simulink model "SIM_EXO_DAL_MN"  (R2021b)
(part 14 of 24)

C_dq = ft_12({dq1,dq2,dq3,dq4,dq5,dq6,t1004,t1016,t1019,t1020,t1031,t1039,t1046,t1050,t1056,t1061,t1069,t1075,t1076,t1077,t1081,t1083,t1088,t1090,t1095,t1099,t1101,t1106,t1108,t112,t1122,t113,t1133,t1144,t1146,t1147,t115,t1150,t1152,t1155,t1156,t1158,t116,t1165,t1170,t1171,t1174,t1177,t1179,t1184,t1185,t1191,t1193,t1194,t1196,t1201,t1203,t1205,t1207,t121,t1211,t1212,t1213,t1215,t1221,t1224,t1225,t1227,t1228,t1233,t1245,t125,t1250,t1253,t1254,t1258,t1265,t1267,t1268,t1269,t1273,t1274,t1282,t1285,t1288,t1292,t1300,t1301,t1306,t131,t1311,t1316,t1317,t1318,t132,t1322,t1323,t1324,t133,t1330,t1331,t1333,t1337,t1342,t1344,t1345,t1348,t1353,t1365,t1377,t1379,t1380,t1383,t1388,t139,t1391,t1402,t1407,t1409,t1411,t1413,t1419,t142,t1423,t1426,t1427,t1428,t1429,t1436,t144,t1440,t1441,t1443,t1445,t1446,t1449,t1454,t1457,t1458,t1460,t1471,t148,t1486,t1487,t1488,t1489,t1493,t1494,t1495,t1496,t1498,t1499,t15,t150,t1503,t1505,t1506,t1508,t151,t1511,t1517,t1520,t1521,t1522,t1523,t1524,t1526,t1530,t1531,t1533,t1534,t1535,t1536,t1537,t1538,t1540,t1541,t1542,t1548,t1549,t1550,t1551,t1558,t156,t1560,t1561,t1566,t1567,t1568,t1570,t1571,t1574,t1577,t1578,t158,t1581,t1582,t1584,t1585,t1586,t1587,t1589,t1590,t1591,t1592,t1593,t1594,t1595,t1598,t16,t1600,t1601,t1602,t1605,t1606,t1607,t1609,t1611,t1612,t1613,t1614,t1615,t1616,t1617,t1619,t1620,t1621,t1622,t1625,t1627,t1628,t1630,t1632,t1633,t1635,t1636,t1637,t1638,t1639,t1641,t1642,t1643,t1644,t1645,t1647,t1648,t1651,t1653,t1655,t1656,t1657,t1658,t1659,t166,t1660,t1661,t1662,t1663,t1666,t1667,t1669,t1670,t1672,t1674,t1676,t1681,t1683,t1687,t1692,t1696,t1697,t1699,t17,t1700,t1701,t1704,t1705,t1706,t1707,t1708,t1709,t171,t1710,t1711,t1712,t1713,t1715,t1716,t1718,t1719,t1720,t1721,t1724,t1728,t1729,t1731,t1732,t1733,t1734,t1735,t1736,t1740,t1745,t1747,t1748,t1752,t1753,t1754,t1755,t1756,t1757,t1758,t1759,t1760,t1761,t1762,t1763,t1764,t1766,t1767,t1769,t1770,t1771,t1772,t1775,t1776,t1777,t1779,t1781,t1783,t1784,t1785,t1786,t1787,t1788,t1789,t1792,t1793,t1794,t1795,t1797,t1798,t1799,t18,t1800,t1804,t1805,t1806,t1807,t1808,t1809,t1811,t1812,t1814,t1815,t1816,t1820,t1821,t1823,t1827,t1828,t1829,t183,t1831,t1832,t1833,t1834,t1835,t1836,t1839,t1847,t1849,t185,t1850,t1851,t1855,t1856,t1857,t1858,t1859,t1860,t1861,t1863,t1866,t1867,t1868,t1870,t1873,t1878,t1882,t1884,t1886,t1889,t1892,t1896,t1899,t19,t190,t1900,t1902,t1903,t1906,t1907,t1908,t1909,t191,t1912,t1913,t1915,t1916,t1917,t1920,t1922,t1925,t1926,t1930,t1935,t1936,t1937,t1938,t1939,t1941,t1942,t1943,t1946,t1947,t1951,t1952,t1955,t196,t1961,t1967,t1968,t1969,t197,t1970,t1974,t1977,t1981,t1983,t1984,t1985,t1986,t1989,t199,t1992,t1993,t1994,t1995,t1996,t1997,t1998,t1999,t2,t20,t200,t2000,t2002,t2003,t2004,t2006,t2008,t201,t2014,t2015,t2017,t2019,t202,t2020,t2026,t2027,t2028,t2033,t2034,t2035,t2036,t2037,t2038,t2039,t2042,t2043,t2047,t2050,t2052,t2053,t206,t2060,t2062,t2066,t2067,t2068,t2069,t207,t2070,t2072,t2073,t2075,t2076,t2077,t2079,t2081,t2083,t2084,t2085,t2087,t2088,t2091,t2096,t2098,t21,t2100,t2104,t2105,t2106,t2108,t2110,t2113,t2114,t2115,t2116,t2118,t2119,t2121,t2123,t2128,t2130,t2131,t2132,t2133,t2134,t2136,t2142,t2143,t2145,t2148,t2149,t2150,t2154,t2158,t2164,t2165,t2171,t2176,t2177,t2178,t2180,t2181,t2182,t2184,t2186,t2187,t2189,t2191,t2192,t2193,t2194,t2196,t2197,t2199,t22,t2200,t2202,t2203,t2208,t2211,t2212,t2213,t2214,t2217,t2218,t2220,t2223,t2224,t2225,t2234,t2236,t2239,t224,t2243,t225,t2253,t2256,t2257,t2265,t2266,t2267,t227,t2276,t2277,t2279,t228,t2280,t2284,t2285,t2289,t2291,t2296,t2298,t2299,t23,t230,t2300,t2303,t2304,t2305,t231,t2312,t2314,t2315,t2316,t2317,t2320,t2323,t2324,t2326,t2328,t233,t2330,t2333,t2334,t2336,t2338,t2339,t234,t2340,t2341,t2342,t235,t2350,t2357,t2358,t2359,t236,t2361,t2362,t2364,t2369,t2372,t2375,t2376,t2377,t2379,t2383,t2385,t2387,t2388,t2389,t2390,t2391,t2392,t2394,t2395,t2396,t2397,t2398,t24,t240,t2400,t2401,t2402,t2403,t2405,t2406,t2410,t2416,t2417,t2420,t2421,t2424,t2429,t243,t2430,t2431,t2435,t2438,t2439,t244,t2440,t2441,t2443,t2444,t2449,t2452,t2453,t2454,t2455,t2456,t2465,t2466,t2470,t2474,t2481,t2483,t2486,t249,t2490,t2494,t2497,t2502,t2507,t2513,t2519,t2523,t2524,t2525,t2530,t2539,t2544,t2545,t2546,t2548,t2549,t2552,t2553,t2554,t2555,t2556,t2560,t2562,t2563,t2564,t2565,t2566,t2567,t2568,t2569,t257,t2570,t2571,t2574,t2575,t2576,t2577,t2578,t2579,t258,t2588,t2589,t2597,t2598,t2599,t2606,t2611,t2612,t2615,t2617,t2620,t2623,t2624,t2625,t2627,t263,t2633,t2634,t2639,t2640,t2641,t2644,t2649,t2650,t2651,t2655,t2656,t2659,t266,t2666,t2669,t2671,t2673,t2675,t2681,t2684,t2686,t2689,t2691,t2692,t2694,t2695,t2696,t2697,t2698,t270,t2700,t2706,t2707,t2708,t2711,t2713,t2714,t2715,t2718,t2720,t2721,t2722,t2724,t2725,t2726,t273,t2736,t2737,t274,t2740,t2741,t2743,t2744,t2748,t2749,t275,t2750,t2752,t2753,t2754,t2755,t2757,t2758,t2759,t276,t2760,t2761,t2762,t2764,t277,t2770,t2771,t2772,t2775,t2778,t278,t2780,t2783,t2785,t2791,t2792,t2793,t2795,t2796,t2797,t2798,t2799,t280,t2800,t2801,t2802,t2805,t2806,t2807,t2812,t2814,t2815,t2816,t2817,t2818,t2824,t2825,t2827,t2828,t2832,t2833,t2835,t284,t2850,t2851,t2854,t2857,t2861,t2868,t287,t2872,t2877,t2880,t2881,t2883,t2884,t2887,t2889,t2893,t2895,t2896,t29,t290,t2905,t2906,t2907,t291,t2911,t2912,t2913,t2915,t2916,t2918,t292,t2921,t2922,t2932,t2933,t294,t2941,t2944,t2946,t2956,t2958,t2965,t297,t2973,t2977,t2987,t299,t2993,t2998,t2999,t3,t30,t300,t302,t303,t304,t3047,t305,t306,t3065,t3080,t3083,t3088,t309,t3095,t3096,t310,t311,t3117,t3125,t3129,t313,t3136,t314,t3142,t315,t3159,t316,t3164,t3166,t3168,t318,t319,t320,t3200,t3209,t3210,t3213,t3219,t322,t3222,t3223,t3224,t3228,t3230,t3239,t324,t3245,t3247,t325,t3266,t3268,t3274,t3275,t3277,t3278,t3279,t328,t3284,t3288,t3296,t3298,t3303,t3309,t3314,t3317,t3318,t3320,t3321,t3326,t3328,t3329,t333,t3332,t3336,t3337,t3338,t3340,t3349,t3351,t3352,t3353,t336,t3363,t3364,t3365,t3366,t3368,t3369,t337,t3371,t3372,t3373,t3375,t3377,t3378,t3380,t3381,t3383,t3387,t3388,t3390,t3391,t3392,t3393,t3396,t3397,t3398,t3399,t34,t340,t3400,t3402,t3405,t3407,t3408,t3409,t3410,t3411,t3413,t3416,t3417,t3418,t3420,t3421,t3422,t3426,t3429,t3430,t3432,t3434,t3435,t3436,t3437,t3439,t344,t3440,t3441,t3442,t3443,t3444,t3445,t3446,t3447,t3449,t3450,t3453,t3454,t3455,t3457,t3458,t346,t3462,t3463,t3464,t3465,t3468,t3469,t347,t3471,t3472,t3473,t3474,t3475,t3476,t3479,t348,t3480,t3481,t3483,t3484,t3485,t3489,t349,t3490,t3491,t3492,t3493,t3496,t3498,t3499,t350,t3500,t3501,t3502,t3504,t3505,t3506,t3507,t3510,t3511,t3513,t3514,t3515,t3517,t3518,t352,t3521,t3522,t3523,t3526,t353,t3530,t3531,t3532,t3535,t3536,t3539,t3540,t3542,t3543,t3544,t3547,t3554,t3556,t3557,t3559,t356,t3562,t3563,t3565,t3568,t3569,t357,t3571,t3572,t3573,t3574,t3577,t3578,t358,t3582,t3583,t3584,t3585,t3588,t3589,t359,t3590,t3591,t3592,t3593,t3598,t3602,t3604,t3605,t3606,t3607,t361,t3610,t3611,t3612,t3617,t3618,t362,t3624,t3625,t3633,t3634,t3635,t3636,t3637,t3638,t3640,t3642,t3644,t3648,t365,t3652,t3653,t3654,t3655,t3656,t3657,t3658,t3659,t3662,t3666,t3667,t3668,t3671,t3672,t3673,t3674,t3676,t3678,t3679,t368,t3681,t3682,t3689,t369,t3690,t3691,t3693,t3694,t3696,t3698,t3699,t3700,t3701,t3702,t3703,t3704,t3705,t3706,t3708,t371,t3713,t3715,t3717,t3719,t372,t3720,t3725,t3726,t3728,t3729,t373,t3731,t3732,t3733,t3734,t3735,t3737,t3738,t374,t3742,t3743,t3746,t3747,t3750,t3752,t3753,t3754,t3755,t3756,t3757,t3758,t3759,t3761,t3762,t3763,t3764,t3765,t3766,t3767,t3769,t377,t3772,t3777,t3779,t378,t3780,t3781,t3783,t3784,t3785,t3787,t3788,t3789,t379,t3792,t3793,t3795,t3796,t3799,t380,t3800,t3810,t3811,t3812,t3813,t3814,t3815,t3818,t3819,t382,t3820,t3821,t3822,t3823,t3824,t3831,t3833,t3834,t3835,t3836,t3838,t3839,t384,t3840,t3841,t3842,t3843,t3844,t3845,t3848,t3849,t3851,t3852,t3853,t386,t3863,t3865,t3866,t3868,t3869,t387,t3870,t3871,t3872,t3873,t3874,t3875,t3876,t388,t3880,t3882,t3883,t3884,t3885,t3889,t3890,t3891,t3892,t3893,t3896,t3904,t3905,t3906,t3907,t3908,t391,t3910,t3913,t3914,t3915,t392,t3920,t3921,t3922,t3923,t3924,t3931,t3940,t3941,t3942,t3943,t3944,t395,t3950,t3951,t3954,t3955,t3956,t3957,t3959,t396,t3960,t3965,t3967,t3968,t3969,t3971,t3972,t3973,t3976,t3977,t3978,t3979,t3991,t3992,t3993,t3995,t3996,t3997,t3998,t4,t400,t4000,t4004,t4008,t401,t4010,t4011,t4014,t4015,t4016,t4017,t4018,t402,t4020,t4023,t4024,t4025,t4026,t4028,t4029,t403,t4034,t4037,t4041,t4042,t4045,t4046,t4047,t4050,t4051,t4053,t4055,t4056,t4057,t4059,t406,t4062,t4063,t4064,t4067,t4068,t4069,t4070,t4071,t4072,t4073,t4074,t4075,t4076,t4079,t4080,t4083,t4085,t4086,t4087,t4088,t4089,t4091,t4092,t4093,t4094,t4095,t4096,t4099,t410,t4100,t4102,t4103,t4104,t4108,t411,t4113,t4115,t4118,t4119,t412,t4121,t4122,t4123,t4126,t4127,t413,t4132,t4134,t4138,t414,t4141,t4143,t4146,t4148,t4149,t415,t4152,t4153,t4154,t4158,t416,t4161,t4166,t417,t4173,t4178,t4179,t418,t4181,t4183,t4184,t4185,t4186,t4190,t4196,t4197,t4198,t4199,t420,t4205,t4206,t4208,t4209,t4210,t4211,t4215,t4217,t4218,t4219,t422,t4221,t4223,t4224,t4226,t4228,t423,t4230,t4231,t4232,t4233,t4234,t4235,t424,t4241,t4243,t4245,t4246,t4247,t4248,t4249,t425,t4250,t4251,t4254,t4255,t4256,t4257,t4259,t4260,t4261,t4262,t4263,t427,t4274,t4276,t4278,t4279,t428,t4280,t4282,t4283,t4284,t4285,t4286,t4287,t4289,t429,t4290,t4292,t4293,t4295,t4296,t4297,t4298,t4299,t4301,t4303,t4304,t4305,t4306,t431,t4315,t4317,t4318,t432,t4323,t4324,t4325,t4326,t4327,t4329,t433,t4330,t4332,t4333,t4334,t4335,t4337,t4338,t4339,t434,t4342,t4344,t4345,t4346,t4347,t4348,t4349,t435,t4350,t436,t4363,t4365,t4366,t4368,t4369,t437,t4370,t4371,t4373,t4374,t4377,t4378,t438,t4380,t4382,t4383,t4385,t4387,t4388,t439,t4392,t4394,t4395,t4396,t4397,t4399,t44,t440,t4402,t4403,t4405,t4406,t4407,t4409,t441,t4410,t4412,t4413,t4414,t4416,t4417,t4418,t4419,t442,t4420,t4421,t4423,t4425,t4426,t4427,t4428,t4429,t4431,t4432,t4433,t4434,t4435,t4436,t4437,t4438,t4439,t444,t4440,t4444,t4446,t4447,t4449,t445,t4450,t4453,t4460,t4462,t4463,t4464,t4467,t4468,t4469,t4470,t4471,t4473,t4474,t4475,t4478,t4479,t448,t4482,t4483,t4484,t4485,t4486,t4487,t4488,t4489,t449,t4490,t4494,t4495,t4498,t4499,t45,t450,t4500,t4501,t4502,t4503,t4504,t4505,t4506,t4507,t4508,t4509,t4510,t4512,t4515,t4518,t4519,t452,t4520,t4521,t4522,t4523,t4526,t4527,t4528,t453,t4530,t4534,t4536,t4538,t4539,t454,t4541,t4543,t4545,t4546,t4549,t4551,t4552,t4553,t4556,t4557,t4558,t4559,t4560,t4565,t4568,t4569,t457,t4570,t4572,t4575,t4577,t4578,t458,t4581,t4582,t4586,t4587,t4588,t4589,t459,t4590,t4591,t4592,t4593,t4595,t4596,t4597,t4598,t460,t4600,t4601,t4602,t4604,t4605,t4606,t4607,t4608,t461,t4614,t4616,t4619,t462,t4621,t4622,t4623,t4624,t4625,t4626,t4629,t463,t4633,t4634,t4636,t4637,t4639,t464,t4640,t4644,t4645,t4647,t4648,t465,t4650,t4652,t4653,t4654,t4656,t4657,t4659,t466,t4660,t4662,t4663,t4666,t4667,t4668,t4669,t4670,t4673,t4674,t4675,t4677,t4678,t4679,t468,t4680,t4681,t4682,t4683,t4684,t4685,t4686,t4687,t469,t4694,t4695,t4696,t4697,t4699,t47,t470,t4700,t4703,t4707,t4708,t4709,t471,t4711,t4714,t4717,t4718,t4719,t472,t4720,t4721,t4722,t4723,t4724,t4725,t4726,t4727,t4728,t4731,t4732,t4733,t4734,t4737,t4738,t4739,t4742,t4743,t4745,t4747,t4748,t475,t4754,t4755,t4756,t4762,t4763,t4764,t4767,t477,t4772,t4773,t4775,t4780,t4781,t4782,t4783,t4785,t4786,t479,t480,t4803,t481,t4810,t4811,t482,t4824,t4825,t4826,t483,t4831,t4837,t4838,t4842,t4846,t485,t486,t4862,t4864,t4865,t4866,t4867,t4869,t4870,t4877,t488,t4884,t489,t4903,t4904,t491,t4911,t4914,t4919,t492,t4920,t4922,t4924,t4925,t4927,t4929,t493,t4934,t4936,t494,t4942,t4944,t4946,t4949,t4950,t4952,t4953,t4957,t496,t4964,t4966,t4967,t4969,t497,t4973,t4974,t4979,t498,t4981,t4982,t4983,t4984,t4987,t4988,t4989,t499,t4990,t4993,t4994,t4995,t4996,t5,t50,t500,t5000,t5001,t5002,t5007,t5008,t5009,t501,t5016,t5017,t502,t5020,t5021,t5022,t5023,t5024,t5026,t5027,t503,t5031,t5032,t5039,t504,t5043,t5049,t505,t5050,t5056,t5058,t506,t5061,t5063,t5064,t5065,t507,t5074,t5075,t5076,t508,t5080,t5083,t5084,t5086,t5087,t509,t5090,t5091,t5092,t5093,t5097,t5098,t5099,t510,t5100,t5102,t5107,t511,t5110,t5112,t5113,t5114,t512,t5121,t5123,t513,t5131,t5132,t5136,t5139,t514,t5140,t5143,t5144,t5145,t5147,t5148,t5150,t5151,t516,t5163,t5164,t5166,t5167,t517,t5175,t5177,t518,t5182,t5184,t5188,t5189,t5194,t5195,t520,t5200,t5202,t5203,t5204,t5205,t5206,t521,t5210,t5211,t5215,t5217,t5219,t522,t5222,t5227,t5228,t523,t5231,t5232,t5233,t5235,t5236,t5237,t5238,t524,t5242,t5244,t5249,t525,t5251,t5252,t5254,t5255,t5256,t5258,t5259,t526,t5260,t5261,t5262,t5264,t5266,t5269,t527,t5275,t5279,t528,t5280,t5285,t5286,t529,t5291,t5294,t5296,t5297,t5299,t53,t530,t5301,t5302,t5307,t5309,t531,t5314,t5316,t5318,t532,t5320,t5321,t5322,t5323,t5324,t533,t5333,t5335,t5337,t5339,t534,t5340,t5344,t535,t5354,t5356,t5357,t5358,t5359,t536,t5361,t5364,t5369,t537,t5370,t5371,t5372,t5373,t5375,t5378,t5379,t538,t5380,t5381,t5382,t5383,t5385,t5389,t539,t5390,t5391,t5392,t5393,t5394,t5395,t5396,t5397,t5399,t540,t5401,t5402,t5403,t5404,t5405,t5406,t5408,t5409,t5410,t5411,t5412,t5414,t5415,t5416,t5418,t5422,t5423,t5426,t5427,t5428,t543,t5431,t5436,t5438,t544,t5442,t5443,t5447,t545,t5450,t5451,t5457,t5459,t546,t5464,t5465,t5466,t547,t5479,t548,t5480,t5482,t5483,t5484,t5486,t5487,t5488,t549,t5507,t551,t5512,t5515,t552,t5521,t5526,t553,t554,t555,t556,t557,t558,t559,t560,t5602,t5605,t561,t5616,t5617,t5619,t562,t5620,t5621,t5622,t5623,t5624,t5625,t5626,t5628,t563,t5630,t5633,t5634,t5636,t5639,t564,t5642,t5644,t5648,t5657,t5658,t5662,t5665,t5666,t567,t5670,t5679,t568,t5682,t5684,t5688,t569,t5691,t5692,t5694,t5696,t5698,t5699,t57,t570,t5701,t5703,t5704,t5705,t5707,t571,t5711,t5713,t5714,t5718,t572,t5720,t5722,t5723,t5724,t5726,t5727,t5728,t573,t5731,t5732,t5733,t5736,t5738,t574,t5742,t5745,t5746,t5747,t5748,t5751,t5754,t5757,t5759,t576,t5760,t5763,t5765,t5768,t5770,t5771,t5772,t5773,t5774,t5775,t5776,t5778,t5779,t578,t5782,t5784,t5786,t5787,t5788,t579,t5790,t5792,t5794,t5795,t5797,t58,t580,t5808,t5809,t581,t5810,t5813,t5814,t5818,t5819,t582,t5822,t5823,t5824,t5825,t5826,t5827,t5828,t5829,t5830,t5831,t5832,t5833,t5834,t5835,t5836,t5838,t584,t5842,t5843,t5844,t5845,t5846,t5849,t5850,t5851,t5852,t5859,t586,t5860,t5861,t5862,t5863,t5868,t5869,t587,t5870,t5871,t5872,t5873,t5874,t5875,t5876,t5881,t5882,t5883,t5884,t5885,t5886,t5887,t5888,t5889,t589,t5890,t5891,t5892,t5893,t5894,t5895,t5896,t5898,t5899,t590,t5901,t5902,t5903,t5905,t5906,t5909,t591,t5917,t5918,t5919,t592,t5920,t5925,t5928,t593,t5930,t5931,t5932,t5933,t5934,t5935,t5936,t5938,t5939,t594,t5940,t595,t5954,t5956,t5957,t5958,t5959,t596,t5960,t5964,t5965,t5966,t5967,t597,t5970,t5971,t5972,t5976,t5977,t5978,t5979,t5980,t5981,t5982,t5984,t5988,t5994,t5996,t5998,t5999,t6,t60,t600,t6000,t6001,t6002,t6003,t6005,t6007,t6011,t6012,t6013,t6014,t6017,t602,t603,t6038,t604,t6043,t6045,t6046,t6047,t605,t6060,t6061,t6062,t6064,t6065,t6069,t6075,t6077,t6079,t6086,t609,t610,t6101,t6102,t6103,t6105,t6106,t6108,t6109,t611,t6117,t6119,t612,t6123,t6124,t6126,t613,t6136,t6139,t614,t6140,t6149,t615,t616,t618,t619,t6195,t620,t6203,t6204,t6205,t6206,t6209,t621,t6210,t622,t623,t624,t625,t626,t629,t6319,t632,t6329,t6330,t6338,t6341,t6342,t6343,t6347,t6348,t6349,t6350,t6351,t6352,t6362,t638,t6391,t6395,t640,t6403,t6416,t6417,t6436,t6437,t6462,t6463,t6471,t650,t6506,t654,t6565,t658,t6597,t6609,t6689,t669,t6690,t673,t679,t681,t6826,t6827,t683,t684,t7,t7012,t7020,t7043,t705,t706,t7079,t708,t7080,t7087,t71,t7104,t7119,t712,t7148,t7149,t716,t72,t724,t7256,t73,t731,t733,t7333,t7364,t738,t739,t741,t742,t743,t744,t746,t748,t749,t75,t750,t752,t7528,t753,t7549,t7553,t7556,t7566,t7570,t7573,t759,t76,t760,t764,t765,t766,t773,t777,t778,t779,t780,t781,t784,t785,t792,t796,t797,t8,t801,t802,t803,t804,t81,t823,t824,t825,t826,t827,t830,t832,t833,t834,t835,t836,t838,t84,t841,t842,t843,t845,t846,t847,t848,t852,t856,t86,t861,t863,t866,t868,t869,t870,t874,t875,t877,t878,t880,t881,t893,t899,t9,t90,t902,t903,t905,t908,t909,t91,t910,t911,t912,t914,t915,t917,t919,t922,t925,t926,t928,t929,t930,t931,t932,t934,t940,t944,t945,t947,t95,t952,t954,t955,t957,t958,t968,t97,t970,t971,t972,t975,t976,t984,t985,t986,t989,t99,t991,t998});
end
function C_dq = ft_12(ct)
dq1 = ct{1};
dq2 = ct{2};
dq3 = ct{3};
dq4 = ct{4};
dq5 = ct{5};
dq6 = ct{6};
t1004 = ct{7};
t1016 = ct{8};
t1019 = ct{9};
t1020 = ct{10};
t1031 = ct{11};
t1039 = ct{12};
t1046 = ct{13};
t1050 = ct{14};
t1056 = ct{15};
t1061 = ct{16};
t1069 = ct{17};
t1075 = ct{18};
t1076 = ct{19};
t1077 = ct{20};
t1081 = ct{21};
t1083 = ct{22};
t1088 = ct{23};
t1090 = ct{24};
t1095 = ct{25};
t1099 = ct{26};
t1101 = ct{27};
t1106 = ct{28};
t1108 = ct{29};
t112 = ct{30};
t1122 = ct{31};
t113 = ct{32};
t1133 = ct{33};
t1144 = ct{34};
t1146 = ct{35};
t1147 = ct{36};
t115 = ct{37};
t1150 = ct{38};
t1152 = ct{39};
t1155 = ct{40};
t1156 = ct{41};
t1158 = ct{42};
t116 = ct{43};
t1165 = ct{44};
t1170 = ct{45};
t1171 = ct{46};
t1174 = ct{47};
t1177 = ct{48};
t1179 = ct{49};
t1184 = ct{50};
t1185 = ct{51};
t1191 = ct{52};
t1193 = ct{53};
t1194 = ct{54};
t1196 = ct{55};
t1201 = ct{56};
t1203 = ct{57};
t1205 = ct{58};
t1207 = ct{59};
t121 = ct{60};
t1211 = ct{61};
t1212 = ct{62};
t1213 = ct{63};
t1215 = ct{64};
t1221 = ct{65};
t1224 = ct{66};
t1225 = ct{67};
t1227 = ct{68};
t1228 = ct{69};
t1233 = ct{70};
t1245 = ct{71};
t125 = ct{72};
t1250 = ct{73};
t1253 = ct{74};
t1254 = ct{75};
t1258 = ct{76};
t1265 = ct{77};
t1267 = ct{78};
t1268 = ct{79};
t1269 = ct{80};
t1273 = ct{81};
t1274 = ct{82};
t1282 = ct{83};
t1285 = ct{84};
t1288 = ct{85};
t1292 = ct{86};
t1300 = ct{87};
t1301 = ct{88};
t1306 = ct{89};
t131 = ct{90};
t1311 = ct{91};
t1316 = ct{92};
t1317 = ct{93};
t1318 = ct{94};
t132 = ct{95};
t1322 = ct{96};
t1323 = ct{97};
t1324 = ct{98};
t133 = ct{99};
t1330 = ct{100};
t1331 = ct{101};
t1333 = ct{102};
t1337 = ct{103};
t1342 = ct{104};
t1344 = ct{105};
t1345 = ct{106};
t1348 = ct{107};
t1353 = ct{108};
t1365 = ct{109};
t1377 = ct{110};
t1379 = ct{111};
t1380 = ct{112};
t1383 = ct{113};
t1388 = ct{114};
t139 = ct{115};
t1391 = ct{116};
t1402 = ct{117};
t1407 = ct{118};
t1409 = ct{119};
t1411 = ct{120};
t1413 = ct{121};
t1419 = ct{122};
t142 = ct{123};
t1423 = ct{124};
t1426 = ct{125};
t1427 = ct{126};
t1428 = ct{127};
t1429 = ct{128};
t1436 = ct{129};
t144 = ct{130};
t1440 = ct{131};
t1441 = ct{132};
t1443 = ct{133};
t1445 = ct{134};
t1446 = ct{135};
t1449 = ct{136};
t1454 = ct{137};
t1457 = ct{138};
t1458 = ct{139};
t1460 = ct{140};
t1471 = ct{141};
t148 = ct{142};
t1486 = ct{143};
t1487 = ct{144};
t1488 = ct{145};
t1489 = ct{146};
t1493 = ct{147};
t1494 = ct{148};
t1495 = ct{149};
t1496 = ct{150};
t1498 = ct{151};
t1499 = ct{152};
t15 = ct{153};
t150 = ct{154};
t1503 = ct{155};
t1505 = ct{156};
t1506 = ct{157};
t1508 = ct{158};
t151 = ct{159};
t1511 = ct{160};
t1517 = ct{161};
t1520 = ct{162};
t1521 = ct{163};
t1522 = ct{164};
t1523 = ct{165};
t1524 = ct{166};
t1526 = ct{167};
t1530 = ct{168};
t1531 = ct{169};
t1533 = ct{170};
t1534 = ct{171};
t1535 = ct{172};
t1536 = ct{173};
t1537 = ct{174};
t1538 = ct{175};
t1540 = ct{176};
t1541 = ct{177};
t1542 = ct{178};
t1548 = ct{179};
t1549 = ct{180};
t1550 = ct{181};
t1551 = ct{182};
t1558 = ct{183};
t156 = ct{184};
t1560 = ct{185};
t1561 = ct{186};
t1566 = ct{187};
t1567 = ct{188};
t1568 = ct{189};
t1570 = ct{190};
t1571 = ct{191};
t1574 = ct{192};
t1577 = ct{193};
t1578 = ct{194};
t158 = ct{195};
t1581 = ct{196};
t1582 = ct{197};
t1584 = ct{198};
t1585 = ct{199};
t1586 = ct{200};
t1587 = ct{201};
t1589 = ct{202};
t1590 = ct{203};
t1591 = ct{204};
t1592 = ct{205};
t1593 = ct{206};
t1594 = ct{207};
t1595 = ct{208};
t1598 = ct{209};
t16 = ct{210};
t1600 = ct{211};
t1601 = ct{212};
t1602 = ct{213};
t1605 = ct{214};
t1606 = ct{215};
t1607 = ct{216};
t1609 = ct{217};
t1611 = ct{218};
t1612 = ct{219};
t1613 = ct{220};
t1614 = ct{221};
t1615 = ct{222};
t1616 = ct{223};
t1617 = ct{224};
t1619 = ct{225};
t1620 = ct{226};
t1621 = ct{227};
t1622 = ct{228};
t1625 = ct{229};
t1627 = ct{230};
t1628 = ct{231};
t1630 = ct{232};
t1632 = ct{233};
t1633 = ct{234};
t1635 = ct{235};
t1636 = ct{236};
t1637 = ct{237};
t1638 = ct{238};
t1639 = ct{239};
t1641 = ct{240};
t1642 = ct{241};
t1643 = ct{242};
t1644 = ct{243};
t1645 = ct{244};
t1647 = ct{245};
t1648 = ct{246};
t1651 = ct{247};
t1653 = ct{248};
t1655 = ct{249};
t1656 = ct{250};
t1657 = ct{251};
t1658 = ct{252};
t1659 = ct{253};
t166 = ct{254};
t1660 = ct{255};
t1661 = ct{256};
t1662 = ct{257};
t1663 = ct{258};
t1666 = ct{259};
t1667 = ct{260};
t1669 = ct{261};
t1670 = ct{262};
t1672 = ct{263};
t1674 = ct{264};
t1676 = ct{265};
t1681 = ct{266};
t1683 = ct{267};
t1687 = ct{268};
t1692 = ct{269};
t1696 = ct{270};
t1697 = ct{271};
t1699 = ct{272};
t17 = ct{273};
t1700 = ct{274};
t1701 = ct{275};
t1704 = ct{276};
t1705 = ct{277};
t1706 = ct{278};
t1707 = ct{279};
t1708 = ct{280};
t1709 = ct{281};
t171 = ct{282};
t1710 = ct{283};
t1711 = ct{284};
t1712 = ct{285};
t1713 = ct{286};
t1715 = ct{287};
t1716 = ct{288};
t1718 = ct{289};
t1719 = ct{290};
t1720 = ct{291};
t1721 = ct{292};
t1724 = ct{293};
t1728 = ct{294};
t1729 = ct{295};
t1731 = ct{296};
t1732 = ct{297};
t1733 = ct{298};
t1734 = ct{299};
t1735 = ct{300};
t1736 = ct{301};
t1740 = ct{302};
t1745 = ct{303};
t1747 = ct{304};
t1748 = ct{305};
t1752 = ct{306};
t1753 = ct{307};
t1754 = ct{308};
t1755 = ct{309};
t1756 = ct{310};
t1757 = ct{311};
t1758 = ct{312};
t1759 = ct{313};
t1760 = ct{314};
t1761 = ct{315};
t1762 = ct{316};
t1763 = ct{317};
t1764 = ct{318};
t1766 = ct{319};
t1767 = ct{320};
t1769 = ct{321};
t1770 = ct{322};
t1771 = ct{323};
t1772 = ct{324};
t1775 = ct{325};
t1776 = ct{326};
t1777 = ct{327};
t1779 = ct{328};
t1781 = ct{329};
t1783 = ct{330};
t1784 = ct{331};
t1785 = ct{332};
t1786 = ct{333};
t1787 = ct{334};
t1788 = ct{335};
t1789 = ct{336};
t1792 = ct{337};
t1793 = ct{338};
t1794 = ct{339};
t1795 = ct{340};
t1797 = ct{341};
t1798 = ct{342};
t1799 = ct{343};
t18 = ct{344};
t1800 = ct{345};
t1804 = ct{346};
t1805 = ct{347};
t1806 = ct{348};
t1807 = ct{349};
t1808 = ct{350};
t1809 = ct{351};
t1811 = ct{352};
t1812 = ct{353};
t1814 = ct{354};
t1815 = ct{355};
t1816 = ct{356};
t1820 = ct{357};
t1821 = ct{358};
t1823 = ct{359};
t1827 = ct{360};
t1828 = ct{361};
t1829 = ct{362};
t183 = ct{363};
t1831 = ct{364};
t1832 = ct{365};
t1833 = ct{366};
t1834 = ct{367};
t1835 = ct{368};
t1836 = ct{369};
t1839 = ct{370};
t1847 = ct{371};
t1849 = ct{372};
t185 = ct{373};
t1850 = ct{374};
t1851 = ct{375};
t1855 = ct{376};
t1856 = ct{377};
t1857 = ct{378};
t1858 = ct{379};
t1859 = ct{380};
t1860 = ct{381};
t1861 = ct{382};
t1863 = ct{383};
t1866 = ct{384};
t1867 = ct{385};
t1868 = ct{386};
t1870 = ct{387};
t1873 = ct{388};
t1878 = ct{389};
t1882 = ct{390};
t1884 = ct{391};
t1886 = ct{392};
t1889 = ct{393};
t1892 = ct{394};
t1896 = ct{395};
t1899 = ct{396};
t19 = ct{397};
t190 = ct{398};
t1900 = ct{399};
t1902 = ct{400};
t1903 = ct{401};
t1906 = ct{402};
t1907 = ct{403};
t1908 = ct{404};
t1909 = ct{405};
t191 = ct{406};
t1912 = ct{407};
t1913 = ct{408};
t1915 = ct{409};
t1916 = ct{410};
t1917 = ct{411};
t1920 = ct{412};
t1922 = ct{413};
t1925 = ct{414};
t1926 = ct{415};
t1930 = ct{416};
t1935 = ct{417};
t1936 = ct{418};
t1937 = ct{419};
t1938 = ct{420};
t1939 = ct{421};
t1941 = ct{422};
t1942 = ct{423};
t1943 = ct{424};
t1946 = ct{425};
t1947 = ct{426};
t1951 = ct{427};
t1952 = ct{428};
t1955 = ct{429};
t196 = ct{430};
t1961 = ct{431};
t1967 = ct{432};
t1968 = ct{433};
t1969 = ct{434};
t197 = ct{435};
t1970 = ct{436};
t1974 = ct{437};
t1977 = ct{438};
t1981 = ct{439};
t1983 = ct{440};
t1984 = ct{441};
t1985 = ct{442};
t1986 = ct{443};
t1989 = ct{444};
t199 = ct{445};
t1992 = ct{446};
t1993 = ct{447};
t1994 = ct{448};
t1995 = ct{449};
t1996 = ct{450};
t1997 = ct{451};
t1998 = ct{452};
t1999 = ct{453};
t2 = ct{454};
t20 = ct{455};
t200 = ct{456};
t2000 = ct{457};
t2002 = ct{458};
t2003 = ct{459};
t2004 = ct{460};
t2006 = ct{461};
t2008 = ct{462};
t201 = ct{463};
t2014 = ct{464};
t2015 = ct{465};
t2017 = ct{466};
t2019 = ct{467};
t202 = ct{468};
t2020 = ct{469};
t2026 = ct{470};
t2027 = ct{471};
t2028 = ct{472};
t2033 = ct{473};
t2034 = ct{474};
t2035 = ct{475};
t2036 = ct{476};
t2037 = ct{477};
t2038 = ct{478};
t2039 = ct{479};
t2042 = ct{480};
t2043 = ct{481};
t2047 = ct{482};
t2050 = ct{483};
t2052 = ct{484};
t2053 = ct{485};
t206 = ct{486};
t2060 = ct{487};
t2062 = ct{488};
t2066 = ct{489};
t2067 = ct{490};
t2068 = ct{491};
t2069 = ct{492};
t207 = ct{493};
t2070 = ct{494};
t2072 = ct{495};
t2073 = ct{496};
t2075 = ct{497};
t2076 = ct{498};
t2077 = ct{499};
t2079 = ct{500};
t2081 = ct{501};
t2083 = ct{502};
t2084 = ct{503};
t2085 = ct{504};
t2087 = ct{505};
t2088 = ct{506};
t2091 = ct{507};
t2096 = ct{508};
t2098 = ct{509};
t21 = ct{510};
t2100 = ct{511};
t2104 = ct{512};
t2105 = ct{513};
t2106 = ct{514};
t2108 = ct{515};
t2110 = ct{516};
t2113 = ct{517};
t2114 = ct{518};
t2115 = ct{519};
t2116 = ct{520};
t2118 = ct{521};
t2119 = ct{522};
t2121 = ct{523};
t2123 = ct{524};
t2128 = ct{525};
t2130 = ct{526};
t2131 = ct{527};
t2132 = ct{528};
t2133 = ct{529};
t2134 = ct{530};
t2136 = ct{531};
t2142 = ct{532};
t2143 = ct{533};
t2145 = ct{534};
t2148 = ct{535};
t2149 = ct{536};
t2150 = ct{537};
t2154 = ct{538};
t2158 = ct{539};
t2164 = ct{540};
t2165 = ct{541};
t2171 = ct{542};
t2176 = ct{543};
t2177 = ct{544};
t2178 = ct{545};
t2180 = ct{546};
t2181 = ct{547};
t2182 = ct{548};
t2184 = ct{549};
t2186 = ct{550};
t2187 = ct{551};
t2189 = ct{552};
t2191 = ct{553};
t2192 = ct{554};
t2193 = ct{555};
t2194 = ct{556};
t2196 = ct{557};
t2197 = ct{558};
t2199 = ct{559};
t22 = ct{560};
t2200 = ct{561};
t2202 = ct{562};
t2203 = ct{563};
t2208 = ct{564};
t2211 = ct{565};
t2212 = ct{566};
t2213 = ct{567};
t2214 = ct{568};
t2217 = ct{569};
t2218 = ct{570};
t2220 = ct{571};
t2223 = ct{572};
t2224 = ct{573};
t2225 = ct{574};
t2234 = ct{575};
t2236 = ct{576};
t2239 = ct{577};
t224 = ct{578};
t2243 = ct{579};
t225 = ct{580};
t2253 = ct{581};
t2256 = ct{582};
t2257 = ct{583};
t2265 = ct{584};
t2266 = ct{585};
t2267 = ct{586};
t227 = ct{587};
t2276 = ct{588};
t2277 = ct{589};
t2279 = ct{590};
t228 = ct{591};
t2280 = ct{592};
t2284 = ct{593};
t2285 = ct{594};
t2289 = ct{595};
t2291 = ct{596};
t2296 = ct{597};
t2298 = ct{598};
t2299 = ct{599};
t23 = ct{600};
t230 = ct{601};
t2300 = ct{602};
t2303 = ct{603};
t2304 = ct{604};
t2305 = ct{605};
t231 = ct{606};
t2312 = ct{607};
t2314 = ct{608};
t2315 = ct{609};
t2316 = ct{610};
t2317 = ct{611};
t2320 = ct{612};
t2323 = ct{613};
t2324 = ct{614};
t2326 = ct{615};
t2328 = ct{616};
t233 = ct{617};
t2330 = ct{618};
t2333 = ct{619};
t2334 = ct{620};
t2336 = ct{621};
t2338 = ct{622};
t2339 = ct{623};
t234 = ct{624};
t2340 = ct{625};
t2341 = ct{626};
t2342 = ct{627};
t235 = ct{628};
t2350 = ct{629};
t2357 = ct{630};
t2358 = ct{631};
t2359 = ct{632};
t236 = ct{633};
t2361 = ct{634};
t2362 = ct{635};
t2364 = ct{636};
t2369 = ct{637};
t2372 = ct{638};
t2375 = ct{639};
t2376 = ct{640};
t2377 = ct{641};
t2379 = ct{642};
t2383 = ct{643};
t2385 = ct{644};
t2387 = ct{645};
t2388 = ct{646};
t2389 = ct{647};
t2390 = ct{648};
t2391 = ct{649};
t2392 = ct{650};
t2394 = ct{651};
t2395 = ct{652};
t2396 = ct{653};
t2397 = ct{654};
t2398 = ct{655};
t24 = ct{656};
t240 = ct{657};
t2400 = ct{658};
t2401 = ct{659};
t2402 = ct{660};
t2403 = ct{661};
t2405 = ct{662};
t2406 = ct{663};
t2410 = ct{664};
t2416 = ct{665};
t2417 = ct{666};
t2420 = ct{667};
t2421 = ct{668};
t2424 = ct{669};
t2429 = ct{670};
t243 = ct{671};
t2430 = ct{672};
t2431 = ct{673};
t2435 = ct{674};
t2438 = ct{675};
t2439 = ct{676};
t244 = ct{677};
t2440 = ct{678};
t2441 = ct{679};
t2443 = ct{680};
t2444 = ct{681};
t2449 = ct{682};
t2452 = ct{683};
t2453 = ct{684};
t2454 = ct{685};
t2455 = ct{686};
t2456 = ct{687};
t2465 = ct{688};
t2466 = ct{689};
t2470 = ct{690};
t2474 = ct{691};
t2481 = ct{692};
t2483 = ct{693};
t2486 = ct{694};
t249 = ct{695};
t2490 = ct{696};
t2494 = ct{697};
t2497 = ct{698};
t2502 = ct{699};
t2507 = ct{700};
t2513 = ct{701};
t2519 = ct{702};
t2523 = ct{703};
t2524 = ct{704};
t2525 = ct{705};
t2530 = ct{706};
t2539 = ct{707};
t2544 = ct{708};
t2545 = ct{709};
t2546 = ct{710};
t2548 = ct{711};
t2549 = ct{712};
t2552 = ct{713};
t2553 = ct{714};
t2554 = ct{715};
t2555 = ct{716};
t2556 = ct{717};
t2560 = ct{718};
t2562 = ct{719};
t2563 = ct{720};
t2564 = ct{721};
t2565 = ct{722};
t2566 = ct{723};
t2567 = ct{724};
t2568 = ct{725};
t2569 = ct{726};
t257 = ct{727};
t2570 = ct{728};
t2571 = ct{729};
t2574 = ct{730};
t2575 = ct{731};
t2576 = ct{732};
t2577 = ct{733};
t2578 = ct{734};
t2579 = ct{735};
t258 = ct{736};
t2588 = ct{737};
t2589 = ct{738};
t2597 = ct{739};
t2598 = ct{740};
t2599 = ct{741};
t2606 = ct{742};
t2611 = ct{743};
t2612 = ct{744};
t2615 = ct{745};
t2617 = ct{746};
t2620 = ct{747};
t2623 = ct{748};
t2624 = ct{749};
t2625 = ct{750};
t2627 = ct{751};
t263 = ct{752};
t2633 = ct{753};
t2634 = ct{754};
t2639 = ct{755};
t2640 = ct{756};
t2641 = ct{757};
t2644 = ct{758};
t2649 = ct{759};
t2650 = ct{760};
t2651 = ct{761};
t2655 = ct{762};
t2656 = ct{763};
t2659 = ct{764};
t266 = ct{765};
t2666 = ct{766};
t2669 = ct{767};
t2671 = ct{768};
t2673 = ct{769};
t2675 = ct{770};
t2681 = ct{771};
t2684 = ct{772};
t2686 = ct{773};
t2689 = ct{774};
t2691 = ct{775};
t2692 = ct{776};
t2694 = ct{777};
t2695 = ct{778};
t2696 = ct{779};
t2697 = ct{780};
t2698 = ct{781};
t270 = ct{782};
t2700 = ct{783};
t2706 = ct{784};
t2707 = ct{785};
t2708 = ct{786};
t2711 = ct{787};
t2713 = ct{788};
t2714 = ct{789};
t2715 = ct{790};
t2718 = ct{791};
t2720 = ct{792};
t2721 = ct{793};
t2722 = ct{794};
t2724 = ct{795};
t2725 = ct{796};
t2726 = ct{797};
t273 = ct{798};
t2736 = ct{799};
t2737 = ct{800};
t274 = ct{801};
t2740 = ct{802};
t2741 = ct{803};
t2743 = ct{804};
t2744 = ct{805};
t2748 = ct{806};
t2749 = ct{807};
t275 = ct{808};
t2750 = ct{809};
t2752 = ct{810};
t2753 = ct{811};
t2754 = ct{812};
t2755 = ct{813};
t2757 = ct{814};
t2758 = ct{815};
t2759 = ct{816};
t276 = ct{817};
t2760 = ct{818};
t2761 = ct{819};
t2762 = ct{820};
t2764 = ct{821};
t277 = ct{822};
t2770 = ct{823};
t2771 = ct{824};
t2772 = ct{825};
t2775 = ct{826};
t2778 = ct{827};
t278 = ct{828};
t2780 = ct{829};
t2783 = ct{830};
t2785 = ct{831};
t2791 = ct{832};
t2792 = ct{833};
t2793 = ct{834};
t2795 = ct{835};
t2796 = ct{836};
t2797 = ct{837};
t2798 = ct{838};
t2799 = ct{839};
t280 = ct{840};
t2800 = ct{841};
t2801 = ct{842};
t2802 = ct{843};
t2805 = ct{844};
t2806 = ct{845};
t2807 = ct{846};
t2812 = ct{847};
t2814 = ct{848};
t2815 = ct{849};
t2816 = ct{850};
t2817 = ct{851};
t2818 = ct{852};
t2824 = ct{853};
t2825 = ct{854};
t2827 = ct{855};
t2828 = ct{856};
t2832 = ct{857};
t2833 = ct{858};
t2835 = ct{859};
t284 = ct{860};
t2850 = ct{861};
t2851 = ct{862};
t2854 = ct{863};
t2857 = ct{864};
t2861 = ct{865};
t2868 = ct{866};
t287 = ct{867};
t2872 = ct{868};
t2877 = ct{869};
t2880 = ct{870};
t2881 = ct{871};
t2883 = ct{872};
t2884 = ct{873};
t2887 = ct{874};
t2889 = ct{875};
t2893 = ct{876};
t2895 = ct{877};
t2896 = ct{878};
t29 = ct{879};
t290 = ct{880};
t2905 = ct{881};
t2906 = ct{882};
t2907 = ct{883};
t291 = ct{884};
t2911 = ct{885};
t2912 = ct{886};
t2913 = ct{887};
t2915 = ct{888};
t2916 = ct{889};
t2918 = ct{890};
t292 = ct{891};
t2921 = ct{892};
t2922 = ct{893};
t2932 = ct{894};
t2933 = ct{895};
t294 = ct{896};
t2941 = ct{897};
t2944 = ct{898};
t2946 = ct{899};
t2956 = ct{900};
t2958 = ct{901};
t2965 = ct{902};
t297 = ct{903};
t2973 = ct{904};
t2977 = ct{905};
t2987 = ct{906};
t299 = ct{907};
t2993 = ct{908};
t2998 = ct{909};
t2999 = ct{910};
t3 = ct{911};
t30 = ct{912};
t300 = ct{913};
t302 = ct{914};
t303 = ct{915};
t304 = ct{916};
t3047 = ct{917};
t305 = ct{918};
t306 = ct{919};
t3065 = ct{920};
t3080 = ct{921};
t3083 = ct{922};
t3088 = ct{923};
t309 = ct{924};
t3095 = ct{925};
t3096 = ct{926};
t310 = ct{927};
t311 = ct{928};
t3117 = ct{929};
t3125 = ct{930};
t3129 = ct{931};
t313 = ct{932};
t3136 = ct{933};
t314 = ct{934};
t3142 = ct{935};
t315 = ct{936};
t3159 = ct{937};
t316 = ct{938};
t3164 = ct{939};
t3166 = ct{940};
t3168 = ct{941};
t318 = ct{942};
t319 = ct{943};
t320 = ct{944};
t3200 = ct{945};
t3209 = ct{946};
t3210 = ct{947};
t3213 = ct{948};
t3219 = ct{949};
t322 = ct{950};
t3222 = ct{951};
t3223 = ct{952};
t3224 = ct{953};
t3228 = ct{954};
t3230 = ct{955};
t3239 = ct{956};
t324 = ct{957};
t3245 = ct{958};
t3247 = ct{959};
t325 = ct{960};
t3266 = ct{961};
t3268 = ct{962};
t3274 = ct{963};
t3275 = ct{964};
t3277 = ct{965};
t3278 = ct{966};
t3279 = ct{967};
t328 = ct{968};
t3284 = ct{969};
t3288 = ct{970};
t3296 = ct{971};
t3298 = ct{972};
t3303 = ct{973};
t3309 = ct{974};
t3314 = ct{975};
t3317 = ct{976};
t3318 = ct{977};
t3320 = ct{978};
t3321 = ct{979};
t3326 = ct{980};
t3328 = ct{981};
t3329 = ct{982};
t333 = ct{983};
t3332 = ct{984};
t3336 = ct{985};
t3337 = ct{986};
t3338 = ct{987};
t3340 = ct{988};
t3349 = ct{989};
t3351 = ct{990};
t3352 = ct{991};
t3353 = ct{992};
t336 = ct{993};
t3363 = ct{994};
t3364 = ct{995};
t3365 = ct{996};
t3366 = ct{997};
t3368 = ct{998};
t3369 = ct{999};
t337 = ct{1000};
t3371 = ct{1001};
t3372 = ct{1002};
t3373 = ct{1003};
t3375 = ct{1004};
t3377 = ct{1005};
t3378 = ct{1006};
t3380 = ct{1007};
t3381 = ct{1008};
t3383 = ct{1009};
t3387 = ct{1010};
t3388 = ct{1011};
t3390 = ct{1012};
t3391 = ct{1013};
t3392 = ct{1014};
t3393 = ct{1015};
t3396 = ct{1016};
t3397 = ct{1017};
t3398 = ct{1018};
t3399 = ct{1019};
t34 = ct{1020};
t340 = ct{1021};
t3400 = ct{1022};
t3402 = ct{1023};
t3405 = ct{1024};
t3407 = ct{1025};
t3408 = ct{1026};
t3409 = ct{1027};
t3410 = ct{1028};
t3411 = ct{1029};
t3413 = ct{1030};
t3416 = ct{1031};
t3417 = ct{1032};
t3418 = ct{1033};
t3420 = ct{1034};
t3421 = ct{1035};
t3422 = ct{1036};
t3426 = ct{1037};
t3429 = ct{1038};
t3430 = ct{1039};
t3432 = ct{1040};
t3434 = ct{1041};
t3435 = ct{1042};
t3436 = ct{1043};
t3437 = ct{1044};
t3439 = ct{1045};
t344 = ct{1046};
t3440 = ct{1047};
t3441 = ct{1048};
t3442 = ct{1049};
t3443 = ct{1050};
t3444 = ct{1051};
t3445 = ct{1052};
t3446 = ct{1053};
t3447 = ct{1054};
t3449 = ct{1055};
t3450 = ct{1056};
t3453 = ct{1057};
t3454 = ct{1058};
t3455 = ct{1059};
t3457 = ct{1060};
t3458 = ct{1061};
t346 = ct{1062};
t3462 = ct{1063};
t3463 = ct{1064};
t3464 = ct{1065};
t3465 = ct{1066};
t3468 = ct{1067};
t3469 = ct{1068};
t347 = ct{1069};
t3471 = ct{1070};
t3472 = ct{1071};
t3473 = ct{1072};
t3474 = ct{1073};
t3475 = ct{1074};
t3476 = ct{1075};
t3479 = ct{1076};
t348 = ct{1077};
t3480 = ct{1078};
t3481 = ct{1079};
t3483 = ct{1080};
t3484 = ct{1081};
t3485 = ct{1082};
t3489 = ct{1083};
t349 = ct{1084};
t3490 = ct{1085};
t3491 = ct{1086};
t3492 = ct{1087};
t3493 = ct{1088};
t3496 = ct{1089};
t3498 = ct{1090};
t3499 = ct{1091};
t350 = ct{1092};
t3500 = ct{1093};
t3501 = ct{1094};
t3502 = ct{1095};
t3504 = ct{1096};
t3505 = ct{1097};
t3506 = ct{1098};
t3507 = ct{1099};
t3510 = ct{1100};
t3511 = ct{1101};
t3513 = ct{1102};
t3514 = ct{1103};
t3515 = ct{1104};
t3517 = ct{1105};
t3518 = ct{1106};
t352 = ct{1107};
t3521 = ct{1108};
t3522 = ct{1109};
t3523 = ct{1110};
t3526 = ct{1111};
t353 = ct{1112};
t3530 = ct{1113};
t3531 = ct{1114};
t3532 = ct{1115};
t3535 = ct{1116};
t3536 = ct{1117};
t3539 = ct{1118};
t3540 = ct{1119};
t3542 = ct{1120};
t3543 = ct{1121};
t3544 = ct{1122};
t3547 = ct{1123};
t3554 = ct{1124};
t3556 = ct{1125};
t3557 = ct{1126};
t3559 = ct{1127};
t356 = ct{1128};
t3562 = ct{1129};
t3563 = ct{1130};
t3565 = ct{1131};
t3568 = ct{1132};
t3569 = ct{1133};
t357 = ct{1134};
t3571 = ct{1135};
t3572 = ct{1136};
t3573 = ct{1137};
t3574 = ct{1138};
t3577 = ct{1139};
t3578 = ct{1140};
t358 = ct{1141};
t3582 = ct{1142};
t3583 = ct{1143};
t3584 = ct{1144};
t3585 = ct{1145};
t3588 = ct{1146};
t3589 = ct{1147};
t359 = ct{1148};
t3590 = ct{1149};
t3591 = ct{1150};
t3592 = ct{1151};
t3593 = ct{1152};
t3598 = ct{1153};
t3602 = ct{1154};
t3604 = ct{1155};
t3605 = ct{1156};
t3606 = ct{1157};
t3607 = ct{1158};
t361 = ct{1159};
t3610 = ct{1160};
t3611 = ct{1161};
t3612 = ct{1162};
t3617 = ct{1163};
t3618 = ct{1164};
t362 = ct{1165};
t3624 = ct{1166};
t3625 = ct{1167};
t3633 = ct{1168};
t3634 = ct{1169};
t3635 = ct{1170};
t3636 = ct{1171};
t3637 = ct{1172};
t3638 = ct{1173};
t3640 = ct{1174};
t3642 = ct{1175};
t3644 = ct{1176};
t3648 = ct{1177};
t365 = ct{1178};
t3652 = ct{1179};
t3653 = ct{1180};
t3654 = ct{1181};
t3655 = ct{1182};
t3656 = ct{1183};
t3657 = ct{1184};
t3658 = ct{1185};
t3659 = ct{1186};
t3662 = ct{1187};
t3666 = ct{1188};
t3667 = ct{1189};
t3668 = ct{1190};
t3671 = ct{1191};
t3672 = ct{1192};
t3673 = ct{1193};
t3674 = ct{1194};
t3676 = ct{1195};
t3678 = ct{1196};
t3679 = ct{1197};
t368 = ct{1198};
t3681 = ct{1199};
t3682 = ct{1200};
t3689 = ct{1201};
t369 = ct{1202};
t3690 = ct{1203};
t3691 = ct{1204};
t3693 = ct{1205};
t3694 = ct{1206};
t3696 = ct{1207};
t3698 = ct{1208};
t3699 = ct{1209};
t3700 = ct{1210};
t3701 = ct{1211};
t3702 = ct{1212};
t3703 = ct{1213};
t3704 = ct{1214};
t3705 = ct{1215};
t3706 = ct{1216};
t3708 = ct{1217};
t371 = ct{1218};
t3713 = ct{1219};
t3715 = ct{1220};
t3717 = ct{1221};
t3719 = ct{1222};
t372 = ct{1223};
t3720 = ct{1224};
t3725 = ct{1225};
t3726 = ct{1226};
t3728 = ct{1227};
t3729 = ct{1228};
t373 = ct{1229};
t3731 = ct{1230};
t3732 = ct{1231};
t3733 = ct{1232};
t3734 = ct{1233};
t3735 = ct{1234};
t3737 = ct{1235};
t3738 = ct{1236};
t374 = ct{1237};
t3742 = ct{1238};
t3743 = ct{1239};
t3746 = ct{1240};
t3747 = ct{1241};
t3750 = ct{1242};
t3752 = ct{1243};
t3753 = ct{1244};
t3754 = ct{1245};
t3755 = ct{1246};
t3756 = ct{1247};
t3757 = ct{1248};
t3758 = ct{1249};
t3759 = ct{1250};
t3761 = ct{1251};
t3762 = ct{1252};
t3763 = ct{1253};
t3764 = ct{1254};
t3765 = ct{1255};
t3766 = ct{1256};
t3767 = ct{1257};
t3769 = ct{1258};
t377 = ct{1259};
t3772 = ct{1260};
t3777 = ct{1261};
t3779 = ct{1262};
t378 = ct{1263};
t3780 = ct{1264};
t3781 = ct{1265};
t3783 = ct{1266};
t3784 = ct{1267};
t3785 = ct{1268};
t3787 = ct{1269};
t3788 = ct{1270};
t3789 = ct{1271};
t379 = ct{1272};
t3792 = ct{1273};
t3793 = ct{1274};
t3795 = ct{1275};
t3796 = ct{1276};
t3799 = ct{1277};
t380 = ct{1278};
t3800 = ct{1279};
t3810 = ct{1280};
t3811 = ct{1281};
t3812 = ct{1282};
t3813 = ct{1283};
t3814 = ct{1284};
t3815 = ct{1285};
t3818 = ct{1286};
t3819 = ct{1287};
t382 = ct{1288};
t3820 = ct{1289};
t3821 = ct{1290};
t3822 = ct{1291};
t3823 = ct{1292};
t3824 = ct{1293};
t3831 = ct{1294};
t3833 = ct{1295};
t3834 = ct{1296};
t3835 = ct{1297};
t3836 = ct{1298};
t3838 = ct{1299};
t3839 = ct{1300};
t384 = ct{1301};
t3840 = ct{1302};
t3841 = ct{1303};
t3842 = ct{1304};
t3843 = ct{1305};
t3844 = ct{1306};
t3845 = ct{1307};
t3848 = ct{1308};
t3849 = ct{1309};
t3851 = ct{1310};
t3852 = ct{1311};
t3853 = ct{1312};
t386 = ct{1313};
t3863 = ct{1314};
t3865 = ct{1315};
t3866 = ct{1316};
t3868 = ct{1317};
t3869 = ct{1318};
t387 = ct{1319};
t3870 = ct{1320};
t3871 = ct{1321};
t3872 = ct{1322};
t3873 = ct{1323};
t3874 = ct{1324};
t3875 = ct{1325};
t3876 = ct{1326};
t388 = ct{1327};
t3880 = ct{1328};
t3882 = ct{1329};
t3883 = ct{1330};
t3884 = ct{1331};
t3885 = ct{1332};
t3889 = ct{1333};
t3890 = ct{1334};
t3891 = ct{1335};
t3892 = ct{1336};
t3893 = ct{1337};
t3896 = ct{1338};
t3904 = ct{1339};
t3905 = ct{1340};
t3906 = ct{1341};
t3907 = ct{1342};
t3908 = ct{1343};
t391 = ct{1344};
t3910 = ct{1345};
t3913 = ct{1346};
t3914 = ct{1347};
t3915 = ct{1348};
t392 = ct{1349};
t3920 = ct{1350};
t3921 = ct{1351};
t3922 = ct{1352};
t3923 = ct{1353};
t3924 = ct{1354};
t3931 = ct{1355};
t3940 = ct{1356};
t3941 = ct{1357};
t3942 = ct{1358};
t3943 = ct{1359};
t3944 = ct{1360};
t395 = ct{1361};
t3950 = ct{1362};
t3951 = ct{1363};
t3954 = ct{1364};
t3955 = ct{1365};
t3956 = ct{1366};
t3957 = ct{1367};
t3959 = ct{1368};
t396 = ct{1369};
t3960 = ct{1370};
t3965 = ct{1371};
t3967 = ct{1372};
t3968 = ct{1373};
t3969 = ct{1374};
t3971 = ct{1375};
t3972 = ct{1376};
t3973 = ct{1377};
t3976 = ct{1378};
t3977 = ct{1379};
t3978 = ct{1380};
t3979 = ct{1381};
t3991 = ct{1382};
t3992 = ct{1383};
t3993 = ct{1384};
t3995 = ct{1385};
t3996 = ct{1386};
t3997 = ct{1387};
t3998 = ct{1388};
t4 = ct{1389};
t400 = ct{1390};
t4000 = ct{1391};
t4004 = ct{1392};
t4008 = ct{1393};
t401 = ct{1394};
t4010 = ct{1395};
t4011 = ct{1396};
t4014 = ct{1397};
t4015 = ct{1398};
t4016 = ct{1399};
t4017 = ct{1400};
t4018 = ct{1401};
t402 = ct{1402};
t4020 = ct{1403};
t4023 = ct{1404};
t4024 = ct{1405};
t4025 = ct{1406};
t4026 = ct{1407};
t4028 = ct{1408};
t4029 = ct{1409};
t403 = ct{1410};
t4034 = ct{1411};
t4037 = ct{1412};
t4041 = ct{1413};
t4042 = ct{1414};
t4045 = ct{1415};
t4046 = ct{1416};
t4047 = ct{1417};
t4050 = ct{1418};
t4051 = ct{1419};
t4053 = ct{1420};
t4055 = ct{1421};
t4056 = ct{1422};
t4057 = ct{1423};
t4059 = ct{1424};
t406 = ct{1425};
t4062 = ct{1426};
t4063 = ct{1427};
t4064 = ct{1428};
t4067 = ct{1429};
t4068 = ct{1430};
t4069 = ct{1431};
t4070 = ct{1432};
t4071 = ct{1433};
t4072 = ct{1434};
t4073 = ct{1435};
t4074 = ct{1436};
t4075 = ct{1437};
t4076 = ct{1438};
t4079 = ct{1439};
t4080 = ct{1440};
t4083 = ct{1441};
t4085 = ct{1442};
t4086 = ct{1443};
t4087 = ct{1444};
t4088 = ct{1445};
t4089 = ct{1446};
t4091 = ct{1447};
t4092 = ct{1448};
t4093 = ct{1449};
t4094 = ct{1450};
t4095 = ct{1451};
t4096 = ct{1452};
t4099 = ct{1453};
t410 = ct{1454};
t4100 = ct{1455};
t4102 = ct{1456};
t4103 = ct{1457};
t4104 = ct{1458};
t4108 = ct{1459};
t411 = ct{1460};
t4113 = ct{1461};
t4115 = ct{1462};
t4118 = ct{1463};
t4119 = ct{1464};
t412 = ct{1465};
t4121 = ct{1466};
t4122 = ct{1467};
t4123 = ct{1468};
t4126 = ct{1469};
t4127 = ct{1470};
t413 = ct{1471};
t4132 = ct{1472};
t4134 = ct{1473};
t4138 = ct{1474};
t414 = ct{1475};
t4141 = ct{1476};
t4143 = ct{1477};
t4146 = ct{1478};
t4148 = ct{1479};
t4149 = ct{1480};
t415 = ct{1481};
t4152 = ct{1482};
t4153 = ct{1483};
t4154 = ct{1484};
t4158 = ct{1485};
t416 = ct{1486};
t4161 = ct{1487};
t4166 = ct{1488};
t417 = ct{1489};
t4173 = ct{1490};
t4178 = ct{1491};
t4179 = ct{1492};
t418 = ct{1493};
t4181 = ct{1494};
t4183 = ct{1495};
t4184 = ct{1496};
t4185 = ct{1497};
t4186 = ct{1498};
t4190 = ct{1499};
t4196 = ct{1500};
t4197 = ct{1501};
t4198 = ct{1502};
t4199 = ct{1503};
t420 = ct{1504};
t4205 = ct{1505};
t4206 = ct{1506};
t4208 = ct{1507};
t4209 = ct{1508};
t4210 = ct{1509};
t4211 = ct{1510};
t4215 = ct{1511};
t4217 = ct{1512};
t4218 = ct{1513};
t4219 = ct{1514};
t422 = ct{1515};
t4221 = ct{1516};
t4223 = ct{1517};
t4224 = ct{1518};
t4226 = ct{1519};
t4228 = ct{1520};
t423 = ct{1521};
t4230 = ct{1522};
t4231 = ct{1523};
t4232 = ct{1524};
t4233 = ct{1525};
t4234 = ct{1526};
t4235 = ct{1527};
t424 = ct{1528};
t4241 = ct{1529};
t4243 = ct{1530};
t4245 = ct{1531};
t4246 = ct{1532};
t4247 = ct{1533};
t4248 = ct{1534};
t4249 = ct{1535};
t425 = ct{1536};
t4250 = ct{1537};
t4251 = ct{1538};
t4254 = ct{1539};
t4255 = ct{1540};
t4256 = ct{1541};
t4257 = ct{1542};
t4259 = ct{1543};
t4260 = ct{1544};
t4261 = ct{1545};
t4262 = ct{1546};
t4263 = ct{1547};
t427 = ct{1548};
t4274 = ct{1549};
t4276 = ct{1550};
t4278 = ct{1551};
t4279 = ct{1552};
t428 = ct{1553};
t4280 = ct{1554};
t4282 = ct{1555};
t4283 = ct{1556};
t4284 = ct{1557};
t4285 = ct{1558};
t4286 = ct{1559};
t4287 = ct{1560};
t4289 = ct{1561};
t429 = ct{1562};
t4290 = ct{1563};
t4292 = ct{1564};
t4293 = ct{1565};
t4295 = ct{1566};
t4296 = ct{1567};
t4297 = ct{1568};
t4298 = ct{1569};
t4299 = ct{1570};
t4301 = ct{1571};
t4303 = ct{1572};
t4304 = ct{1573};
t4305 = ct{1574};
t4306 = ct{1575};
t431 = ct{1576};
t4315 = ct{1577};
t4317 = ct{1578};
t4318 = ct{1579};
t432 = ct{1580};
t4323 = ct{1581};
t4324 = ct{1582};
t4325 = ct{1583};
t4326 = ct{1584};
t4327 = ct{1585};
t4329 = ct{1586};
t433 = ct{1587};
t4330 = ct{1588};
t4332 = ct{1589};
t4333 = ct{1590};
t4334 = ct{1591};
t4335 = ct{1592};
t4337 = ct{1593};
t4338 = ct{1594};
t4339 = ct{1595};
t434 = ct{1596};
t4342 = ct{1597};
t4344 = ct{1598};
t4345 = ct{1599};
t4346 = ct{1600};
t4347 = ct{1601};
t4348 = ct{1602};
t4349 = ct{1603};
t435 = ct{1604};
t4350 = ct{1605};
t436 = ct{1606};
t4363 = ct{1607};
t4365 = ct{1608};
t4366 = ct{1609};
t4368 = ct{1610};
t4369 = ct{1611};
t437 = ct{1612};
t4370 = ct{1613};
t4371 = ct{1614};
t4373 = ct{1615};
t4374 = ct{1616};
t4377 = ct{1617};
t4378 = ct{1618};
t438 = ct{1619};
t4380 = ct{1620};
t4382 = ct{1621};
t4383 = ct{1622};
t4385 = ct{1623};
t4387 = ct{1624};
t4388 = ct{1625};
t439 = ct{1626};
t4392 = ct{1627};
t4394 = ct{1628};
t4395 = ct{1629};
t4396 = ct{1630};
t4397 = ct{1631};
t4399 = ct{1632};
t44 = ct{1633};
t440 = ct{1634};
t4402 = ct{1635};
t4403 = ct{1636};
t4405 = ct{1637};
t4406 = ct{1638};
t4407 = ct{1639};
t4409 = ct{1640};
t441 = ct{1641};
t4410 = ct{1642};
t4412 = ct{1643};
t4413 = ct{1644};
t4414 = ct{1645};
t4416 = ct{1646};
t4417 = ct{1647};
t4418 = ct{1648};
t4419 = ct{1649};
t442 = ct{1650};
t4420 = ct{1651};
t4421 = ct{1652};
t4423 = ct{1653};
t4425 = ct{1654};
t4426 = ct{1655};
t4427 = ct{1656};
t4428 = ct{1657};
t4429 = ct{1658};
t4431 = ct{1659};
t4432 = ct{1660};
t4433 = ct{1661};
t4434 = ct{1662};
t4435 = ct{1663};
t4436 = ct{1664};
t4437 = ct{1665};
t4438 = ct{1666};
t4439 = ct{1667};
t444 = ct{1668};
t4440 = ct{1669};
t4444 = ct{1670};
t4446 = ct{1671};
t4447 = ct{1672};
t4449 = ct{1673};
t445 = ct{1674};
t4450 = ct{1675};
t4453 = ct{1676};
t4460 = ct{1677};
t4462 = ct{1678};
t4463 = ct{1679};
t4464 = ct{1680};
t4467 = ct{1681};
t4468 = ct{1682};
t4469 = ct{1683};
t4470 = ct{1684};
t4471 = ct{1685};
t4473 = ct{1686};
t4474 = ct{1687};
t4475 = ct{1688};
t4478 = ct{1689};
t4479 = ct{1690};
t448 = ct{1691};
t4482 = ct{1692};
t4483 = ct{1693};
t4484 = ct{1694};
t4485 = ct{1695};
t4486 = ct{1696};
t4487 = ct{1697};
t4488 = ct{1698};
t4489 = ct{1699};
t449 = ct{1700};
t4490 = ct{1701};
t4494 = ct{1702};
t4495 = ct{1703};
t4498 = ct{1704};
t4499 = ct{1705};
t45 = ct{1706};
t450 = ct{1707};
t4500 = ct{1708};
t4501 = ct{1709};
t4502 = ct{1710};
t4503 = ct{1711};
t4504 = ct{1712};
t4505 = ct{1713};
t4506 = ct{1714};
t4507 = ct{1715};
t4508 = ct{1716};
t4509 = ct{1717};
t4510 = ct{1718};
t4512 = ct{1719};
t4515 = ct{1720};
t4518 = ct{1721};
t4519 = ct{1722};
t452 = ct{1723};
t4520 = ct{1724};
t4521 = ct{1725};
t4522 = ct{1726};
t4523 = ct{1727};
t4526 = ct{1728};
t4527 = ct{1729};
t4528 = ct{1730};
t453 = ct{1731};
t4530 = ct{1732};
t4534 = ct{1733};
t4536 = ct{1734};
t4538 = ct{1735};
t4539 = ct{1736};
t454 = ct{1737};
t4541 = ct{1738};
t4543 = ct{1739};
t4545 = ct{1740};
t4546 = ct{1741};
t4549 = ct{1742};
t4551 = ct{1743};
t4552 = ct{1744};
t4553 = ct{1745};
t4556 = ct{1746};
t4557 = ct{1747};
t4558 = ct{1748};
t4559 = ct{1749};
t4560 = ct{1750};
t4565 = ct{1751};
t4568 = ct{1752};
t4569 = ct{1753};
t457 = ct{1754};
t4570 = ct{1755};
t4572 = ct{1756};
t4575 = ct{1757};
t4577 = ct{1758};
t4578 = ct{1759};
t458 = ct{1760};
t4581 = ct{1761};
t4582 = ct{1762};
t4586 = ct{1763};
t4587 = ct{1764};
t4588 = ct{1765};
t4589 = ct{1766};
t459 = ct{1767};
t4590 = ct{1768};
t4591 = ct{1769};
t4592 = ct{1770};
t4593 = ct{1771};
t4595 = ct{1772};
t4596 = ct{1773};
t4597 = ct{1774};
t4598 = ct{1775};
t460 = ct{1776};
t4600 = ct{1777};
t4601 = ct{1778};
t4602 = ct{1779};
t4604 = ct{1780};
t4605 = ct{1781};
t4606 = ct{1782};
t4607 = ct{1783};
t4608 = ct{1784};
t461 = ct{1785};
t4614 = ct{1786};
t4616 = ct{1787};
t4619 = ct{1788};
t462 = ct{1789};
t4621 = ct{1790};
t4622 = ct{1791};
t4623 = ct{1792};
t4624 = ct{1793};
t4625 = ct{1794};
t4626 = ct{1795};
t4629 = ct{1796};
t463 = ct{1797};
t4633 = ct{1798};
t4634 = ct{1799};
t4636 = ct{1800};
t4637 = ct{1801};
t4639 = ct{1802};
t464 = ct{1803};
t4640 = ct{1804};
t4644 = ct{1805};
t4645 = ct{1806};
t4647 = ct{1807};
t4648 = ct{1808};
t465 = ct{1809};
t4650 = ct{1810};
t4652 = ct{1811};
t4653 = ct{1812};
t4654 = ct{1813};
t4656 = ct{1814};
t4657 = ct{1815};
t4659 = ct{1816};
t466 = ct{1817};
t4660 = ct{1818};
t4662 = ct{1819};
t4663 = ct{1820};
t4666 = ct{1821};
t4667 = ct{1822};
t4668 = ct{1823};
t4669 = ct{1824};
t4670 = ct{1825};
t4673 = ct{1826};
t4674 = ct{1827};
t4675 = ct{1828};
t4677 = ct{1829};
t4678 = ct{1830};
t4679 = ct{1831};
t468 = ct{1832};
t4680 = ct{1833};
t4681 = ct{1834};
t4682 = ct{1835};
t4683 = ct{1836};
t4684 = ct{1837};
t4685 = ct{1838};
t4686 = ct{1839};
t4687 = ct{1840};
t469 = ct{1841};
t4694 = ct{1842};
t4695 = ct{1843};
t4696 = ct{1844};
t4697 = ct{1845};
t4699 = ct{1846};
t47 = ct{1847};
t470 = ct{1848};
t4700 = ct{1849};
t4703 = ct{1850};
t4707 = ct{1851};
t4708 = ct{1852};
t4709 = ct{1853};
t471 = ct{1854};
t4711 = ct{1855};
t4714 = ct{1856};
t4717 = ct{1857};
t4718 = ct{1858};
t4719 = ct{1859};
t472 = ct{1860};
t4720 = ct{1861};
t4721 = ct{1862};
t4722 = ct{1863};
t4723 = ct{1864};
t4724 = ct{1865};
t4725 = ct{1866};
t4726 = ct{1867};
t4727 = ct{1868};
t4728 = ct{1869};
t4731 = ct{1870};
t4732 = ct{1871};
t4733 = ct{1872};
t4734 = ct{1873};
t4737 = ct{1874};
t4738 = ct{1875};
t4739 = ct{1876};
t4742 = ct{1877};
t4743 = ct{1878};
t4745 = ct{1879};
t4747 = ct{1880};
t4748 = ct{1881};
t475 = ct{1882};
t4754 = ct{1883};
t4755 = ct{1884};
t4756 = ct{1885};
t4762 = ct{1886};
t4763 = ct{1887};
t4764 = ct{1888};
t4767 = ct{1889};
t477 = ct{1890};
t4772 = ct{1891};
t4773 = ct{1892};
t4775 = ct{1893};
t4780 = ct{1894};
t4781 = ct{1895};
t4782 = ct{1896};
t4783 = ct{1897};
t4785 = ct{1898};
t4786 = ct{1899};
t479 = ct{1900};
t480 = ct{1901};
t4803 = ct{1902};
t481 = ct{1903};
t4810 = ct{1904};
t4811 = ct{1905};
t482 = ct{1906};
t4824 = ct{1907};
t4825 = ct{1908};
t4826 = ct{1909};
t483 = ct{1910};
t4831 = ct{1911};
t4837 = ct{1912};
t4838 = ct{1913};
t4842 = ct{1914};
t4846 = ct{1915};
t485 = ct{1916};
t486 = ct{1917};
t4862 = ct{1918};
t4864 = ct{1919};
t4865 = ct{1920};
t4866 = ct{1921};
t4867 = ct{1922};
t4869 = ct{1923};
t4870 = ct{1924};
t4877 = ct{1925};
t488 = ct{1926};
t4884 = ct{1927};
t489 = ct{1928};
t4903 = ct{1929};
t4904 = ct{1930};
t491 = ct{1931};
t4911 = ct{1932};
t4914 = ct{1933};
t4919 = ct{1934};
t492 = ct{1935};
t4920 = ct{1936};
t4922 = ct{1937};
t4924 = ct{1938};
t4925 = ct{1939};
t4927 = ct{1940};
t4929 = ct{1941};
t493 = ct{1942};
t4934 = ct{1943};
t4936 = ct{1944};
t494 = ct{1945};
t4942 = ct{1946};
t4944 = ct{1947};
t4946 = ct{1948};
t4949 = ct{1949};
t4950 = ct{1950};
t4952 = ct{1951};
t4953 = ct{1952};
t4957 = ct{1953};
t496 = ct{1954};
t4964 = ct{1955};
t4966 = ct{1956};
t4967 = ct{1957};
t4969 = ct{1958};
t497 = ct{1959};
t4973 = ct{1960};
t4974 = ct{1961};
t4979 = ct{1962};
t498 = ct{1963};
t4981 = ct{1964};
t4982 = ct{1965};
t4983 = ct{1966};
t4984 = ct{1967};
t4987 = ct{1968};
t4988 = ct{1969};
t4989 = ct{1970};
t499 = ct{1971};
t4990 = ct{1972};
t4993 = ct{1973};
t4994 = ct{1974};
t4995 = ct{1975};
t4996 = ct{1976};
t5 = ct{1977};
t50 = ct{1978};
t500 = ct{1979};
t5000 = ct{1980};
t5001 = ct{1981};
t5002 = ct{1982};
t5007 = ct{1983};
t5008 = ct{1984};
t5009 = ct{1985};
t501 = ct{1986};
t5016 = ct{1987};
t5017 = ct{1988};
t502 = ct{1989};
t5020 = ct{1990};
t5021 = ct{1991};
t5022 = ct{1992};
t5023 = ct{1993};
t5024 = ct{1994};
t5026 = ct{1995};
t5027 = ct{1996};
t503 = ct{1997};
t5031 = ct{1998};
t5032 = ct{1999};
t5039 = ct{2000};
t504 = ct{2001};
t5043 = ct{2002};
t5049 = ct{2003};
t505 = ct{2004};
t5050 = ct{2005};
t5056 = ct{2006};
t5058 = ct{2007};
t506 = ct{2008};
t5061 = ct{2009};
t5063 = ct{2010};
t5064 = ct{2011};
t5065 = ct{2012};
t507 = ct{2013};
t5074 = ct{2014};
t5075 = ct{2015};
t5076 = ct{2016};
t508 = ct{2017};
t5080 = ct{2018};
t5083 = ct{2019};
t5084 = ct{2020};
t5086 = ct{2021};
t5087 = ct{2022};
t509 = ct{2023};
t5090 = ct{2024};
t5091 = ct{2025};
t5092 = ct{2026};
t5093 = ct{2027};
t5097 = ct{2028};
t5098 = ct{2029};
t5099 = ct{2030};
t510 = ct{2031};
t5100 = ct{2032};
t5102 = ct{2033};
t5107 = ct{2034};
t511 = ct{2035};
t5110 = ct{2036};
t5112 = ct{2037};
t5113 = ct{2038};
t5114 = ct{2039};
t512 = ct{2040};
t5121 = ct{2041};
t5123 = ct{2042};
t513 = ct{2043};
t5131 = ct{2044};
t5132 = ct{2045};
t5136 = ct{2046};
t5139 = ct{2047};
t514 = ct{2048};
t5140 = ct{2049};
t5143 = ct{2050};
t5144 = ct{2051};
t5145 = ct{2052};
t5147 = ct{2053};
t5148 = ct{2054};
t5150 = ct{2055};
t5151 = ct{2056};
t516 = ct{2057};
t5163 = ct{2058};
t5164 = ct{2059};
t5166 = ct{2060};
t5167 = ct{2061};
t517 = ct{2062};
t5175 = ct{2063};
t5177 = ct{2064};
t518 = ct{2065};
t5182 = ct{2066};
t5184 = ct{2067};
t5188 = ct{2068};
t5189 = ct{2069};
t5194 = ct{2070};
t5195 = ct{2071};
t520 = ct{2072};
t5200 = ct{2073};
t5202 = ct{2074};
t5203 = ct{2075};
t5204 = ct{2076};
t5205 = ct{2077};
t5206 = ct{2078};
t521 = ct{2079};
t5210 = ct{2080};
t5211 = ct{2081};
t5215 = ct{2082};
t5217 = ct{2083};
t5219 = ct{2084};
t522 = ct{2085};
t5222 = ct{2086};
t5227 = ct{2087};
t5228 = ct{2088};
t523 = ct{2089};
t5231 = ct{2090};
t5232 = ct{2091};
t5233 = ct{2092};
t5235 = ct{2093};
t5236 = ct{2094};
t5237 = ct{2095};
t5238 = ct{2096};
t524 = ct{2097};
t5242 = ct{2098};
t5244 = ct{2099};
t5249 = ct{2100};
t525 = ct{2101};
t5251 = ct{2102};
t5252 = ct{2103};
t5254 = ct{2104};
t5255 = ct{2105};
t5256 = ct{2106};
t5258 = ct{2107};
t5259 = ct{2108};
t526 = ct{2109};
t5260 = ct{2110};
t5261 = ct{2111};
t5262 = ct{2112};
t5264 = ct{2113};
t5266 = ct{2114};
t5269 = ct{2115};
t527 = ct{2116};
t5275 = ct{2117};
t5279 = ct{2118};
t528 = ct{2119};
t5280 = ct{2120};
t5285 = ct{2121};
t5286 = ct{2122};
t529 = ct{2123};
t5291 = ct{2124};
t5294 = ct{2125};
t5296 = ct{2126};
t5297 = ct{2127};
t5299 = ct{2128};
t53 = ct{2129};
t530 = ct{2130};
t5301 = ct{2131};
t5302 = ct{2132};
t5307 = ct{2133};
t5309 = ct{2134};
t531 = ct{2135};
t5314 = ct{2136};
t5316 = ct{2137};
t5318 = ct{2138};
t532 = ct{2139};
t5320 = ct{2140};
t5321 = ct{2141};
t5322 = ct{2142};
t5323 = ct{2143};
t5324 = ct{2144};
t533 = ct{2145};
t5333 = ct{2146};
t5335 = ct{2147};
t5337 = ct{2148};
t5339 = ct{2149};
t534 = ct{2150};
t5340 = ct{2151};
t5344 = ct{2152};
t535 = ct{2153};
t5354 = ct{2154};
t5356 = ct{2155};
t5357 = ct{2156};
t5358 = ct{2157};
t5359 = ct{2158};
t536 = ct{2159};
t5361 = ct{2160};
t5364 = ct{2161};
t5369 = ct{2162};
t537 = ct{2163};
t5370 = ct{2164};
t5371 = ct{2165};
t5372 = ct{2166};
t5373 = ct{2167};
t5375 = ct{2168};
t5378 = ct{2169};
t5379 = ct{2170};
t538 = ct{2171};
t5380 = ct{2172};
t5381 = ct{2173};
t5382 = ct{2174};
t5383 = ct{2175};
t5385 = ct{2176};
t5389 = ct{2177};
t539 = ct{2178};
t5390 = ct{2179};
t5391 = ct{2180};
t5392 = ct{2181};
t5393 = ct{2182};
t5394 = ct{2183};
t5395 = ct{2184};
t5396 = ct{2185};
t5397 = ct{2186};
t5399 = ct{2187};
t540 = ct{2188};
t5401 = ct{2189};
t5402 = ct{2190};
t5403 = ct{2191};
t5404 = ct{2192};
t5405 = ct{2193};
t5406 = ct{2194};
t5408 = ct{2195};
t5409 = ct{2196};
t5410 = ct{2197};
t5411 = ct{2198};
t5412 = ct{2199};
t5414 = ct{2200};
t5415 = ct{2201};
t5416 = ct{2202};
t5418 = ct{2203};
t5422 = ct{2204};
t5423 = ct{2205};
t5426 = ct{2206};
t5427 = ct{2207};
t5428 = ct{2208};
t543 = ct{2209};
t5431 = ct{2210};
t5436 = ct{2211};
t5438 = ct{2212};
t544 = ct{2213};
t5442 = ct{2214};
t5443 = ct{2215};
t5447 = ct{2216};
t545 = ct{2217};
t5450 = ct{2218};
t5451 = ct{2219};
t5457 = ct{2220};
t5459 = ct{2221};
t546 = ct{2222};
t5464 = ct{2223};
t5465 = ct{2224};
t5466 = ct{2225};
t547 = ct{2226};
t5479 = ct{2227};
t548 = ct{2228};
t5480 = ct{2229};
t5482 = ct{2230};
t5483 = ct{2231};
t5484 = ct{2232};
t5486 = ct{2233};
t5487 = ct{2234};
t5488 = ct{2235};
t549 = ct{2236};
t5507 = ct{2237};
t551 = ct{2238};
t5512 = ct{2239};
t5515 = ct{2240};
t552 = ct{2241};
t5521 = ct{2242};
t5526 = ct{2243};
t553 = ct{2244};
t554 = ct{2245};
t555 = ct{2246};
t556 = ct{2247};
t557 = ct{2248};
t558 = ct{2249};
t559 = ct{2250};
t560 = ct{2251};
t5602 = ct{2252};
t5605 = ct{2253};
t561 = ct{2254};
t5616 = ct{2255};
t5617 = ct{2256};
t5619 = ct{2257};
t562 = ct{2258};
t5620 = ct{2259};
t5621 = ct{2260};
t5622 = ct{2261};
t5623 = ct{2262};
t5624 = ct{2263};
t5625 = ct{2264};
t5626 = ct{2265};
t5628 = ct{2266};
t563 = ct{2267};
t5630 = ct{2268};
t5633 = ct{2269};
t5634 = ct{2270};
t5636 = ct{2271};
t5639 = ct{2272};
t564 = ct{2273};
t5642 = ct{2274};
t5644 = ct{2275};
t5648 = ct{2276};
t5657 = ct{2277};
t5658 = ct{2278};
t5662 = ct{2279};
t5665 = ct{2280};
t5666 = ct{2281};
t567 = ct{2282};
t5670 = ct{2283};
t5679 = ct{2284};
t568 = ct{2285};
t5682 = ct{2286};
t5684 = ct{2287};
t5688 = ct{2288};
t569 = ct{2289};
t5691 = ct{2290};
t5692 = ct{2291};
t5694 = ct{2292};
t5696 = ct{2293};
t5698 = ct{2294};
t5699 = ct{2295};
t57 = ct{2296};
t570 = ct{2297};
t5701 = ct{2298};
t5703 = ct{2299};
t5704 = ct{2300};
t5705 = ct{2301};
t5707 = ct{2302};
t571 = ct{2303};
t5711 = ct{2304};
t5713 = ct{2305};
t5714 = ct{2306};
t5718 = ct{2307};
t572 = ct{2308};
t5720 = ct{2309};
t5722 = ct{2310};
t5723 = ct{2311};
t5724 = ct{2312};
t5726 = ct{2313};
t5727 = ct{2314};
t5728 = ct{2315};
t573 = ct{2316};
t5731 = ct{2317};
t5732 = ct{2318};
t5733 = ct{2319};
t5736 = ct{2320};
t5738 = ct{2321};
t574 = ct{2322};
t5742 = ct{2323};
t5745 = ct{2324};
t5746 = ct{2325};
t5747 = ct{2326};
t5748 = ct{2327};
t5751 = ct{2328};
t5754 = ct{2329};
t5757 = ct{2330};
t5759 = ct{2331};
t576 = ct{2332};
t5760 = ct{2333};
t5763 = ct{2334};
t5765 = ct{2335};
t5768 = ct{2336};
t5770 = ct{2337};
t5771 = ct{2338};
t5772 = ct{2339};
t5773 = ct{2340};
t5774 = ct{2341};
t5775 = ct{2342};
t5776 = ct{2343};
t5778 = ct{2344};
t5779 = ct{2345};
t578 = ct{2346};
t5782 = ct{2347};
t5784 = ct{2348};
t5786 = ct{2349};
t5787 = ct{2350};
t5788 = ct{2351};
t579 = ct{2352};
t5790 = ct{2353};
t5792 = ct{2354};
t5794 = ct{2355};
t5795 = ct{2356};
t5797 = ct{2357};
t58 = ct{2358};
t580 = ct{2359};
t5808 = ct{2360};
t5809 = ct{2361};
t581 = ct{2362};
t5810 = ct{2363};
t5813 = ct{2364};
t5814 = ct{2365};
t5818 = ct{2366};
t5819 = ct{2367};
t582 = ct{2368};
t5822 = ct{2369};
t5823 = ct{2370};
t5824 = ct{2371};
t5825 = ct{2372};
t5826 = ct{2373};
t5827 = ct{2374};
t5828 = ct{2375};
t5829 = ct{2376};
t5830 = ct{2377};
t5831 = ct{2378};
t5832 = ct{2379};
t5833 = ct{2380};
t5834 = ct{2381};
t5835 = ct{2382};
t5836 = ct{2383};
t5838 = ct{2384};
t584 = ct{2385};
t5842 = ct{2386};
t5843 = ct{2387};
t5844 = ct{2388};
t5845 = ct{2389};
t5846 = ct{2390};
t5849 = ct{2391};
t5850 = ct{2392};
t5851 = ct{2393};
t5852 = ct{2394};
t5859 = ct{2395};
t586 = ct{2396};
t5860 = ct{2397};
t5861 = ct{2398};
t5862 = ct{2399};
t5863 = ct{2400};
t5868 = ct{2401};
t5869 = ct{2402};
t587 = ct{2403};
t5870 = ct{2404};
t5871 = ct{2405};
t5872 = ct{2406};
t5873 = ct{2407};
t5874 = ct{2408};
t5875 = ct{2409};
t5876 = ct{2410};
t5881 = ct{2411};
t5882 = ct{2412};
t5883 = ct{2413};
t5884 = ct{2414};
t5885 = ct{2415};
t5886 = ct{2416};
t5887 = ct{2417};
t5888 = ct{2418};
t5889 = ct{2419};
t589 = ct{2420};
t5890 = ct{2421};
t5891 = ct{2422};
t5892 = ct{2423};
t5893 = ct{2424};
t5894 = ct{2425};
t5895 = ct{2426};
t5896 = ct{2427};
t5898 = ct{2428};
t5899 = ct{2429};
t590 = ct{2430};
t5901 = ct{2431};
t5902 = ct{2432};
t5903 = ct{2433};
t5905 = ct{2434};
t5906 = ct{2435};
t5909 = ct{2436};
t591 = ct{2437};
t5917 = ct{2438};
t5918 = ct{2439};
t5919 = ct{2440};
t592 = ct{2441};
t5920 = ct{2442};
t5925 = ct{2443};
t5928 = ct{2444};
t593 = ct{2445};
t5930 = ct{2446};
t5931 = ct{2447};
t5932 = ct{2448};
t5933 = ct{2449};
t5934 = ct{2450};
t5935 = ct{2451};
t5936 = ct{2452};
t5938 = ct{2453};
t5939 = ct{2454};
t594 = ct{2455};
t5940 = ct{2456};
t595 = ct{2457};
t5954 = ct{2458};
t5956 = ct{2459};
t5957 = ct{2460};
t5958 = ct{2461};
t5959 = ct{2462};
t596 = ct{2463};
t5960 = ct{2464};
t5964 = ct{2465};
t5965 = ct{2466};
t5966 = ct{2467};
t5967 = ct{2468};
t597 = ct{2469};
t5970 = ct{2470};
t5971 = ct{2471};
t5972 = ct{2472};
t5976 = ct{2473};
t5977 = ct{2474};
t5978 = ct{2475};
t5979 = ct{2476};
t5980 = ct{2477};
t5981 = ct{2478};
t5982 = ct{2479};
t5984 = ct{2480};
t5988 = ct{2481};
t5994 = ct{2482};
t5996 = ct{2483};
t5998 = ct{2484};
t5999 = ct{2485};
t6 = ct{2486};
t60 = ct{2487};
t600 = ct{2488};
t6000 = ct{2489};
t6001 = ct{2490};
t6002 = ct{2491};
t6003 = ct{2492};
t6005 = ct{2493};
t6007 = ct{2494};
t6011 = ct{2495};
t6012 = ct{2496};
t6013 = ct{2497};
t6014 = ct{2498};
t6017 = ct{2499};
t602 = ct{2500};
t603 = ct{2501};
t6038 = ct{2502};
t604 = ct{2503};
t6043 = ct{2504};
t6045 = ct{2505};
t6046 = ct{2506};
t6047 = ct{2507};
t605 = ct{2508};
t6060 = ct{2509};
t6061 = ct{2510};
t6062 = ct{2511};
t6064 = ct{2512};
t6065 = ct{2513};
t6069 = ct{2514};
t6075 = ct{2515};
t6077 = ct{2516};
t6079 = ct{2517};
t6086 = ct{2518};
t609 = ct{2519};
t610 = ct{2520};
t6101 = ct{2521};
t6102 = ct{2522};
t6103 = ct{2523};
t6105 = ct{2524};
t6106 = ct{2525};
t6108 = ct{2526};
t6109 = ct{2527};
t611 = ct{2528};
t6117 = ct{2529};
t6119 = ct{2530};
t612 = ct{2531};
t6123 = ct{2532};
t6124 = ct{2533};
t6126 = ct{2534};
t613 = ct{2535};
t6136 = ct{2536};
t6139 = ct{2537};
t614 = ct{2538};
t6140 = ct{2539};
t6149 = ct{2540};
t615 = ct{2541};
t616 = ct{2542};
t618 = ct{2543};
t619 = ct{2544};
t6195 = ct{2545};
t620 = ct{2546};
t6203 = ct{2547};
t6204 = ct{2548};
t6205 = ct{2549};
t6206 = ct{2550};
t6209 = ct{2551};
t621 = ct{2552};
t6210 = ct{2553};
t622 = ct{2554};
t623 = ct{2555};
t624 = ct{2556};
t625 = ct{2557};
t626 = ct{2558};
t629 = ct{2559};
t6319 = ct{2560};
t632 = ct{2561};
t6329 = ct{2562};
t6330 = ct{2563};
t6338 = ct{2564};
t6341 = ct{2565};
t6342 = ct{2566};
t6343 = ct{2567};
t6347 = ct{2568};
t6348 = ct{2569};
t6349 = ct{2570};
t6350 = ct{2571};
t6351 = ct{2572};
t6352 = ct{2573};
t6362 = ct{2574};
t638 = ct{2575};
t6391 = ct{2576};
t6395 = ct{2577};
t640 = ct{2578};
t6403 = ct{2579};
t6416 = ct{2580};
t6417 = ct{2581};
t6436 = ct{2582};
t6437 = ct{2583};
t6462 = ct{2584};
t6463 = ct{2585};
t6471 = ct{2586};
t650 = ct{2587};
t6506 = ct{2588};
t654 = ct{2589};
t6565 = ct{2590};
t658 = ct{2591};
t6597 = ct{2592};
t6609 = ct{2593};
t6689 = ct{2594};
t669 = ct{2595};
t6690 = ct{2596};
t673 = ct{2597};
t679 = ct{2598};
t681 = ct{2599};
t6826 = ct{2600};
t6827 = ct{2601};
t683 = ct{2602};
t684 = ct{2603};
t7 = ct{2604};
t7012 = ct{2605};
t7020 = ct{2606};
t7043 = ct{2607};
t705 = ct{2608};
t706 = ct{2609};
t7079 = ct{2610};
t708 = ct{2611};
t7080 = ct{2612};
t7087 = ct{2613};
t71 = ct{2614};
t7104 = ct{2615};
t7119 = ct{2616};
t712 = ct{2617};
t7148 = ct{2618};
t7149 = ct{2619};
t716 = ct{2620};
t72 = ct{2621};
t724 = ct{2622};
t7256 = ct{2623};
t73 = ct{2624};
t731 = ct{2625};
t733 = ct{2626};
t7333 = ct{2627};
t7364 = ct{2628};
t738 = ct{2629};
t739 = ct{2630};
t741 = ct{2631};
t742 = ct{2632};
t743 = ct{2633};
t744 = ct{2634};
t746 = ct{2635};
t748 = ct{2636};
t749 = ct{2637};
t75 = ct{2638};
t750 = ct{2639};
t752 = ct{2640};
t7528 = ct{2641};
t753 = ct{2642};
t7549 = ct{2643};
t7553 = ct{2644};
t7556 = ct{2645};
t7566 = ct{2646};
t7570 = ct{2647};
t7573 = ct{2648};
t759 = ct{2649};
t76 = ct{2650};
t760 = ct{2651};
t764 = ct{2652};
t765 = ct{2653};
t766 = ct{2654};
t773 = ct{2655};
t777 = ct{2656};
t778 = ct{2657};
t779 = ct{2658};
t780 = ct{2659};
t781 = ct{2660};
t784 = ct{2661};
t785 = ct{2662};
t792 = ct{2663};
t796 = ct{2664};
t797 = ct{2665};
t8 = ct{2666};
t801 = ct{2667};
t802 = ct{2668};
t803 = ct{2669};
t804 = ct{2670};
t81 = ct{2671};
t823 = ct{2672};
t824 = ct{2673};
t825 = ct{2674};
t826 = ct{2675};
t827 = ct{2676};
t830 = ct{2677};
t832 = ct{2678};
t833 = ct{2679};
t834 = ct{2680};
t835 = ct{2681};
t836 = ct{2682};
t838 = ct{2683};
t84 = ct{2684};
t841 = ct{2685};
t842 = ct{2686};
t843 = ct{2687};
t845 = ct{2688};
t846 = ct{2689};
t847 = ct{2690};
t848 = ct{2691};
t852 = ct{2692};
t856 = ct{2693};
t86 = ct{2694};
t861 = ct{2695};
t863 = ct{2696};
t866 = ct{2697};
t868 = ct{2698};
t869 = ct{2699};
t870 = ct{2700};
t874 = ct{2701};
t875 = ct{2702};
t877 = ct{2703};
t878 = ct{2704};
t880 = ct{2705};
t881 = ct{2706};
t893 = ct{2707};
t899 = ct{2708};
t9 = ct{2709};
t90 = ct{2710};
t902 = ct{2711};
t903 = ct{2712};
t905 = ct{2713};
t908 = ct{2714};
t909 = ct{2715};
t91 = ct{2716};
t910 = ct{2717};
t911 = ct{2718};
t912 = ct{2719};
t914 = ct{2720};
t915 = ct{2721};
t917 = ct{2722};
t919 = ct{2723};
t922 = ct{2724};
t925 = ct{2725};
t926 = ct{2726};
t928 = ct{2727};
t929 = ct{2728};
t930 = ct{2729};
t931 = ct{2730};
t932 = ct{2731};
t934 = ct{2732};
t940 = ct{2733};
t944 = ct{2734};
t945 = ct{2735};
t947 = ct{2736};
t95 = ct{2737};
t952 = ct{2738};
t954 = ct{2739};
t955 = ct{2740};
t957 = ct{2741};
t958 = ct{2742};
t968 = ct{2743};
t97 = ct{2744};
t970 = ct{2745};
t971 = ct{2746};
t972 = ct{2747};
t975 = ct{2748};
t976 = ct{2749};
t984 = ct{2750};
t985 = ct{2751};
t986 = ct{2752};
t989 = ct{2753};
t99 = ct{2754};
t991 = ct{2755};
t998 = ct{2756};
t6156 = t5795.*(t2088-t4743).*(-5.344156668414146e-72);
t6163 = t5795.*(t2088-t4743).*(-7.671525497590686e-73);
t6175 = t6126.*(-7.26735e-3);
t6180 = t6126.*7.26735e-3;
t6182 = t6126.*(-7.26350610236655e-5);
t6187 = t6126.*7.26350610236655e-5;
t6193 = -t5657.*(t4148+t5.*(t2421-t4158));
t6197 = t5657.*(t4148+t5.*(t2421-t4158));
t6198 = t6126.*(-1.40259855e-11);
t6199 = -t6195;
t6200 = t6126.*1.40259855e-11;
t6201 = (t5657.*t5886)./2.0;
t6207 = -t6205;
t6208 = -t6206;
t6211 = -t6209;
t6212 = -t6210;
t6215 = t5657.*t5903;
t6241 = t6195.*7.26350610236655e-5;
t6249 = t6195.*1.246862701090643e-6;
t6251 = t6195.*1.744166498897461e-6;
t6267 = t6195.*1.40259855e-11;
t6269 = t6195.*4.126305279697715e-13;
t6271 = (t520.*t6136)./2.0;
t6276 = (t579.*t6136)./2.0;
t6280 = (t6136.*(t97-t8.*t9.*1.33637579258949e-4))./2.0;
t6331 = -t6330;
t6340 = t5810.*(t3136-t5691).*-2.0;
t6344 = t5861.*((t197.*(t29-t30))./9.007199254740992e+15+t3.*(t3219-t3230)).*-2.0;
t6354 = t5861.*(t7.*(t3719-t3788)+(t3.*t34.*t191.*(t29-t30))./8.112963841460668e+31).*-2.0;
t6360 = t9.*t6351.*7.01299275e-12;
t6364 = -t5903.*(t4148+t5.*(t2421-t4158));
t6366 = t4.*t91.*t5824.*(t3136-t5691).*(-7.596454196607839e-68);
t6367 = t4.*t5824.*t5861.*(t29-t30).*(-7.596454196607839e-68);
t6372 = t4.*t91.*t5824.*(t3136-t5691).*(-1.015171749786156e-71);
t6373 = t4.*t91.*t5824.*(t3136-t5691).*(-5.520609140571798e-70);
t6374 = t5903.*(t4148+t5.*(t2421-t4158)).*(-7.26735e-3);
t6375 = t4.*t91.*t5824.*(t3136-t5691).*1.015171749786156e-71;
t6376 = t4.*t91.*t5824.*(t3136-t5691).*5.520609140571798e-70;
t6377 = t4.*t91.*t5824.*(t3136-t5691).*(-5.517689141340903e-72);
t6378 = t5903.*(t4148+t5.*(t2421-t4158)).*(-7.26350610236655e-5);
t6379 = t4.*t91.*t5824.*(t3136-t5691).*5.517689141340903e-72;
t6380 = (t1531.*t6350)./2.0;
t6381 = (t1587.*t6349)./2.0;
t6382 = t4.*t91.*t5824.*(t3136-t5691).*(-1.656182742171539e-72);
t6383 = t4.*t5824.*t5861.*(t29-t30).*(-1.015171749786156e-71);
t6384 = t4.*t5824.*t5861.*(t29-t30).*(-5.520609140571798e-70);
t6386 = t4.*t91.*t5824.*(t3136-t5691).*1.656182742171539e-72;
t6387 = t4.*t5824.*t5861.*(t29-t30).*1.015171749786156e-71;
t6388 = t4.*t5824.*t5861.*(t29-t30).*5.520609140571798e-70;
t6389 = t4.*t5824.*t5861.*(t29-t30).*(-5.517689141340903e-72);
t6390 = t4.*t5824.*t5861.*(t29-t30).*5.517689141340903e-72;
t6393 = t4.*t5824.*t5861.*(t29-t30).*(-1.656182742171539e-72);
t6396 = t4.*t5824.*t5861.*(t29-t30).*1.656182742171539e-72;
t6397 = t5903.*(t4148+t5.*(t2421-t4158)).*(-1.40259855e-11);
t6398 = t5903.*(t4148+t5.*(t2421-t4158)).*1.40259855e-11;
t6404 = -t6403;
t6406 = t5.*t6391.*7.01299275e-12;
t6407 = t9.*t6395.*7.01299275e-12;
t6409 = t5050+t5087+t5703+t5713;
t6427 = (t5782.*t6136)./2.0;
t6431 = (t1531.*t6395)./2.0;
t6433 = (t1587.*t6391)./2.0;
t6440 = t91.*t5824.*(t5670+t4.*(t1458-t5665)).*(-7.596454196607839e-68);
t6441 = t5824.*t6103.*(t29-t30).*(-7.596454196607839e-68);
t6456 = t91.*t5824.*(t5670+t4.*(t1458-t5665)).*(-1.015171749786156e-71);
t6457 = t91.*t5824.*(t5670+t4.*(t1458-t5665)).*(-5.520609140571798e-70);
t6458 = t91.*t5824.*(t5670+t4.*(t1458-t5665)).*(-5.517689141340903e-72);
t6459 = t5824.*t6103.*(t29-t30).*(-1.015171749786156e-71);
t6460 = t5824.*t6103.*(t29-t30).*(-5.520609140571798e-70);
t6461 = t5824.*t6103.*(t29-t30).*(-5.517689141340903e-72);
t6469 = t744+t759+t2620+t2644+t3320+t3326+t5925;
t6507 = -t6506;
t6546 = (t626.*t6462)./2.0;
t6548 = (t629.*t6463)./2.0;
t6553 = (t5633.*t6417)./2.0;
t6554 = (t5634.*t6416)./2.0;
t6557 = (t1531.*t6462)./2.0;
t6559 = (t1633.*t6462)./2.0;
t6560 = (t1561.*t6463)./2.0;
t6562 = (t1587.*t6463)./2.0;
t6566 = -t6565;
t6567 = (t5633.*t6436)./2.0;
t6568 = (t5634.*t6437)./2.0;
t6702 = t784+t1645+t1889+t3410+t3704+t3905+t4289+t4439+t5086+t5396+t5427;
t6832 = t673+t683+t748+t764+t2606+t2623+t2639+t2649+t3277+t3296+t6136;
t6868 = (t5294.*t6689)./2.0;
t6871 = (t5358.*t6689)./2.0;
t6872 = (t5321.*t6690)./2.0;
t6873 = (t5361.*t6690)./2.0;
t6874 = t1506+t1542+t1571+t2519+t2796+t2814+t4877+t5016+t5110+t5143+t5369+t5371;
t6895 = (t5633.*t6689)./2.0;
t6902 = (t5634.*t6690)./2.0;
t6919 = t658+t1558+t1637+t3317+t3696+t3698+t4283+t4967+t5092+t5705+t5720;
t6933 = t731+t746+t838+t880+t2673+t2691+t2707+t2711+t3332+t3349+t6349;
t6934 = t733+t752+t834+t842+t2675+t2697+t2708+t2714+t3336+t3351+t6350;
t6994 = t777+t1638+t1709+t1789+t3373+t3454+t3699+t3758+t3842+t4366+t4434+t5397+t5760;
t7000 = t823+t1711+t1713+t1804+t3399+t3411+t3769+t3777+t3848+t4290+t4438+t5399+t5751;
t7010 = t613.*(t5772+t5861.*((t197.*(t29-t30))./9.007199254740992e+15+t3.*(t3219-t3230)).*2.0+t5810.*(t3136-t5691).*2.0).*(-1.0./2.0);
t7011 = (t613.*(t5772+t5861.*((t197.*(t29-t30))./9.007199254740992e+15+t3.*(t3219-t3230)).*2.0+t5810.*(t3136-t5691).*2.0))./2.0;
t7019 = t750+t766+t833+t841+t2625+t2651+t2696+t2713+t3278+t3298+t3366+t3377+t6351;
t7021 = t650+t1549+t1595+t1696+t1729+t3329+t3381+t3402+t3690+t3691+t3793+t3893+t4299+t4346+t5309+t5357;
t7026 = t773+t1632+t1635+t1907+t3228+t3372+t3447+t3693+t3834+t3914+t4363+t4504+t5043+t5379+t5759;
t7032 = t1311+t2317+t2369+t2405+t3713+t3737+t4051+t4079+t4095+t4662+t4703+t5177+t5266+t5724+t5726;
t7033 = t1267+t2316+t2339+t2403+t3654+t3810+t4045+t4063+t4094+t4681+t4700+t5182+t5231+t5732+t5733;
t7044 = (t5.*t7043)./2.0;
t7046 = t708+t1269+t1936+t2340+t2401+t3364+t3729+t3920+t4064+t4092+t4296+t4657+t4726+t5286+t5291+t5296+t5322+t5406;
t7052 = (t1429.*t7043)./2.0;
t7060 = t705+t749+t765+t780+t835+t843+t2624+t2633+t2650+t2669+t2698+t2715+t3288+t3328+t3337+t3352+t6462;
t7061 = t706+t716+t785+t804+t836+t846+t2634+t2659+t2671+t2681+t2700+t2718+t3284+t3303+t3340+t3353+t6463;
t7065 = t743+t870+t1662+t1832+t1859+t2131+t3383+t3476+t3735+t3870+t3872+t3991+t4233+t4297+t4435+t4512+t5188+t5381+t5411+t5428+t5438;
t7082 = t654+t1317+t1505+t1658+t2277+t2372+t2429+t3279+t3502+t3655+t3720+t3731+t3747+t4071+t4080+t4102+t4231+t4663+t4722+t5182+t5194+t5401+t5728+t5733;
t7085 = t679+t1265+t1560+t1850+t2279+t2336+t2430+t3363+t3544+t3653+t3766+t3800+t3865+t4062+t4073+t4104+t4365+t4680+t4725+t5167+t5177+t5414+t5724+t5731;
t7098 = t739+t909+t1606+t1660+t1716+t1836+t1937+t2053+t3396+t3418+t3480+t3481+t3702+t3733+t3876+t3890+t3921+t3969+t4285+t4298+t4350+t4510+t5385+t5415+t5747+t5765;
t7109 = t801+t863+t1566+t1653+t1712+t1851+t1939+t2042+t3275+t3393+t3413+t3442+t3505+t3728+t3789+t3866+t3885+t3942+t3967+t4282+t4374+t4432+t4507+t5256+t5382+t5408+t5754+t5768;
t7153 = t1785+t1866+t2379+t2389+t2410+t2470+t3588+t3624+t4020+t4026+t4072+t4096+t4218+t4247+t4639+t4652+t4687+t4721+t7043;
t7244 = t669+t1267+t1522+t1535+t1669+t1676+t1733+t1903+t2316+t2323+t2339+t2376+t2387+t2391+t2403+t2440+t2455+t3318+t3473+t3573+t3590+t3591+t3604+t3654+t3689+t3799+t3810+t4017+t4024+t4028+t4041+t4045+t4057+t4063+t4087+t4094+t4215+t4245+t4280+t4670+t4679+t4681+t4685+t4700+t4718+t5254+t5264+t5380+t5722+t5736;
t7258 = dq1.*t7256;
t7334 = dq1.*t7333;
t7335 = dq2.*t7333;
t7550 = dq2.*t7549;
t7551 = dq6.*t7549;
t7557 = dq1.*t7556;
t7558 = dq2.*t7556;
t7559 = dq5.*t7556;
t7564 = t7119+t7549;
t7567 = dq1.*t7566;
t7568 = dq2.*t7566;
t7569 = dq4.*t7566;
t7571 = dq2.*t7570;
t7574 = dq1.*t7573;
t7575 = dq5.*t7573;
t7576 = t1752+t1755+t1915+t1920+t1926+t1943+t2000+t2087+t2105+t2108+t2171+t2194+t2218+t2305+t2513+t2545+t3598+t3633+t3657+t3674+t3787+t3796+t3883+t3896+t3908+t3924+t3941+t3973+t3996+t3998+t4122+t4127+t4205+t4224+t4241+t4262+t4292+t4303+t4330+t4399+t4464+t4470+t4484+t4539+t4560+t4569+t4754+t4772+t7566;
t7579 = t2721+t2736+t2758+t2762+t2770+t2828+t2832+t2850+t2854+t2883+t2884+t2907+t2912+t2946+t2993+t2998+t3210+t3223+t4831+t4865+t4922+t4944+t4952+t4969+t4979+t4982+t5001+t5074+t5098+t5131+t5148+t5175+t5200+t5205+t5222+t5237+t5261+t5302+t5436+t5442+t5451+t5479+t5512+t5526+t7570;
t5627 = -t5625;
t5638 = t5625.*(-1.33637579258949e-4);
t5645 = t5625.*(-1.246862701090643e-6);
t5646 = t5625.*(-3.383302988283333e-6);
t5647 = t5625.*(-4.00912737776847e-7);
t5650 = t5624.*1.40259855e-11;
t5651 = t5625.*1.40259855e-11;
t5652 = t5625.*(-3.146556677756745e-13);
t5655 = t5624.*(-4.126305279697715e-13);
t5676 = t5.*t5666;
t5677 = t9.*t5666;
t5681 = t2225+t4767;
t5683 = t2276+t4764;
t5700 = t5666.*1.33637579258949e-4;
t5702 = t5622.*(t81-t86).*(-1.0./2.0);
t5706 = t47.*t5666;
t5708 = (t5622.*(t81-t86))./2.0;
t5709 = t5666.*7.26350610236655e-5;
t5710 = t5666.*4.20092050615074e-6;
t5725 = t58.*t5666;
t5729 = t76.*t5666;
t5730 = t84.*t5666;
t5734 = t71.*t5666;
t5737 = t75.*t5666;
t5744 = t5666.*3.146556677756745e-13;
t5752 = -t5746;
t5755 = t5666.*4.126305279697715e-13;
t5756 = t142.*t5666;
t5766 = t151.*t5666;
t5769 = (t640.*t5622)./2.0;
t5783 = t5682./6.582018229284824e+63;
t5791 = -t5788;
t5798 = t5682.*2.060956449549905e-68;
t5799 = t5682.*9.397632428359433e-69;
t5800 = t5682.*4.040985049072001e-70;
t5802 = t5682.*2.672078334207073e-72;
t5805 = t5682.*3.835762748795343e-73;
t5839 = t4199+t5624;
t5841 = (t4742.*t5622)./2.0;
t5847 = (t1460.*t5776)./2.0;
t5848 = -t5845;
t5855 = t4.*t5852;
t5856 = t5.*t5852;
t5857 = t8.*t5852;
t5858 = t9.*t5852;
t5865 = t8.*t5862;
t5866 = t8.*t5863;
t5878 = t8.*t5873;
t5879 = t8.*t5874;
t5897 = -t5896;
t5900 = -t5899;
t5904 = -t5902;
t5907 = -t5906;
t5908 = t5881.*1.33637579258949e-4;
t5910 = t5881.*7.26735e-3;
t5913 = t5881.*7.26350610236655e-5;
t5915 = t5881.*2.180205e-5;
t5926 = (t594.*t5872)./2.0;
t5929 = t5622.*t5657.*2.0;
t5937 = (t1471.*t5872)./2.0;
t5941 = t5622.*t5657.*2.67275158517898e-4;
t5942 = t5622.*t5657.*1.45270122047331e-4;
t5943 = t5622.*t5657.*8.40184101230148e-6;
t5944 = t5622.*t5657.*6.293113355513489e-13;
t5945 = t5930.*1.33637579258949e-4;
t5946 = t5930.*7.26735e-3;
t5947 = t5930.*7.26350610236655e-5;
t5949 = t5622.*t5657.*8.252610559395431e-13;
t5951 = (t2121.*t5872)./2.0;
t5961 = t5622.*t5784;
t5968 = (t3443.*t5872)./2.0;
t5973 = (t3515.*t5872)./2.0;
t5974 = -t5972;
t5983 = t4.*t4119.*t5872;
t5990 = t5657.*t5776;
t5991 = -t5984;
t5997 = t4528.*t5872;
t6004 = -t6003;
t6008 = t5.*t6005;
t6009 = t9.*t6005;
t6010 = -t6005;
t6018 = t5679.*(t2088-t4743).*(-3.038581678643136e-64);
t6020 = t4966.*t5872;
t6022 = t5984.*7.26350610236655e-5;
t6023 = t5984.*1.246862701090643e-6;
t6027 = t5984.*1.744166498897461e-6;
t6035 = t5984.*2.179051830709965e-7;
t6048 = t5359.*t5872;
t6050 = t5984.*1.40259855e-11;
t6053 = t5984.*4.126305279697715e-13;
t6067 = t6005.*1.33637579258949e-4;
t6068 = t6005.*7.26735e-3;
t6072 = t6005.*7.26350610236655e-5;
t6073 = t5701.*t5784;
t6081 = t5707.*t5784;
t6082 = t5679.*(t2088-t4743).*(-1.879526485671887e-68);
t6084 = t5679.*(t2088-t4743).*(-4.121912899099809e-68);
t6087 = t5679.*(t2088-t4743).*(-8.081970098144003e-70);
t6088 = t5679.*(t2088-t4743).*(-5.344156668414146e-72);
t6089 = t5679.*(t2088-t4743).*(-7.671525497590686e-73);
t6092 = t5745.*t5784;
t6093 = t5746.*t5784;
t6104 = -t6102;
t6107 = -t6106;
t6110 = t5776.*t5784;
t6111 = -t6109;
t6113 = t5622.*t5872;
t6115 = -t5622.*(t4148+t5.*(t2421-t4158));
t6118 = t5622.*(t4148+t5.*(t2421-t4158));
t6120 = t5630.*t5872;
t6121 = -t6119;
t6125 = -t6124;
t6127 = (t5622.*t5887)./2.0;
t6128 = t6109.*7.26735e-3;
t6130 = t6109.*7.26350610236655e-5;
t6133 = t6109.*1.40259855e-11;
t6191 = t5657.*t5872;
t6192 = -t5872.*(t2421-t4158);
t6196 = t5872.*(t2421-t4158);
t6202 = -t6201;
t6222 = t5696+t5869;
t6229 = t6197.*(-1.33637579258949e-4);
t6230 = t5698+t5876;
t6236 = t6197.*(-7.26350610236655e-5);
t6240 = t6197.*7.26350610236655e-5;
t6243 = t6197.*(-1.246862701090643e-6);
t6245 = t6197.*(-3.383302988283333e-6);
t6247 = t6197.*(-1.744166498897461e-6);
t6248 = t6197.*1.246862701090643e-6;
t6250 = t6197.*1.744166498897461e-6;
t6261 = t6197.*(-3.146556677756745e-13);
t6263 = t6197.*(-1.40259855e-11);
t6264 = t6197.*3.146556677756745e-13;
t6265 = t6197.*(-4.126305279697715e-13);
t6266 = t6197.*1.40259855e-11;
t6268 = t6197.*4.126305279697715e-13;
t6270 = -t6269;
t6272 = t6215.*1.33637579258949e-4;
t6274 = t6215.*7.26735e-3;
t6277 = t6215.*7.26350610236655e-5;
t6313 = t5784.*t5872;
t6353 = t5852.*(t3136-t5691).*-2.0;
t6361 = -t6360;
t6363 = t5872.*t5903;
t6385 = -t6381;
t6408 = -t6406;
t6418 = t5814+t6101;
t6420 = t5819+t6105;
t6422 = t4141+t5860+t5871;
t6432 = -t6431;
t6435 = -t6433;
t6547 = -t6546;
t6549 = -t6548;
t6555 = -t6553;
t6556 = -t6554;
t6558 = t1589+t1644+t3638+t3703+t4287+t5704+t5707;
t6561 = -t6559;
t6569 = -t6568;
t6640 = t5824.*(t29-t30).*(t6105-t9.*((t197.*(t29-t30))./9.007199254740992e+15+t3.*(t3219-t3230))).*(-7.596454196607839e-68);
t6641 = (t5824.*(t29-t30).*(t6106+t5.*((t197.*(t29-t30))./9.007199254740992e+15+t3.*(t3219-t3230))))./1.316403645856965e+67;
t6662 = t5824.*(t29-t30).*(t6105-t9.*((t197.*(t29-t30))./9.007199254740992e+15+t3.*(t3219-t3230))).*(-5.520609140571798e-70);
t6663 = t5824.*(t29-t30).*(t6105-t9.*((t197.*(t29-t30))./9.007199254740992e+15+t3.*(t3219-t3230))).*(-5.517689141340903e-72);
t6665 = t5824.*(t29-t30).*(t6106+t5.*((t197.*(t29-t30))./9.007199254740992e+15+t3.*(t3219-t3230))).*1.015171749786156e-71;
t6666 = t5824.*(t29-t30).*(t6106+t5.*((t197.*(t29-t30))./9.007199254740992e+15+t3.*(t3219-t3230))).*5.520609140571798e-70;
t6669 = t5824.*(t29-t30).*(t6105-t9.*((t197.*(t29-t30))./9.007199254740992e+15+t3.*(t3219-t3230))).*(-1.065477564130357e-78);
t6670 = t5824.*(t29-t30).*(t6105-t9.*((t197.*(t29-t30))./9.007199254740992e+15+t3.*(t3219-t3230))).*1.065477564130357e-78;
t6671 = t5824.*(t29-t30).*(t6106+t5.*((t197.*(t29-t30))./9.007199254740992e+15+t3.*(t3219-t3230))).*1.065477564130357e-78;
t6700 = t779+t1639+t1787+t3408+t3700+t3840+t4284+t4508+t4966+t5410+t5426;
t6776 = t778+t1643+t1788+t3245+t3398+t3455+t3839+t3841+t4433+t5049+t5745;
t6896 = -t6895;
t6940 = t5773+t6340+t6344;
t7015 = (t5782.*t6832)./2.0;
t7027 = t3314+t5163+t6994;
t7031 = t5894.*(t5770+t5852.*(t3136-t5691).*2.0+t5861.*(t7.*(t3719-t3788)+(t3.*t34.*t191.*(t29-t30))./8.112963841460668e+31).*2.0).*(-1.0./2.0);
t7034 = (t9.*t7033)./2.0;
t7035 = (t5.*t7032)./2.0;
t7039 = (t1429.*t7032)./2.0;
t7040 = (t1427.*t7033)./2.0;
t7042 = t1318+t1521+t1666+t2280+t2400+t3472+t3602+t3652+t3742+t3750+t4074+t4091+t4235+t4719+t5403+t5714+t5727;
t7045 = t1268+t1591+t1857+t2285+t2402+t3559+t3705+t3756+t3811+t3868+t4075+t4093+t4295+t4699+t5418+t5711+t5723;
t7047 = (t9.*t7046)./2.0;
t7055 = (t1427.*t7046)./2.0;
t7062 = t802+t914+t1611+t1641+t1935+t2033+t3274+t3388+t3391+t3440+t3484+t3715+t3931+t3950+t3965+t4421+t4503+t5299+t5748+t5763;
et3 = t741+t868+t1568+t1834-t3274-t3391-t3440+t3874+t3891+t4348+t5259+t5742+t5757-t5.*t8.*1.133811468776912e-7;
et4 = t5.*t201.*(-6.364473664374288e-6)+t8.*t3365+t8.*t3449;
et5 = t4.*t5.*t7.*(-1.907069379620846e-7);
et6 = t8.*t9.*t190.*(-6.800564119502148e-6);
et7 = t3.*t4.*t5.*t34.*t191.*(-7.138318981153782e-22);
t7064 = t318.*(et3+et4+et5+et6+et7).*(-1.0./2.0);
t7071 = (t318.*t7065)./2.0;
t7083 = (t9.*t7082)./2.0;
t7086 = (t5.*t7085)./2.0;
t7088 = (t435.*t7082)./2.0;
t7089 = (t461.*t7082)./2.0;
t7091 = (t432.*t7085)./2.0;
t7093 = (t498.*t7085)./2.0;
t7095 = (t1427.*t7082)./2.0;
t7096 = (t1429.*t7085)./2.0;
t7100 = (t318.*t7098)./2.0;
t7107 = t7021.*(t5772+t5861.*((t197.*(t29-t30))./9.007199254740992e+15+t3.*(t3219-t3230)).*2.0+t5810.*(t3136-t5691).*2.0).*(-1.0./2.0);
t7108 = (t7021.*(t5772+t5861.*((t197.*(t29-t30))./9.007199254740992e+15+t3.*(t3219-t3230)).*2.0+t5810.*(t3136-t5691).*2.0))./2.0;
t7110 = t3.*t4.*t7109.*4.297799892626299e-1;
t7112 = t7021.*(t5770+t5852.*(t3136-t5691).*2.0+t5861.*(t7.*(t3719-t3788)+(t3.*t34.*t191.*(t29-t30))./8.112963841460668e+31).*2.0).*(-1.0./2.0);
t7113 = (t7021.*(t5770+t5852.*(t3136-t5691).*2.0+t5861.*(t7.*(t3719-t3788)+(t3.*t34.*t191.*(t29-t30))./8.112963841460668e+31).*2.0))./2.0;
t7115 = (t349.*t7109)./2.0;
t7140 = t2323+t2376+t2387+t2391+t2440+t2455+t4017+t4024+t4028+t4041+t4057+t4087+t4670+t4679+t4685+t4718+t7033;
t7141 = t2324+t2350+t2394+t2406+t2431+t2441+t4029+t4034+t4037+t4042+t4059+t4067+t4640+t4653+t4686+t4720+t7032;
t7159 = t1912+t2148+t2377+t2388+t2438+t2453+t3844+t3880+t4018+t4025+t4055+t4085+t4257+t4334+t4637+t4650+t4711+t4723+t7046;
t7199 = t1757+t1799+t1996+t2037+t2067+t2084+t2114+t2265+t3563+t3636+t3671+t3762+t3784+t3820+t3955+t3977+t4184+t4209+t4260+t4326+t4338+t4383+t4387+t4474+t7065;
t7248 = t1720+t1764+t2019+t2072+t2357+t2361+t2375+t2385+t2417+t2456+t3681+t3779+t3795+t3812+t4016+t4023+t4046+t4068+t4076+t4088+t4246+t4325+t4668+t4677+t4709+t4734+t7085;
t7297 = t1598+t1756+t1797+t1829+t1916+t1967+t1999+t2003+t2070+t2149+t2189+t2217+t3562+t3634+t3642+t3673+t3746+t3765+t3821+t3845+t3851+t3884+t3907+t3944+t4223+t4251+t4261+t4263+t4306+t4339+t4380+t4471+t7098;
t7306 = t1657+t1728+t1786+t1867+t1955+t1970+t1994+t2020+t2073+t2104+t2182+t2212+t3589+t3625+t3679+t3701+t3780+t3813+t3814+t3815+t3836+t3849+t3906+t3943+t4219+t4248+t4323+t4324+t4373+t4377+t4409+t4463+t7109;
t7560 = -t7559;
t7565 = dq1.*t7564;
t7577 = dq1.*t7576;
t7578 = dq4.*t7576;
t7580 = dq1.*t7579;
t7581 = dq3.*t7579;
t5654 = -t5651;
t5685 = t5683.^2;
t5717 = -t5709;
t5735 = t5676.*(-7.26350610236655e-5);
t5739 = t5676.*(-1.744166498897461e-6);
t5740 = t5676.*(-1.246862701090643e-6);
t5750 = -t5744;
t5761 = t5676.*1.40259855e-11;
t5762 = t5677.*1.40259855e-11;
t5840 = t4198+t5627;
t5864 = -t5855;
t5880 = -t5878;
t5911 = -t5908;
t5912 = -t5910;
t5914 = -t5913;
t5916 = -t5915;
t5922 = (t1471.*t5839)./2.0;
t5948 = -t5947;
t5952 = (t3515.*t5839)./2.0;
t5962 = -t5961;
t5975 = -t5973;
t5985 = t5961.*7.26735e-3;
t5986 = t5961.*1.33637579258949e-4;
t5992 = t5961.*7.26350610236655e-5;
t5995 = -t5990;
t6016 = -t6008;
t6019 = t5681.*t5683.*3.038581678643136e-64;
t6021 = t5990.*1.33637579258949e-4;
t6024 = t5983.*3.383302988283333e-6;
t6026 = t5983.*4.00912737776847e-7;
t6028 = -t6022;
t6029 = t5983.*1.246862701090643e-6;
t6030 = -t6023;
t6032 = -t6027;
t6033 = t5990.*1.246862701090643e-6;
t6034 = t5990.*3.383302988283333e-6;
t6037 = t5990.*4.00912737776847e-7;
t6042 = -t6035;
t6049 = t5983.*1.40259855e-11;
t6051 = t5983.*(-3.146556677756745e-13);
t6052 = t5997.*1.33637579258949e-4;
t6054 = t5997.*7.26735e-3;
t6055 = -t6050;
t6056 = t5990.*3.146556677756745e-13;
t6057 = -t6053;
t6059 = t5990.*1.40259855e-11;
t6074 = t6008.*7.26735e-3;
t6076 = t6009.*7.26735e-3;
t6078 = -t6072;
t6083 = t5997.*1.40259855e-11;
t6085 = t6008.*(-7.26350610236655e-5);
t6090 = t5681.*t5683.*1.879526485671887e-68;
t6091 = t5681.*t5683.*4.121912899099809e-68;
t6094 = t6008.*(-1.40259855e-11);
t6095 = t5681.*t5683.*8.081970098144003e-70;
t6096 = t5681.*t5683.*5.344156668414146e-72;
t6097 = t5681.*t5683.*7.671525497590686e-73;
t6114 = t5657.*t5839;
t6122 = t5683.*(t197.*(t29-t30).*9.007199254740992e+15+t3.*(t2444-t2449)).*(-3.038581678643136e-64);
t6129 = -t6128;
t6131 = t6110.*1.33637579258949e-4;
t6132 = t6110.*7.26735e-3;
t6134 = -t6133;
t6135 = t6110.*1.40259855e-11;
t6137 = t6113.*1.33637579258949e-4;
t6142 = t6113.*4.00912737776847e-7;
t6143 = t6113.*1.246862701090643e-6;
t6145 = t6113.*3.383302988283333e-6;
t6148 = t6118.*(-7.26350610236655e-5);
t6153 = t6118.*(-1.744166498897461e-6);
t6154 = t6118.*7.26350610236655e-5;
t6157 = t6118.*(-1.246862701090643e-6);
t6161 = t6118.*1.744166498897461e-6;
t6165 = t6118.*(-2.179051830709965e-7);
t6166 = t5683.*(t197.*(t29-t30).*9.007199254740992e+15+t3.*(t2444-t2449)).*(-4.121912899099809e-68);
t6167 = t6120.*1.33637579258949e-4;
t6168 = t5683.*(t197.*(t29-t30).*9.007199254740992e+15+t3.*(t2444-t2449)).*(-1.879526485671887e-68);
t6169 = t6120.*7.26735e-3;
t6170 = t6113.*3.146556677756745e-13;
t6171 = t6113.*1.40259855e-11;
t6174 = t5683.*(t197.*(t29-t30).*9.007199254740992e+15+t3.*(t2444-t2449)).*(-8.081970098144003e-70);
t6178 = t5683.*(t197.*(t29-t30).*9.007199254740992e+15+t3.*(t2444-t2449)).*(-5.344156668414146e-72);
t6181 = t6118.*(-1.40259855e-11);
t6184 = t5683.*(t197.*(t29-t30).*9.007199254740992e+15+t3.*(t2444-t2449)).*(-7.671525497590686e-73);
t6186 = t6118.*1.40259855e-11;
t6189 = t6118.*(-4.126305279697715e-13);
t6190 = t6118.*4.126305279697715e-13;
t6194 = t6120.*1.40259855e-11;
t6213 = t5692+t5857;
t6214 = t5784.*t5839;
t6221 = t6191.*1.33637579258949e-4;
t6224 = t6196.*(-1.33637579258949e-4);
t6225 = t6191.*7.26350610236655e-5;
t6228 = t6196.*1.33637579258949e-4;
t6231 = t6191.*1.246862701090643e-6;
t6232 = t6191.*3.383302988283333e-6;
t6233 = t5.*t6222;
t6234 = t9.*t6222;
t6235 = t6191.*1.744166498897461e-6;
t6237 = t6196.*(-1.246862701090643e-6);
t6238 = t6196.*(-3.383302988283333e-6);
t6239 = t6230.^2;
t6242 = t6196.*1.246862701090643e-6;
t6244 = t6196.*3.383302988283333e-6;
t6254 = t6191.*3.146556677756745e-13;
t6255 = t6191.*1.40259855e-11;
t6257 = t6196.*(-3.146556677756745e-13);
t6258 = t6191.*4.126305279697715e-13;
t6259 = t6196.*(-1.40259855e-11);
t6260 = t6196.*3.146556677756745e-13;
t6262 = t6196.*1.40259855e-11;
t6320 = -t6313;
t6332 = t6313.*1.33637579258949e-4;
t6333 = t6313.*7.26735e-3;
t6336 = t6313.*7.26350610236655e-5;
t6345 = t6313.*1.40259855e-11;
t6355 = t5856+t5866;
t6356 = t5858+t5875;
t6357 = t5868+t5879;
t6365 = -t6363;
t6368 = t6363.*1.33637579258949e-4;
t6369 = t6363.*7.26735e-3;
t6392 = t6363.*1.40259855e-11;
t6414 = t4838.*t6230.*(t29-t30).*(-7.596454196607839e-68);
t6415 = (t4838.*t6230.*(t29-t30))./1.316403645856965e+67;
t6419 = t5813+t6104;
t6421 = t5818+t6107;
t6428 = t4838.*t6230.*(t29-t30).*(-1.015171749786156e-71);
t6429 = t4838.*t6230.*(t29-t30).*(-5.520609140571798e-70);
t6430 = t4838.*t6230.*(t29-t30).*(-5.517689141340903e-72);
t6434 = t4838.*t6230.*(t29-t30).*(-1.656182742171539e-72);
t6439 = t5684.*t6230.*(t29-t30).*(-7.596454196607839e-68);
t6452 = t5684.*t6230.*(t29-t30).*(-1.015171749786156e-71);
t6453 = t5684.*t6230.*(t29-t30).*(-5.520609140571798e-70);
t6454 = t5684.*t6230.*(t29-t30).*(-5.517689141340903e-72);
t6455 = t5684.*t6230.*(t29-t30).*5.517689141340903e-72;
t6467 = t4.*t5861.*t6230.*2.0;
t6478 = t5822.*t6230.*(t29-t30).*(-7.596454196607839e-68);
t6481 = t4.*t5861.*t6230.*2.67275158517898e-4;
t6483 = t4.*t5861.*t6230.*1.45270122047331e-4;
t6487 = t4.*t5861.*t6230.*8.40184101230148e-6;
t6494 = t5824.*t6222.*(t29-t30).*(-7.596454196607839e-68);
t6495 = (t5824.*t6222.*(t29-t30))./1.316403645856965e+67;
t6496 = t4.*t5861.*t6230.*6.293113355513489e-13;
t6497 = t5824.*t6230.*(t29-t30).*(-7.596454196607839e-68);
t6501 = t4.*t5861.*t6230.*8.252610559395431e-13;
t6502 = (t9.*t5824.*t6230.*(t29-t30))./1.316403645856965e+67;
t6508 = t5822.*t6230.*(t29-t30).*(-5.520609140571798e-70);
t6509 = t5822.*t6230.*(t29-t30).*(-1.015171749786156e-71);
C_dq = ft_13({dq1,dq2,dq3,dq4,dq5,dq6,t1004,t1016,t1019,t1020,t1031,t1039,t1046,t1050,t1056,t1061,t1069,t1075,t1076,t1077,t1081,t1083,t1088,t1090,t1095,t1099,t1101,t1106,t1108,t112,t1122,t113,t1133,t1144,t1146,t1147,t115,t1150,t1152,t1155,t1156,t1158,t116,t1165,t1170,t1171,t1174,t1177,t1179,t1184,t1185,t1191,t1193,t1194,t1196,t1201,t1203,t1205,t1207,t121,t1211,t1212,t1213,t1215,t1221,t1224,t1225,t1227,t1228,t1233,t1245,t125,t1250,t1253,t1254,t1258,t1273,t1274,t1282,t1285,t1288,t1292,t1300,t1301,t1306,t131,t1316,t132,t1322,t1323,t1324,t133,t1330,t1331,t1333,t1337,t1342,t1344,t1345,t1348,t1353,t1365,t1377,t1379,t1380,t1383,t1388,t139,t1391,t1402,t1407,t1409,t1411,t1413,t1419,t142,t1423,t1426,t1427,t1428,t1429,t1436,t144,t1440,t1441,t1443,t1445,t1446,t1449,t1454,t1457,t1458,t1460,t1471,t148,t1486,t1487,t1488,t1489,t1493,t1494,t1495,t1496,t1498,t1499,t15,t150,t1503,t1508,t151,t1511,t1517,t1520,t1523,t1524,t1526,t1530,t1531,t1533,t1534,t1536,t1537,t1538,t1540,t1541,t1542,t1548,t1550,t1551,t156,t1567,t1568,t1570,t1574,t1577,t1578,t158,t1581,t1582,t1584,t1585,t1586,t1587,t1590,t1592,t1593,t1594,t1598,t16,t1600,t1601,t1602,t1605,t1606,t1607,t1609,t1612,t1613,t1614,t1615,t1616,t1617,t1619,t1620,t1621,t1622,t1625,t1627,t1628,t1630,t1636,t1642,t1647,t1648,t1651,t1655,t1656,t1659,t166,t1660,t1661,t1663,t1667,t1670,t1672,t1674,t1681,t1683,t1687,t1692,t1697,t1699,t17,t1700,t1701,t1704,t1705,t1706,t1707,t1708,t171,t1710,t1715,t1716,t1718,t1719,t1721,t1724,t1731,t1732,t1734,t1735,t1736,t1740,t1745,t1747,t1748,t1753,t1754,t1756,t1758,t1759,t1760,t1761,t1762,t1763,t1766,t1767,t1769,t1770,t1771,t1772,t1775,t1776,t1777,t1779,t1781,t1783,t1784,t1792,t1793,t1794,t1795,t1797,t1798,t18,t1800,t1805,t1806,t1807,t1808,t1809,t1811,t1812,t1814,t1815,t1816,t1820,t1821,t1823,t1827,t1828,t1829,t183,t1831,t1833,t1834,t1835,t1836,t1839,t1847,t1849,t185,t1855,t1856,t1858,t1860,t1861,t1863,t1868,t1870,t1873,t1878,t1882,t1884,t1886,t1892,t1896,t1899,t19,t190,t1900,t1902,t1906,t1908,t1909,t191,t1913,t1916,t1917,t1922,t1925,t1930,t1937,t1938,t1941,t1942,t1946,t1947,t1951,t1952,t196,t1961,t1967,t1968,t1969,t197,t1974,t1977,t1981,t1983,t1984,t1985,t1986,t1989,t199,t1992,t1993,t1995,t1997,t1998,t1999,t2,t20,t200,t2002,t2003,t2004,t2006,t2008,t201,t2014,t2015,t2017,t202,t2026,t2027,t2028,t2034,t2035,t2036,t2038,t2039,t2043,t2047,t2050,t2052,t2053,t206,t2060,t2062,t2066,t2068,t2069,t207,t2070,t2075,t2076,t2077,t2079,t2081,t2083,t2085,t2088,t2091,t2096,t2098,t21,t2100,t2106,t2110,t2113,t2115,t2116,t2118,t2119,t2121,t2123,t2128,t2130,t2132,t2133,t2134,t2136,t2142,t2143,t2145,t2149,t2150,t2154,t2158,t2164,t2165,t2176,t2177,t2178,t2180,t2181,t2184,t2186,t2187,t2189,t2191,t2192,t2193,t2196,t2197,t2199,t22,t2200,t2202,t2203,t2208,t2211,t2213,t2214,t2217,t2220,t2223,t2224,t2234,t2236,t2239,t224,t2243,t225,t2253,t2256,t2257,t2266,t2267,t227,t228,t2284,t2289,t2291,t2296,t2298,t2299,t23,t230,t2300,t2303,t2304,t231,t2312,t2314,t2315,t2320,t2326,t2328,t233,t2330,t2333,t2334,t2338,t234,t2341,t2342,t235,t2358,t2359,t236,t2362,t2364,t2383,t2390,t2392,t2395,t2396,t2397,t2398,t24,t240,t2416,t2420,t2421,t2424,t243,t2435,t2439,t244,t2443,t2444,t2449,t2452,t2454,t2465,t2466,t2474,t2481,t2483,t2486,t249,t2490,t2494,t2497,t2502,t2507,t2523,t2524,t2525,t2530,t2539,t2544,t2546,t2548,t2549,t2552,t2553,t2554,t2555,t2556,t2560,t2562,t2563,t2564,t2565,t2566,t2567,t2568,t2569,t257,t2570,t2571,t2574,t2575,t2576,t2577,t2578,t2579,t258,t2588,t2589,t2597,t2598,t2599,t2611,t2612,t2615,t2617,t2627,t263,t2640,t2641,t2655,t2656,t266,t2666,t2684,t2686,t2689,t2692,t2694,t2695,t270,t2706,t2720,t2722,t2724,t2725,t2726,t273,t2737,t274,t2740,t2741,t2743,t2744,t2748,t2749,t275,t2750,t2752,t2753,t2754,t2755,t2757,t2759,t276,t2760,t2761,t2764,t277,t2771,t2772,t2775,t2778,t278,t2780,t2783,t2785,t2791,t2792,t2793,t2795,t2797,t2798,t2799,t280,t2800,t2801,t2802,t2805,t2806,t2807,t2812,t2815,t2816,t2817,t2818,t2824,t2825,t2827,t2833,t2835,t284,t2851,t2857,t2861,t2868,t287,t2872,t2877,t2880,t2881,t2887,t2889,t2893,t2895,t2896,t29,t290,t2905,t2906,t291,t2911,t2913,t2915,t2916,t2918,t292,t2921,t2922,t2932,t2933,t294,t2941,t2944,t2956,t2958,t2965,t297,t2973,t2977,t2987,t299,t2999,t3,t30,t300,t302,t303,t304,t3047,t305,t306,t3065,t3080,t3083,t3088,t309,t3095,t3096,t310,t311,t3117,t3125,t3129,t313,t3136,t314,t3142,t315,t3159,t316,t3164,t3166,t3168,t318,t319,t320,t3200,t3209,t3213,t3219,t322,t3222,t3224,t3230,t3239,t324,t3247,t325,t3266,t3268,t3274,t328,t3309,t3321,t333,t3338,t336,t3365,t3368,t3369,t337,t3371,t3375,t3378,t3380,t3383,t3387,t3390,t3391,t3392,t3397,t34,t340,t3400,t3405,t3407,t3409,t3416,t3417,t3418,t3420,t3421,t3422,t3426,t3429,t3430,t3432,t3434,t3435,t3436,t3437,t3439,t344,t3440,t3441,t3443,t3444,t3445,t3446,t3449,t3450,t3453,t3457,t3458,t346,t3462,t3463,t3464,t3465,t3468,t3469,t347,t3471,t3472,t3474,t3475,t3476,t3479,t348,t3480,t3483,t3485,t3489,t349,t3490,t3491,t3492,t3493,t3496,t3498,t3499,t350,t3500,t3501,t3504,t3506,t3507,t3510,t3511,t3513,t3514,t3515,t3517,t3518,t352,t3521,t3522,t3523,t3526,t353,t3530,t3531,t3532,t3535,t3536,t3539,t3540,t3542,t3543,t3547,t3554,t3556,t3557,t356,t3562,t3565,t3568,t3569,t357,t3571,t3572,t3574,t3577,t3578,t358,t3582,t3583,t3584,t3585,t359,t3592,t3593,t3605,t3606,t3607,t361,t3610,t3611,t3612,t3617,t3618,t362,t3634,t3635,t3637,t3640,t3642,t3644,t3648,t365,t3656,t3658,t3659,t3662,t3666,t3667,t3668,t3672,t3673,t3676,t3678,t368,t3682,t369,t3694,t3702,t3706,t3708,t371,t3717,t3719,t372,t3725,t3726,t373,t3732,t3733,t3734,t3738,t374,t3743,t3746,t3752,t3753,t3754,t3755,t3757,t3759,t3761,t3763,t3764,t3765,t3767,t377,t3772,t378,t3781,t3783,t3785,t3788,t379,t3792,t380,t3818,t3819,t382,t3821,t3822,t3823,t3824,t3831,t3833,t3835,t3838,t384,t3843,t3845,t3851,t3852,t3853,t386,t3863,t3869,t387,t3871,t3873,t3874,t3875,t3876,t388,t3882,t3884,t3889,t3890,t3891,t3892,t3904,t3907,t391,t3910,t3913,t3915,t392,t3921,t3922,t3923,t3940,t3944,t395,t3951,t3954,t3956,t3957,t3959,t396,t3960,t3968,t3969,t3971,t3972,t3976,t3978,t3979,t3992,t3993,t3995,t3997,t4,t400,t4000,t4004,t4008,t401,t4010,t4011,t4014,t4015,t402,t403,t4047,t4050,t4053,t4056,t406,t4069,t4070,t4083,t4086,t4089,t4099,t410,t4100,t4103,t4108,t411,t4113,t4115,t4118,t4119,t412,t4121,t4123,t4126,t413,t4132,t4134,t4138,t414,t4143,t4146,t4148,t4149,t415,t4152,t4153,t4154,t4158,t416,t4161,t4166,t417,t4173,t4178,t4179,t418,t4181,t4183,t4185,t4186,t4190,t4196,t4197,t420,t4206,t4208,t4210,t4211,t4217,t422,t4221,t4223,t4226,t4228,t423,t4230,t4232,t4234,t424,t4243,t4249,t425,t4250,t4251,t4254,t4255,t4256,t4259,t4261,t4263,t427,t4274,t4276,t4278,t4279,t428,t4285,t4286,t429,t4293,t4298,t4301,t4304,t4305,t4306,t431,t4315,t4317,t4318,t432,t4327,t4329,t433,t4332,t4333,t4335,t4337,t4339,t434,t4342,t4344,t4345,t4347,t4348,t4349,t435,t4350,t436,t4368,t4369,t437,t4370,t4371,t4378,t438,t4380,t4382,t4385,t4388,t439,t4392,t4394,t4395,t4396,t4397,t44,t440,t4402,t4403,t4405,t4406,t4407,t441,t4410,t4412,t4413,t4414,t4416,t4417,t4418,t4419,t442,t4420,t4423,t4425,t4426,t4427,t4428,t4429,t4431,t4436,t4437,t444,t4440,t4444,t4446,t4447,t4449,t445,t4450,t4453,t4460,t4462,t4467,t4468,t4469,t4471,t4473,t4475,t4478,t4479,t448,t4482,t4483,t4485,t4486,t4487,t4488,t4489,t449,t4490,t4494,t4495,t4498,t4499,t45,t450,t4500,t4501,t4502,t4505,t4506,t4509,t4510,t4515,t4518,t4519,t452,t4520,t4521,t4522,t4523,t4526,t4527,t4528,t453,t4530,t4534,t4536,t4538,t454,t4541,t4543,t4545,t4546,t4549,t4551,t4552,t4553,t4556,t4557,t4558,t4559,t4565,t4568,t457,t4570,t4572,t4575,t4577,t4578,t458,t4581,t4582,t4586,t4587,t4588,t4589,t459,t4590,t4591,t4592,t4593,t4595,t4596,t4597,t4598,t460,t4600,t4601,t4602,t4604,t4605,t4606,t4607,t4608,t461,t4614,t4616,t4619,t462,t4621,t4622,t4623,t4624,t4625,t4626,t4629,t463,t4633,t4634,t4636,t464,t4644,t4645,t4647,t4648,t465,t4654,t4656,t4659,t466,t4660,t4666,t4667,t4669,t4673,t4674,t4675,t4678,t468,t4682,t4683,t4684,t469,t4694,t4695,t4696,t4697,t47,t470,t4707,t4708,t471,t4714,t4717,t472,t4724,t4727,t4728,t4731,t4732,t4733,t4737,t4738,t4739,t4742,t4743,t4745,t4747,t4748,t475,t4755,t4756,t4762,t4763,t477,t4773,t4775,t4780,t4781,t4782,t4783,t4785,t4786,t479,t480,t4803,t481,t4810,t4811,t482,t4824,t4825,t4826,t483,t4837,t4838,t4842,t4846,t485,t486,t4862,t4864,t4866,t4867,t4869,t4870,t488,t4884,t489,t4903,t4904,t491,t4911,t4914,t4919,t492,t4920,t4924,t4925,t4927,t4929,t493,t4934,t4936,t494,t4942,t4946,t4949,t4950,t4953,t4957,t496,t4964,t497,t4973,t4974,t498,t4981,t4983,t4984,t4987,t4988,t4989,t499,t4990,t4993,t4994,t4995,t4996,t5,t50,t500,t5000,t5002,t5007,t5008,t5009,t501,t5017,t502,t5020,t5021,t5022,t5023,t5024,t5026,t5027,t503,t5031,t5032,t5039,t504,t505,t5056,t5058,t506,t5061,t5063,t5064,t5065,t507,t5075,t5076,t508,t5080,t5083,t5084,t5086,t5087,t509,t5090,t5091,t5093,t5097,t5099,t510,t5100,t5102,t5107,t511,t5112,t5113,t5114,t512,t5121,t5123,t513,t5132,t5136,t5139,t514,t5140,t5144,t5145,t5147,t5150,t5151,t516,t5164,t5166,t517,t518,t5184,t5189,t5195,t520,t5202,t5203,t5204,t5206,t521,t5210,t5211,t5215,t5217,t5219,t522,t5227,t5228,t523,t5232,t5233,t5235,t5236,t5238,t524,t5242,t5244,t5249,t525,t5251,t5252,t5255,t5258,t5259,t526,t5260,t5262,t5269,t527,t5275,t5279,t528,t5280,t5285,t529,t5297,t53,t530,t5301,t5307,t531,t5314,t5316,t5318,t532,t5320,t5323,t5324,t533,t5333,t5335,t5337,t5339,t534,t5340,t5344,t535,t5354,t5356,t536,t5364,t537,t5370,t5372,t5373,t5375,t5378,t538,t5383,t5389,t539,t5390,t5391,t5392,t5393,t5394,t5395,t540,t5402,t5404,t5405,t5409,t5412,t5416,t5422,t5423,t543,t5431,t544,t5443,t5447,t545,t5450,t5457,t5459,t546,t5464,t5465,t5466,t547,t548,t5480,t5482,t5483,t5484,t5486,t5487,t5488,t549,t5507,t551,t5515,t552,t5521,t553,t554,t555,t556,t557,t558,t559,t560,t5602,t5605,t561,t5616,t5617,t5619,t562,t5620,t5621,t5622,t5623,t5626,t5628,t563,t5633,t5634,t5636,t5638,t5639,t564,t5642,t5644,t5645,t5646,t5647,t5648,t5650,t5652,t5654,t5655,t5657,t5658,t5662,t5665,t5666,t567,t5670,t5676,t5677,t5679,t568,t5683,t5684,t5685,t5688,t569,t5691,t5694,t5699,t57,t570,t5700,t5702,t5704,t5706,t5708,t5709,t571,t5710,t5717,t5718,t572,t5729,t573,t5730,t5735,t5738,t5739,t574,t5740,t5742,t5744,t5750,t5752,t5755,t5756,t5757,t576,t5761,t5762,t5766,t5769,t5770,t5771,t5772,t5774,t5775,t5776,t5778,t5779,t578,t5783,t5784,t5786,t5787,t5790,t5791,t5792,t5794,t5795,t5797,t5798,t5799,t58,t580,t5800,t5802,t5805,t5808,t5809,t581,t5810,t582,t5822,t5823,t5824,t5825,t5826,t5827,t5828,t5829,t5830,t5831,t5832,t5833,t5834,t5835,t5836,t5838,t5839,t584,t5840,t5841,t5842,t5843,t5844,t5845,t5846,t5847,t5848,t5849,t5850,t5851,t5852,t5859,t586,t5861,t5862,t5863,t5864,t587,t5870,t5872,t5873,t5874,t5878,t5879,t5880,t5881,t5882,t5883,t5884,t5885,t5888,t5889,t589,t5890,t5891,t5892,t5893,t5894,t5895,t5897,t5898,t5899,t590,t5900,t5901,t5904,t5905,t5907,t5909,t591,t5911,t5912,t5914,t5915,t5916,t5917,t5918,t5919,t592,t5920,t5922,t5925,t5926,t5928,t5929,t593,t5930,t5931,t5932,t5933,t5934,t5935,t5936,t5937,t5938,t5939,t594,t5940,t5941,t5942,t5943,t5944,t5945,t5946,t5947,t5948,t5949,t595,t5951,t5952,t5954,t5956,t5957,t5958,t5959,t596,t5960,t5961,t5962,t5964,t5965,t5966,t5967,t5968,t597,t5970,t5971,t5972,t5973,t5974,t5975,t5976,t5977,t5978,t5979,t5980,t5981,t5982,t5983,t5984,t5985,t5986,t5988,t5991,t5992,t5994,t5995,t5996,t5997,t5998,t5999,t6,t60,t600,t6000,t6001,t6002,t6003,t6004,t6005,t6007,t6008,t6009,t6010,t6011,t6012,t6013,t6014,t6016,t6017,t6018,t6019,t602,t6020,t6021,t6024,t6026,t6028,t6029,t603,t6030,t6032,t6033,t6034,t6035,t6037,t6038,t604,t6042,t6043,t6045,t6046,t6047,t6048,t6049,t605,t6051,t6052,t6053,t6054,t6055,t6056,t6057,t6059,t6060,t6061,t6062,t6064,t6065,t6067,t6068,t6069,t6073,t6074,t6075,t6076,t6077,t6078,t6079,t6081,t6082,t6083,t6084,t6085,t6086,t6087,t6088,t6089,t609,t6090,t6091,t6093,t6094,t6095,t6096,t6097,t610,t6103,t6105,t6106,t6108,t6109,t611,t6110,t6111,t6113,t6114,t6117,t6118,t6119,t612,t6120,t6121,t6122,t6123,t6125,t6126,t6127,t6128,t6129,t613,t6130,t6131,t6132,t6134,t6135,t6136,t6137,t6139,t614,t6140,t6142,t6143,t6145,t6149,t615,t6154,t6156,t6157,t616,t6161,t6163,t6165,t6166,t6167,t6168,t6169,t6170,t6171,t6174,t6175,t6178,t618,t6180,t6182,t6184,t6186,t6187,t6189,t619,t6190,t6191,t6194,t6195,t6196,t6197,t6199,t620,t6200,t6201,t6202,t6203,t6204,t6205,t6206,t6207,t6208,t6209,t621,t6210,t6211,t6212,t6213,t6214,t6215,t622,t6221,t6222,t6225,t6228,t6229,t623,t6230,t6231,t6232,t6233,t6234,t6235,t6239,t624,t6240,t6241,t6242,t6243,t6244,t6245,t6248,t6249,t625,t6250,t6251,t6254,t6255,t6258,t6260,t6262,t6264,t6266,t6267,t6268,t6270,t6271,t6272,t6274,t6276,t6277,t6280,t6313,t6319,t632,t6320,t6329,t6330,t6331,t6332,t6333,t6336,t6338,t6341,t6342,t6343,t6345,t6347,t6348,t6349,t6350,t6351,t6352,t6353,t6354,t6355,t6356,t6360,t6361,t6362,t6364,t6365,t6366,t6367,t6368,t6369,t6374,t6375,t6376,t6378,t6379,t638,t6380,t6382,t6385,t6386,t6387,t6388,t6390,t6391,t6392,t6393,t6395,t6396,t6397,t6398,t640,t6404,t6406,t6407,t6408,t6414,t6415,t6418,t6419,t6422,t6427,t6428,t6429,t6430,t6431,t6432,t6433,t6434,t6435,t6436,t6439,t6440,t6441,t6452,t6453,t6454,t6455,t6456,t6457,t6458,t6459,t6460,t6461,t6462,t6463,t6467,t6469,t6471,t6478,t6481,t6483,t6487,t6495,t6496,t6497,t6501,t6502,t6507,t6508,t6509,t6546,t6547,t6548,t6549,t6555,t6556,t6557,t6558,t6560,t6561,t6562,t6566,t6567,t6569,t6597,t6609,t6640,t6641,t6662,t6663,t6665,t6666,t6669,t6670,t6671,t6689,t6700,t6702,t6776,t681,t6826,t6827,t6832,t684,t6868,t6871,t6872,t6873,t6874,t6896,t6902,t6919,t6933,t6934,t6994,t7,t7000,t7010,t7011,t7012,t7015,t7019,t7020,t7026,t7027,t7031,t7032,t7033,t7034,t7035,t7039,t7040,t7042,t7043,t7044,t7045,t7046,t7047,t7052,t7055,t7060,t7061,t7062,t7064,t7065,t7071,t7079,t7080,t7082,t7083,t7085,t7086,t7087,t7088,t7089,t7091,t7093,t7095,t7096,t7098,t71,t7100,t7104,t7108,t7109,t7110,t7113,t7115,t7119,t712,t7140,t7141,t7148,t7149,t7153,t7159,t7199,t72,t724,t7244,t7248,t7256,t7258,t7297,t73,t7306,t7334,t7335,t7364,t738,t739,t741,t742,t75,t7528,t753,t7549,t7550,t7551,t7553,t7557,t7558,t7560,t7564,t7565,t7567,t7568,t7569,t7570,t7571,t7573,t7574,t7575,t7576,t7577,t7578,t7579,t7580,t7581,t76,t760,t781,t792,t796,t797,t8,t803,t81,t824,t825,t826,t827,t830,t832,t84,t845,t847,t848,t852,t856,t86,t861,t866,t868,t869,t874,t875,t877,t878,t881,t893,t899,t9,t90,t902,t903,t905,t908,t909,t91,t910,t911,t912,t915,t917,t919,t922,t925,t926,t928,t929,t930,t931,t932,t934,t940,t944,t945,t947,t95,t952,t954,t955,t957,t958,t968,t970,t971,t972,t975,t976,t984,t985,t986,t989,t99,t991,t998});
end
function C_dq = ft_13(ct)
dq1 = ct{1};
dq2 = ct{2};
dq3 = ct{3};
dq4 = ct{4};
dq5 = ct{5};
dq6 = ct{6};
t1004 = ct{7};
t1016 = ct{8};
t1019 = ct{9};
t1020 = ct{10};
t1031 = ct{11};
t1039 = ct{12};
t1046 = ct{13};
t1050 = ct{14};
t1056 = ct{15};
t1061 = ct{16};
t1069 = ct{17};
t1075 = ct{18};
t1076 = ct{19};
t1077 = ct{20};
t1081 = ct{21};
t1083 = ct{22};
t1088 = ct{23};
t1090 = ct{24};
t1095 = ct{25};
t1099 = ct{26};
t1101 = ct{27};
t1106 = ct{28};
t1108 = ct{29};
t112 = ct{30};
t1122 = ct{31};
t113 = ct{32};
t1133 = ct{33};
t1144 = ct{34};
t1146 = ct{35};
t1147 = ct{36};
t115 = ct{37};
t1150 = ct{38};
t1152 = ct{39};
t1155 = ct{40};
t1156 = ct{41};
t1158 = ct{42};
t116 = ct{43};
t1165 = ct{44};
t1170 = ct{45};
t1171 = ct{46};
t1174 = ct{47};
t1177 = ct{48};
t1179 = ct{49};
t1184 = ct{50};
t1185 = ct{51};
t1191 = ct{52};
t1193 = ct{53};
t1194 = ct{54};
t1196 = ct{55};
t1201 = ct{56};
t1203 = ct{57};
t1205 = ct{58};
t1207 = ct{59};
t121 = ct{60};
t1211 = ct{61};
t1212 = ct{62};
t1213 = ct{63};
t1215 = ct{64};
t1221 = ct{65};
t1224 = ct{66};
t1225 = ct{67};
t1227 = ct{68};
t1228 = ct{69};
t1233 = ct{70};
t1245 = ct{71};
t125 = ct{72};
t1250 = ct{73};
t1253 = ct{74};
t1254 = ct{75};
t1258 = ct{76};
t1273 = ct{77};
t1274 = ct{78};
t1282 = ct{79};
t1285 = ct{80};
t1288 = ct{81};
t1292 = ct{82};
t1300 = ct{83};
t1301 = ct{84};
t1306 = ct{85};
t131 = ct{86};
t1316 = ct{87};
t132 = ct{88};
t1322 = ct{89};
t1323 = ct{90};
t1324 = ct{91};
t133 = ct{92};
t1330 = ct{93};
t1331 = ct{94};
t1333 = ct{95};
t1337 = ct{96};
t1342 = ct{97};
t1344 = ct{98};
t1345 = ct{99};
t1348 = ct{100};
t1353 = ct{101};
t1365 = ct{102};
t1377 = ct{103};
t1379 = ct{104};
t1380 = ct{105};
t1383 = ct{106};
t1388 = ct{107};
t139 = ct{108};
t1391 = ct{109};
t1402 = ct{110};
t1407 = ct{111};
t1409 = ct{112};
t1411 = ct{113};
t1413 = ct{114};
t1419 = ct{115};
t142 = ct{116};
t1423 = ct{117};
t1426 = ct{118};
t1427 = ct{119};
t1428 = ct{120};
t1429 = ct{121};
t1436 = ct{122};
t144 = ct{123};
t1440 = ct{124};
t1441 = ct{125};
t1443 = ct{126};
t1445 = ct{127};
t1446 = ct{128};
t1449 = ct{129};
t1454 = ct{130};
t1457 = ct{131};
t1458 = ct{132};
t1460 = ct{133};
t1471 = ct{134};
t148 = ct{135};
t1486 = ct{136};
t1487 = ct{137};
t1488 = ct{138};
t1489 = ct{139};
t1493 = ct{140};
t1494 = ct{141};
t1495 = ct{142};
t1496 = ct{143};
t1498 = ct{144};
t1499 = ct{145};
t15 = ct{146};
t150 = ct{147};
t1503 = ct{148};
t1508 = ct{149};
t151 = ct{150};
t1511 = ct{151};
t1517 = ct{152};
t1520 = ct{153};
t1523 = ct{154};
t1524 = ct{155};
t1526 = ct{156};
t1530 = ct{157};
t1531 = ct{158};
t1533 = ct{159};
t1534 = ct{160};
t1536 = ct{161};
t1537 = ct{162};
t1538 = ct{163};
t1540 = ct{164};
t1541 = ct{165};
t1542 = ct{166};
t1548 = ct{167};
t1550 = ct{168};
t1551 = ct{169};
t156 = ct{170};
t1567 = ct{171};
t1568 = ct{172};
t1570 = ct{173};
t1574 = ct{174};
t1577 = ct{175};
t1578 = ct{176};
t158 = ct{177};
t1581 = ct{178};
t1582 = ct{179};
t1584 = ct{180};
t1585 = ct{181};
t1586 = ct{182};
t1587 = ct{183};
t1590 = ct{184};
t1592 = ct{185};
t1593 = ct{186};
t1594 = ct{187};
t1598 = ct{188};
t16 = ct{189};
t1600 = ct{190};
t1601 = ct{191};
t1602 = ct{192};
t1605 = ct{193};
t1606 = ct{194};
t1607 = ct{195};
t1609 = ct{196};
t1612 = ct{197};
t1613 = ct{198};
t1614 = ct{199};
t1615 = ct{200};
t1616 = ct{201};
t1617 = ct{202};
t1619 = ct{203};
t1620 = ct{204};
t1621 = ct{205};
t1622 = ct{206};
t1625 = ct{207};
t1627 = ct{208};
t1628 = ct{209};
t1630 = ct{210};
t1636 = ct{211};
t1642 = ct{212};
t1647 = ct{213};
t1648 = ct{214};
t1651 = ct{215};
t1655 = ct{216};
t1656 = ct{217};
t1659 = ct{218};
t166 = ct{219};
t1660 = ct{220};
t1661 = ct{221};
t1663 = ct{222};
t1667 = ct{223};
t1670 = ct{224};
t1672 = ct{225};
t1674 = ct{226};
t1681 = ct{227};
t1683 = ct{228};
t1687 = ct{229};
t1692 = ct{230};
t1697 = ct{231};
t1699 = ct{232};
t17 = ct{233};
t1700 = ct{234};
t1701 = ct{235};
t1704 = ct{236};
t1705 = ct{237};
t1706 = ct{238};
t1707 = ct{239};
t1708 = ct{240};
t171 = ct{241};
t1710 = ct{242};
t1715 = ct{243};
t1716 = ct{244};
t1718 = ct{245};
t1719 = ct{246};
t1721 = ct{247};
t1724 = ct{248};
t1731 = ct{249};
t1732 = ct{250};
t1734 = ct{251};
t1735 = ct{252};
t1736 = ct{253};
t1740 = ct{254};
t1745 = ct{255};
t1747 = ct{256};
t1748 = ct{257};
t1753 = ct{258};
t1754 = ct{259};
t1756 = ct{260};
t1758 = ct{261};
t1759 = ct{262};
t1760 = ct{263};
t1761 = ct{264};
t1762 = ct{265};
t1763 = ct{266};
t1766 = ct{267};
t1767 = ct{268};
t1769 = ct{269};
t1770 = ct{270};
t1771 = ct{271};
t1772 = ct{272};
t1775 = ct{273};
t1776 = ct{274};
t1777 = ct{275};
t1779 = ct{276};
t1781 = ct{277};
t1783 = ct{278};
t1784 = ct{279};
t1792 = ct{280};
t1793 = ct{281};
t1794 = ct{282};
t1795 = ct{283};
t1797 = ct{284};
t1798 = ct{285};
t18 = ct{286};
t1800 = ct{287};
t1805 = ct{288};
t1806 = ct{289};
t1807 = ct{290};
t1808 = ct{291};
t1809 = ct{292};
t1811 = ct{293};
t1812 = ct{294};
t1814 = ct{295};
t1815 = ct{296};
t1816 = ct{297};
t1820 = ct{298};
t1821 = ct{299};
t1823 = ct{300};
t1827 = ct{301};
t1828 = ct{302};
t1829 = ct{303};
t183 = ct{304};
t1831 = ct{305};
t1833 = ct{306};
t1834 = ct{307};
t1835 = ct{308};
t1836 = ct{309};
t1839 = ct{310};
t1847 = ct{311};
t1849 = ct{312};
t185 = ct{313};
t1855 = ct{314};
t1856 = ct{315};
t1858 = ct{316};
t1860 = ct{317};
t1861 = ct{318};
t1863 = ct{319};
t1868 = ct{320};
t1870 = ct{321};
t1873 = ct{322};
t1878 = ct{323};
t1882 = ct{324};
t1884 = ct{325};
t1886 = ct{326};
t1892 = ct{327};
t1896 = ct{328};
t1899 = ct{329};
t19 = ct{330};
t190 = ct{331};
t1900 = ct{332};
t1902 = ct{333};
t1906 = ct{334};
t1908 = ct{335};
t1909 = ct{336};
t191 = ct{337};
t1913 = ct{338};
t1916 = ct{339};
t1917 = ct{340};
t1922 = ct{341};
t1925 = ct{342};
t1930 = ct{343};
t1937 = ct{344};
t1938 = ct{345};
t1941 = ct{346};
t1942 = ct{347};
t1946 = ct{348};
t1947 = ct{349};
t1951 = ct{350};
t1952 = ct{351};
t196 = ct{352};
t1961 = ct{353};
t1967 = ct{354};
t1968 = ct{355};
t1969 = ct{356};
t197 = ct{357};
t1974 = ct{358};
t1977 = ct{359};
t1981 = ct{360};
t1983 = ct{361};
t1984 = ct{362};
t1985 = ct{363};
t1986 = ct{364};
t1989 = ct{365};
t199 = ct{366};
t1992 = ct{367};
t1993 = ct{368};
t1995 = ct{369};
t1997 = ct{370};
t1998 = ct{371};
t1999 = ct{372};
t2 = ct{373};
t20 = ct{374};
t200 = ct{375};
t2002 = ct{376};
t2003 = ct{377};
t2004 = ct{378};
t2006 = ct{379};
t2008 = ct{380};
t201 = ct{381};
t2014 = ct{382};
t2015 = ct{383};
t2017 = ct{384};
t202 = ct{385};
t2026 = ct{386};
t2027 = ct{387};
t2028 = ct{388};
t2034 = ct{389};
t2035 = ct{390};
t2036 = ct{391};
t2038 = ct{392};
t2039 = ct{393};
t2043 = ct{394};
t2047 = ct{395};
t2050 = ct{396};
t2052 = ct{397};
t2053 = ct{398};
t206 = ct{399};
t2060 = ct{400};
t2062 = ct{401};
t2066 = ct{402};
t2068 = ct{403};
t2069 = ct{404};
t207 = ct{405};
t2070 = ct{406};
t2075 = ct{407};
t2076 = ct{408};
t2077 = ct{409};
t2079 = ct{410};
t2081 = ct{411};
t2083 = ct{412};
t2085 = ct{413};
t2088 = ct{414};
t2091 = ct{415};
t2096 = ct{416};
t2098 = ct{417};
t21 = ct{418};
t2100 = ct{419};
t2106 = ct{420};
t2110 = ct{421};
t2113 = ct{422};
t2115 = ct{423};
t2116 = ct{424};
t2118 = ct{425};
t2119 = ct{426};
t2121 = ct{427};
t2123 = ct{428};
t2128 = ct{429};
t2130 = ct{430};
t2132 = ct{431};
t2133 = ct{432};
t2134 = ct{433};
t2136 = ct{434};
t2142 = ct{435};
t2143 = ct{436};
t2145 = ct{437};
t2149 = ct{438};
t2150 = ct{439};
t2154 = ct{440};
t2158 = ct{441};
t2164 = ct{442};
t2165 = ct{443};
t2176 = ct{444};
t2177 = ct{445};
t2178 = ct{446};
t2180 = ct{447};
t2181 = ct{448};
t2184 = ct{449};
t2186 = ct{450};
t2187 = ct{451};
t2189 = ct{452};
t2191 = ct{453};
t2192 = ct{454};
t2193 = ct{455};
t2196 = ct{456};
t2197 = ct{457};
t2199 = ct{458};
t22 = ct{459};
t2200 = ct{460};
t2202 = ct{461};
t2203 = ct{462};
t2208 = ct{463};
t2211 = ct{464};
t2213 = ct{465};
t2214 = ct{466};
t2217 = ct{467};
t2220 = ct{468};
t2223 = ct{469};
t2224 = ct{470};
t2234 = ct{471};
t2236 = ct{472};
t2239 = ct{473};
t224 = ct{474};
t2243 = ct{475};
t225 = ct{476};
t2253 = ct{477};
t2256 = ct{478};
t2257 = ct{479};
t2266 = ct{480};
t2267 = ct{481};
t227 = ct{482};
t228 = ct{483};
t2284 = ct{484};
t2289 = ct{485};
t2291 = ct{486};
t2296 = ct{487};
t2298 = ct{488};
t2299 = ct{489};
t23 = ct{490};
t230 = ct{491};
t2300 = ct{492};
t2303 = ct{493};
t2304 = ct{494};
t231 = ct{495};
t2312 = ct{496};
t2314 = ct{497};
t2315 = ct{498};
t2320 = ct{499};
t2326 = ct{500};
t2328 = ct{501};
t233 = ct{502};
t2330 = ct{503};
t2333 = ct{504};
t2334 = ct{505};
t2338 = ct{506};
t234 = ct{507};
t2341 = ct{508};
t2342 = ct{509};
t235 = ct{510};
t2358 = ct{511};
t2359 = ct{512};
t236 = ct{513};
t2362 = ct{514};
t2364 = ct{515};
t2383 = ct{516};
t2390 = ct{517};
t2392 = ct{518};
t2395 = ct{519};
t2396 = ct{520};
t2397 = ct{521};
t2398 = ct{522};
t24 = ct{523};
t240 = ct{524};
t2416 = ct{525};
t2420 = ct{526};
t2421 = ct{527};
t2424 = ct{528};
t243 = ct{529};
t2435 = ct{530};
t2439 = ct{531};
t244 = ct{532};
t2443 = ct{533};
t2444 = ct{534};
t2449 = ct{535};
t2452 = ct{536};
t2454 = ct{537};
t2465 = ct{538};
t2466 = ct{539};
t2474 = ct{540};
t2481 = ct{541};
t2483 = ct{542};
t2486 = ct{543};
t249 = ct{544};
t2490 = ct{545};
t2494 = ct{546};
t2497 = ct{547};
t2502 = ct{548};
t2507 = ct{549};
t2523 = ct{550};
t2524 = ct{551};
t2525 = ct{552};
t2530 = ct{553};
t2539 = ct{554};
t2544 = ct{555};
t2546 = ct{556};
t2548 = ct{557};
t2549 = ct{558};
t2552 = ct{559};
t2553 = ct{560};
t2554 = ct{561};
t2555 = ct{562};
t2556 = ct{563};
t2560 = ct{564};
t2562 = ct{565};
t2563 = ct{566};
t2564 = ct{567};
t2565 = ct{568};
t2566 = ct{569};
t2567 = ct{570};
t2568 = ct{571};
t2569 = ct{572};
t257 = ct{573};
t2570 = ct{574};
t2571 = ct{575};
t2574 = ct{576};
t2575 = ct{577};
t2576 = ct{578};
t2577 = ct{579};
t2578 = ct{580};
t2579 = ct{581};
t258 = ct{582};
t2588 = ct{583};
t2589 = ct{584};
t2597 = ct{585};
t2598 = ct{586};
t2599 = ct{587};
t2611 = ct{588};
t2612 = ct{589};
t2615 = ct{590};
t2617 = ct{591};
t2627 = ct{592};
t263 = ct{593};
t2640 = ct{594};
t2641 = ct{595};
t2655 = ct{596};
t2656 = ct{597};
t266 = ct{598};
t2666 = ct{599};
t2684 = ct{600};
t2686 = ct{601};
t2689 = ct{602};
t2692 = ct{603};
t2694 = ct{604};
t2695 = ct{605};
t270 = ct{606};
t2706 = ct{607};
t2720 = ct{608};
t2722 = ct{609};
t2724 = ct{610};
t2725 = ct{611};
t2726 = ct{612};
t273 = ct{613};
t2737 = ct{614};
t274 = ct{615};
t2740 = ct{616};
t2741 = ct{617};
t2743 = ct{618};
t2744 = ct{619};
t2748 = ct{620};
t2749 = ct{621};
t275 = ct{622};
t2750 = ct{623};
t2752 = ct{624};
t2753 = ct{625};
t2754 = ct{626};
t2755 = ct{627};
t2757 = ct{628};
t2759 = ct{629};
t276 = ct{630};
t2760 = ct{631};
t2761 = ct{632};
t2764 = ct{633};
t277 = ct{634};
t2771 = ct{635};
t2772 = ct{636};
t2775 = ct{637};
t2778 = ct{638};
t278 = ct{639};
t2780 = ct{640};
t2783 = ct{641};
t2785 = ct{642};
t2791 = ct{643};
t2792 = ct{644};
t2793 = ct{645};
t2795 = ct{646};
t2797 = ct{647};
t2798 = ct{648};
t2799 = ct{649};
t280 = ct{650};
t2800 = ct{651};
t2801 = ct{652};
t2802 = ct{653};
t2805 = ct{654};
t2806 = ct{655};
t2807 = ct{656};
t2812 = ct{657};
t2815 = ct{658};
t2816 = ct{659};
t2817 = ct{660};
t2818 = ct{661};
t2824 = ct{662};
t2825 = ct{663};
t2827 = ct{664};
t2833 = ct{665};
t2835 = ct{666};
t284 = ct{667};
t2851 = ct{668};
t2857 = ct{669};
t2861 = ct{670};
t2868 = ct{671};
t287 = ct{672};
t2872 = ct{673};
t2877 = ct{674};
t2880 = ct{675};
t2881 = ct{676};
t2887 = ct{677};
t2889 = ct{678};
t2893 = ct{679};
t2895 = ct{680};
t2896 = ct{681};
t29 = ct{682};
t290 = ct{683};
t2905 = ct{684};
t2906 = ct{685};
t291 = ct{686};
t2911 = ct{687};
t2913 = ct{688};
t2915 = ct{689};
t2916 = ct{690};
t2918 = ct{691};
t292 = ct{692};
t2921 = ct{693};
t2922 = ct{694};
t2932 = ct{695};
t2933 = ct{696};
t294 = ct{697};
t2941 = ct{698};
t2944 = ct{699};
t2956 = ct{700};
t2958 = ct{701};
t2965 = ct{702};
t297 = ct{703};
t2973 = ct{704};
t2977 = ct{705};
t2987 = ct{706};
t299 = ct{707};
t2999 = ct{708};
t3 = ct{709};
t30 = ct{710};
t300 = ct{711};
t302 = ct{712};
t303 = ct{713};
t304 = ct{714};
t3047 = ct{715};
t305 = ct{716};
t306 = ct{717};
t3065 = ct{718};
t3080 = ct{719};
t3083 = ct{720};
t3088 = ct{721};
t309 = ct{722};
t3095 = ct{723};
t3096 = ct{724};
t310 = ct{725};
t311 = ct{726};
t3117 = ct{727};
t3125 = ct{728};
t3129 = ct{729};
t313 = ct{730};
t3136 = ct{731};
t314 = ct{732};
t3142 = ct{733};
t315 = ct{734};
t3159 = ct{735};
t316 = ct{736};
t3164 = ct{737};
t3166 = ct{738};
t3168 = ct{739};
t318 = ct{740};
t319 = ct{741};
t320 = ct{742};
t3200 = ct{743};
t3209 = ct{744};
t3213 = ct{745};
t3219 = ct{746};
t322 = ct{747};
t3222 = ct{748};
t3224 = ct{749};
t3230 = ct{750};
t3239 = ct{751};
t324 = ct{752};
t3247 = ct{753};
t325 = ct{754};
t3266 = ct{755};
t3268 = ct{756};
t3274 = ct{757};
t328 = ct{758};
t3309 = ct{759};
t3321 = ct{760};
t333 = ct{761};
t3338 = ct{762};
t336 = ct{763};
t3365 = ct{764};
t3368 = ct{765};
t3369 = ct{766};
t337 = ct{767};
t3371 = ct{768};
t3375 = ct{769};
t3378 = ct{770};
t3380 = ct{771};
t3383 = ct{772};
t3387 = ct{773};
t3390 = ct{774};
t3391 = ct{775};
t3392 = ct{776};
t3397 = ct{777};
t34 = ct{778};
t340 = ct{779};
t3400 = ct{780};
t3405 = ct{781};
t3407 = ct{782};
t3409 = ct{783};
t3416 = ct{784};
t3417 = ct{785};
t3418 = ct{786};
t3420 = ct{787};
t3421 = ct{788};
t3422 = ct{789};
t3426 = ct{790};
t3429 = ct{791};
t3430 = ct{792};
t3432 = ct{793};
t3434 = ct{794};
t3435 = ct{795};
t3436 = ct{796};
t3437 = ct{797};
t3439 = ct{798};
t344 = ct{799};
t3440 = ct{800};
t3441 = ct{801};
t3443 = ct{802};
t3444 = ct{803};
t3445 = ct{804};
t3446 = ct{805};
t3449 = ct{806};
t3450 = ct{807};
t3453 = ct{808};
t3457 = ct{809};
t3458 = ct{810};
t346 = ct{811};
t3462 = ct{812};
t3463 = ct{813};
t3464 = ct{814};
t3465 = ct{815};
t3468 = ct{816};
t3469 = ct{817};
t347 = ct{818};
t3471 = ct{819};
t3472 = ct{820};
t3474 = ct{821};
t3475 = ct{822};
t3476 = ct{823};
t3479 = ct{824};
t348 = ct{825};
t3480 = ct{826};
t3483 = ct{827};
t3485 = ct{828};
t3489 = ct{829};
t349 = ct{830};
t3490 = ct{831};
t3491 = ct{832};
t3492 = ct{833};
t3493 = ct{834};
t3496 = ct{835};
t3498 = ct{836};
t3499 = ct{837};
t350 = ct{838};
t3500 = ct{839};
t3501 = ct{840};
t3504 = ct{841};
t3506 = ct{842};
t3507 = ct{843};
t3510 = ct{844};
t3511 = ct{845};
t3513 = ct{846};
t3514 = ct{847};
t3515 = ct{848};
t3517 = ct{849};
t3518 = ct{850};
t352 = ct{851};
t3521 = ct{852};
t3522 = ct{853};
t3523 = ct{854};
t3526 = ct{855};
t353 = ct{856};
t3530 = ct{857};
t3531 = ct{858};
t3532 = ct{859};
t3535 = ct{860};
t3536 = ct{861};
t3539 = ct{862};
t3540 = ct{863};
t3542 = ct{864};
t3543 = ct{865};
t3547 = ct{866};
t3554 = ct{867};
t3556 = ct{868};
t3557 = ct{869};
t356 = ct{870};
t3562 = ct{871};
t3565 = ct{872};
t3568 = ct{873};
t3569 = ct{874};
t357 = ct{875};
t3571 = ct{876};
t3572 = ct{877};
t3574 = ct{878};
t3577 = ct{879};
t3578 = ct{880};
t358 = ct{881};
t3582 = ct{882};
t3583 = ct{883};
t3584 = ct{884};
t3585 = ct{885};
t359 = ct{886};
t3592 = ct{887};
t3593 = ct{888};
t3605 = ct{889};
t3606 = ct{890};
t3607 = ct{891};
t361 = ct{892};
t3610 = ct{893};
t3611 = ct{894};
t3612 = ct{895};
t3617 = ct{896};
t3618 = ct{897};
t362 = ct{898};
t3634 = ct{899};
t3635 = ct{900};
t3637 = ct{901};
t3640 = ct{902};
t3642 = ct{903};
t3644 = ct{904};
t3648 = ct{905};
t365 = ct{906};
t3656 = ct{907};
t3658 = ct{908};
t3659 = ct{909};
t3662 = ct{910};
t3666 = ct{911};
t3667 = ct{912};
t3668 = ct{913};
t3672 = ct{914};
t3673 = ct{915};
t3676 = ct{916};
t3678 = ct{917};
t368 = ct{918};
t3682 = ct{919};
t369 = ct{920};
t3694 = ct{921};
t3702 = ct{922};
t3706 = ct{923};
t3708 = ct{924};
t371 = ct{925};
t3717 = ct{926};
t3719 = ct{927};
t372 = ct{928};
t3725 = ct{929};
t3726 = ct{930};
t373 = ct{931};
t3732 = ct{932};
t3733 = ct{933};
t3734 = ct{934};
t3738 = ct{935};
t374 = ct{936};
t3743 = ct{937};
t3746 = ct{938};
t3752 = ct{939};
t3753 = ct{940};
t3754 = ct{941};
t3755 = ct{942};
t3757 = ct{943};
t3759 = ct{944};
t3761 = ct{945};
t3763 = ct{946};
t3764 = ct{947};
t3765 = ct{948};
t3767 = ct{949};
t377 = ct{950};
t3772 = ct{951};
t378 = ct{952};
t3781 = ct{953};
t3783 = ct{954};
t3785 = ct{955};
t3788 = ct{956};
t379 = ct{957};
t3792 = ct{958};
t380 = ct{959};
t3818 = ct{960};
t3819 = ct{961};
t382 = ct{962};
t3821 = ct{963};
t3822 = ct{964};
t3823 = ct{965};
t3824 = ct{966};
t3831 = ct{967};
t3833 = ct{968};
t3835 = ct{969};
t3838 = ct{970};
t384 = ct{971};
t3843 = ct{972};
t3845 = ct{973};
t3851 = ct{974};
t3852 = ct{975};
t3853 = ct{976};
t386 = ct{977};
t3863 = ct{978};
t3869 = ct{979};
t387 = ct{980};
t3871 = ct{981};
t3873 = ct{982};
t3874 = ct{983};
t3875 = ct{984};
t3876 = ct{985};
t388 = ct{986};
t3882 = ct{987};
t3884 = ct{988};
t3889 = ct{989};
t3890 = ct{990};
t3891 = ct{991};
t3892 = ct{992};
t3904 = ct{993};
t3907 = ct{994};
t391 = ct{995};
t3910 = ct{996};
t3913 = ct{997};
t3915 = ct{998};
t392 = ct{999};
t3921 = ct{1000};
t3922 = ct{1001};
t3923 = ct{1002};
t3940 = ct{1003};
t3944 = ct{1004};
t395 = ct{1005};
t3951 = ct{1006};
t3954 = ct{1007};
t3956 = ct{1008};
t3957 = ct{1009};
t3959 = ct{1010};
t396 = ct{1011};
t3960 = ct{1012};
t3968 = ct{1013};
t3969 = ct{1014};
t3971 = ct{1015};
t3972 = ct{1016};
t3976 = ct{1017};
t3978 = ct{1018};
t3979 = ct{1019};
t3992 = ct{1020};
t3993 = ct{1021};
t3995 = ct{1022};
t3997 = ct{1023};
t4 = ct{1024};
t400 = ct{1025};
t4000 = ct{1026};
t4004 = ct{1027};
t4008 = ct{1028};
t401 = ct{1029};
t4010 = ct{1030};
t4011 = ct{1031};
t4014 = ct{1032};
t4015 = ct{1033};
t402 = ct{1034};
t403 = ct{1035};
t4047 = ct{1036};
t4050 = ct{1037};
t4053 = ct{1038};
t4056 = ct{1039};
t406 = ct{1040};
t4069 = ct{1041};
t4070 = ct{1042};
t4083 = ct{1043};
t4086 = ct{1044};
t4089 = ct{1045};
t4099 = ct{1046};
t410 = ct{1047};
t4100 = ct{1048};
t4103 = ct{1049};
t4108 = ct{1050};
t411 = ct{1051};
t4113 = ct{1052};
t4115 = ct{1053};
t4118 = ct{1054};
t4119 = ct{1055};
t412 = ct{1056};
t4121 = ct{1057};
t4123 = ct{1058};
t4126 = ct{1059};
t413 = ct{1060};
t4132 = ct{1061};
t4134 = ct{1062};
t4138 = ct{1063};
t414 = ct{1064};
t4143 = ct{1065};
t4146 = ct{1066};
t4148 = ct{1067};
t4149 = ct{1068};
t415 = ct{1069};
t4152 = ct{1070};
t4153 = ct{1071};
t4154 = ct{1072};
t4158 = ct{1073};
t416 = ct{1074};
t4161 = ct{1075};
t4166 = ct{1076};
t417 = ct{1077};
t4173 = ct{1078};
t4178 = ct{1079};
t4179 = ct{1080};
t418 = ct{1081};
t4181 = ct{1082};
t4183 = ct{1083};
t4185 = ct{1084};
t4186 = ct{1085};
t4190 = ct{1086};
t4196 = ct{1087};
t4197 = ct{1088};
t420 = ct{1089};
t4206 = ct{1090};
t4208 = ct{1091};
t4210 = ct{1092};
t4211 = ct{1093};
t4217 = ct{1094};
t422 = ct{1095};
t4221 = ct{1096};
t4223 = ct{1097};
t4226 = ct{1098};
t4228 = ct{1099};
t423 = ct{1100};
t4230 = ct{1101};
t4232 = ct{1102};
t4234 = ct{1103};
t424 = ct{1104};
t4243 = ct{1105};
t4249 = ct{1106};
t425 = ct{1107};
t4250 = ct{1108};
t4251 = ct{1109};
t4254 = ct{1110};
t4255 = ct{1111};
t4256 = ct{1112};
t4259 = ct{1113};
t4261 = ct{1114};
t4263 = ct{1115};
t427 = ct{1116};
t4274 = ct{1117};
t4276 = ct{1118};
t4278 = ct{1119};
t4279 = ct{1120};
t428 = ct{1121};
t4285 = ct{1122};
t4286 = ct{1123};
t429 = ct{1124};
t4293 = ct{1125};
t4298 = ct{1126};
t4301 = ct{1127};
t4304 = ct{1128};
t4305 = ct{1129};
t4306 = ct{1130};
t431 = ct{1131};
t4315 = ct{1132};
t4317 = ct{1133};
t4318 = ct{1134};
t432 = ct{1135};
t4327 = ct{1136};
t4329 = ct{1137};
t433 = ct{1138};
t4332 = ct{1139};
t4333 = ct{1140};
t4335 = ct{1141};
t4337 = ct{1142};
t4339 = ct{1143};
t434 = ct{1144};
t4342 = ct{1145};
t4344 = ct{1146};
t4345 = ct{1147};
t4347 = ct{1148};
t4348 = ct{1149};
t4349 = ct{1150};
t435 = ct{1151};
t4350 = ct{1152};
t436 = ct{1153};
t4368 = ct{1154};
t4369 = ct{1155};
t437 = ct{1156};
t4370 = ct{1157};
t4371 = ct{1158};
t4378 = ct{1159};
t438 = ct{1160};
t4380 = ct{1161};
t4382 = ct{1162};
t4385 = ct{1163};
t4388 = ct{1164};
t439 = ct{1165};
t4392 = ct{1166};
t4394 = ct{1167};
t4395 = ct{1168};
t4396 = ct{1169};
t4397 = ct{1170};
t44 = ct{1171};
t440 = ct{1172};
t4402 = ct{1173};
t4403 = ct{1174};
t4405 = ct{1175};
t4406 = ct{1176};
t4407 = ct{1177};
t441 = ct{1178};
t4410 = ct{1179};
t4412 = ct{1180};
t4413 = ct{1181};
t4414 = ct{1182};
t4416 = ct{1183};
t4417 = ct{1184};
t4418 = ct{1185};
t4419 = ct{1186};
t442 = ct{1187};
t4420 = ct{1188};
t4423 = ct{1189};
t4425 = ct{1190};
t4426 = ct{1191};
t4427 = ct{1192};
t4428 = ct{1193};
t4429 = ct{1194};
t4431 = ct{1195};
t4436 = ct{1196};
t4437 = ct{1197};
t444 = ct{1198};
t4440 = ct{1199};
t4444 = ct{1200};
t4446 = ct{1201};
t4447 = ct{1202};
t4449 = ct{1203};
t445 = ct{1204};
t4450 = ct{1205};
t4453 = ct{1206};
t4460 = ct{1207};
t4462 = ct{1208};
t4467 = ct{1209};
t4468 = ct{1210};
t4469 = ct{1211};
t4471 = ct{1212};
t4473 = ct{1213};
t4475 = ct{1214};
t4478 = ct{1215};
t4479 = ct{1216};
t448 = ct{1217};
t4482 = ct{1218};
t4483 = ct{1219};
t4485 = ct{1220};
t4486 = ct{1221};
t4487 = ct{1222};
t4488 = ct{1223};
t4489 = ct{1224};
t449 = ct{1225};
t4490 = ct{1226};
t4494 = ct{1227};
t4495 = ct{1228};
t4498 = ct{1229};
t4499 = ct{1230};
t45 = ct{1231};
t450 = ct{1232};
t4500 = ct{1233};
t4501 = ct{1234};
t4502 = ct{1235};
t4505 = ct{1236};
t4506 = ct{1237};
t4509 = ct{1238};
t4510 = ct{1239};
t4515 = ct{1240};
t4518 = ct{1241};
t4519 = ct{1242};
t452 = ct{1243};
t4520 = ct{1244};
t4521 = ct{1245};
t4522 = ct{1246};
t4523 = ct{1247};
t4526 = ct{1248};
t4527 = ct{1249};
t4528 = ct{1250};
t453 = ct{1251};
t4530 = ct{1252};
t4534 = ct{1253};
t4536 = ct{1254};
t4538 = ct{1255};
t454 = ct{1256};
t4541 = ct{1257};
t4543 = ct{1258};
t4545 = ct{1259};
t4546 = ct{1260};
t4549 = ct{1261};
t4551 = ct{1262};
t4552 = ct{1263};
t4553 = ct{1264};
t4556 = ct{1265};
t4557 = ct{1266};
t4558 = ct{1267};
t4559 = ct{1268};
t4565 = ct{1269};
t4568 = ct{1270};
t457 = ct{1271};
t4570 = ct{1272};
t4572 = ct{1273};
t4575 = ct{1274};
t4577 = ct{1275};
t4578 = ct{1276};
t458 = ct{1277};
t4581 = ct{1278};
t4582 = ct{1279};
t4586 = ct{1280};
t4587 = ct{1281};
t4588 = ct{1282};
t4589 = ct{1283};
t459 = ct{1284};
t4590 = ct{1285};
t4591 = ct{1286};
t4592 = ct{1287};
t4593 = ct{1288};
t4595 = ct{1289};
t4596 = ct{1290};
t4597 = ct{1291};
t4598 = ct{1292};
t460 = ct{1293};
t4600 = ct{1294};
t4601 = ct{1295};
t4602 = ct{1296};
t4604 = ct{1297};
t4605 = ct{1298};
t4606 = ct{1299};
t4607 = ct{1300};
t4608 = ct{1301};
t461 = ct{1302};
t4614 = ct{1303};
t4616 = ct{1304};
t4619 = ct{1305};
t462 = ct{1306};
t4621 = ct{1307};
t4622 = ct{1308};
t4623 = ct{1309};
t4624 = ct{1310};
t4625 = ct{1311};
t4626 = ct{1312};
t4629 = ct{1313};
t463 = ct{1314};
t4633 = ct{1315};
t4634 = ct{1316};
t4636 = ct{1317};
t464 = ct{1318};
t4644 = ct{1319};
t4645 = ct{1320};
t4647 = ct{1321};
t4648 = ct{1322};
t465 = ct{1323};
t4654 = ct{1324};
t4656 = ct{1325};
t4659 = ct{1326};
t466 = ct{1327};
t4660 = ct{1328};
t4666 = ct{1329};
t4667 = ct{1330};
t4669 = ct{1331};
t4673 = ct{1332};
t4674 = ct{1333};
t4675 = ct{1334};
t4678 = ct{1335};
t468 = ct{1336};
t4682 = ct{1337};
t4683 = ct{1338};
t4684 = ct{1339};
t469 = ct{1340};
t4694 = ct{1341};
t4695 = ct{1342};
t4696 = ct{1343};
t4697 = ct{1344};
t47 = ct{1345};
t470 = ct{1346};
t4707 = ct{1347};
t4708 = ct{1348};
t471 = ct{1349};
t4714 = ct{1350};
t4717 = ct{1351};
t472 = ct{1352};
t4724 = ct{1353};
t4727 = ct{1354};
t4728 = ct{1355};
t4731 = ct{1356};
t4732 = ct{1357};
t4733 = ct{1358};
t4737 = ct{1359};
t4738 = ct{1360};
t4739 = ct{1361};
t4742 = ct{1362};
t4743 = ct{1363};
t4745 = ct{1364};
t4747 = ct{1365};
t4748 = ct{1366};
t475 = ct{1367};
t4755 = ct{1368};
t4756 = ct{1369};
t4762 = ct{1370};
t4763 = ct{1371};
t477 = ct{1372};
t4773 = ct{1373};
t4775 = ct{1374};
t4780 = ct{1375};
t4781 = ct{1376};
t4782 = ct{1377};
t4783 = ct{1378};
t4785 = ct{1379};
t4786 = ct{1380};
t479 = ct{1381};
t480 = ct{1382};
t4803 = ct{1383};
t481 = ct{1384};
t4810 = ct{1385};
t4811 = ct{1386};
t482 = ct{1387};
t4824 = ct{1388};
t4825 = ct{1389};
t4826 = ct{1390};
t483 = ct{1391};
t4837 = ct{1392};
t4838 = ct{1393};
t4842 = ct{1394};
t4846 = ct{1395};
t485 = ct{1396};
t486 = ct{1397};
t4862 = ct{1398};
t4864 = ct{1399};
t4866 = ct{1400};
t4867 = ct{1401};
t4869 = ct{1402};
t4870 = ct{1403};
t488 = ct{1404};
t4884 = ct{1405};
t489 = ct{1406};
t4903 = ct{1407};
t4904 = ct{1408};
t491 = ct{1409};
t4911 = ct{1410};
t4914 = ct{1411};
t4919 = ct{1412};
t492 = ct{1413};
t4920 = ct{1414};
t4924 = ct{1415};
t4925 = ct{1416};
t4927 = ct{1417};
t4929 = ct{1418};
t493 = ct{1419};
t4934 = ct{1420};
t4936 = ct{1421};
t494 = ct{1422};
t4942 = ct{1423};
t4946 = ct{1424};
t4949 = ct{1425};
t4950 = ct{1426};
t4953 = ct{1427};
t4957 = ct{1428};
t496 = ct{1429};
t4964 = ct{1430};
t497 = ct{1431};
t4973 = ct{1432};
t4974 = ct{1433};
t498 = ct{1434};
t4981 = ct{1435};
t4983 = ct{1436};
t4984 = ct{1437};
t4987 = ct{1438};
t4988 = ct{1439};
t4989 = ct{1440};
t499 = ct{1441};
t4990 = ct{1442};
t4993 = ct{1443};
t4994 = ct{1444};
t4995 = ct{1445};
t4996 = ct{1446};
t5 = ct{1447};
t50 = ct{1448};
t500 = ct{1449};
t5000 = ct{1450};
t5002 = ct{1451};
t5007 = ct{1452};
t5008 = ct{1453};
t5009 = ct{1454};
t501 = ct{1455};
t5017 = ct{1456};
t502 = ct{1457};
t5020 = ct{1458};
t5021 = ct{1459};
t5022 = ct{1460};
t5023 = ct{1461};
t5024 = ct{1462};
t5026 = ct{1463};
t5027 = ct{1464};
t503 = ct{1465};
t5031 = ct{1466};
t5032 = ct{1467};
t5039 = ct{1468};
t504 = ct{1469};
t505 = ct{1470};
t5056 = ct{1471};
t5058 = ct{1472};
t506 = ct{1473};
t5061 = ct{1474};
t5063 = ct{1475};
t5064 = ct{1476};
t5065 = ct{1477};
t507 = ct{1478};
t5075 = ct{1479};
t5076 = ct{1480};
t508 = ct{1481};
t5080 = ct{1482};
t5083 = ct{1483};
t5084 = ct{1484};
t5086 = ct{1485};
t5087 = ct{1486};
t509 = ct{1487};
t5090 = ct{1488};
t5091 = ct{1489};
t5093 = ct{1490};
t5097 = ct{1491};
t5099 = ct{1492};
t510 = ct{1493};
t5100 = ct{1494};
t5102 = ct{1495};
t5107 = ct{1496};
t511 = ct{1497};
t5112 = ct{1498};
t5113 = ct{1499};
t5114 = ct{1500};
t512 = ct{1501};
t5121 = ct{1502};
t5123 = ct{1503};
t513 = ct{1504};
t5132 = ct{1505};
t5136 = ct{1506};
t5139 = ct{1507};
t514 = ct{1508};
t5140 = ct{1509};
t5144 = ct{1510};
t5145 = ct{1511};
t5147 = ct{1512};
t5150 = ct{1513};
t5151 = ct{1514};
t516 = ct{1515};
t5164 = ct{1516};
t5166 = ct{1517};
t517 = ct{1518};
t518 = ct{1519};
t5184 = ct{1520};
t5189 = ct{1521};
t5195 = ct{1522};
t520 = ct{1523};
t5202 = ct{1524};
t5203 = ct{1525};
t5204 = ct{1526};
t5206 = ct{1527};
t521 = ct{1528};
t5210 = ct{1529};
t5211 = ct{1530};
t5215 = ct{1531};
t5217 = ct{1532};
t5219 = ct{1533};
t522 = ct{1534};
t5227 = ct{1535};
t5228 = ct{1536};
t523 = ct{1537};
t5232 = ct{1538};
t5233 = ct{1539};
t5235 = ct{1540};
t5236 = ct{1541};
t5238 = ct{1542};
t524 = ct{1543};
t5242 = ct{1544};
t5244 = ct{1545};
t5249 = ct{1546};
t525 = ct{1547};
t5251 = ct{1548};
t5252 = ct{1549};
t5255 = ct{1550};
t5258 = ct{1551};
t5259 = ct{1552};
t526 = ct{1553};
t5260 = ct{1554};
t5262 = ct{1555};
t5269 = ct{1556};
t527 = ct{1557};
t5275 = ct{1558};
t5279 = ct{1559};
t528 = ct{1560};
t5280 = ct{1561};
t5285 = ct{1562};
t529 = ct{1563};
t5297 = ct{1564};
t53 = ct{1565};
t530 = ct{1566};
t5301 = ct{1567};
t5307 = ct{1568};
t531 = ct{1569};
t5314 = ct{1570};
t5316 = ct{1571};
t5318 = ct{1572};
t532 = ct{1573};
t5320 = ct{1574};
t5323 = ct{1575};
t5324 = ct{1576};
t533 = ct{1577};
t5333 = ct{1578};
t5335 = ct{1579};
t5337 = ct{1580};
t5339 = ct{1581};
t534 = ct{1582};
t5340 = ct{1583};
t5344 = ct{1584};
t535 = ct{1585};
t5354 = ct{1586};
t5356 = ct{1587};
t536 = ct{1588};
t5364 = ct{1589};
t537 = ct{1590};
t5370 = ct{1591};
t5372 = ct{1592};
t5373 = ct{1593};
t5375 = ct{1594};
t5378 = ct{1595};
t538 = ct{1596};
t5383 = ct{1597};
t5389 = ct{1598};
t539 = ct{1599};
t5390 = ct{1600};
t5391 = ct{1601};
t5392 = ct{1602};
t5393 = ct{1603};
t5394 = ct{1604};
t5395 = ct{1605};
t540 = ct{1606};
t5402 = ct{1607};
t5404 = ct{1608};
t5405 = ct{1609};
t5409 = ct{1610};
t5412 = ct{1611};
t5416 = ct{1612};
t5422 = ct{1613};
t5423 = ct{1614};
t543 = ct{1615};
t5431 = ct{1616};
t544 = ct{1617};
t5443 = ct{1618};
t5447 = ct{1619};
t545 = ct{1620};
t5450 = ct{1621};
t5457 = ct{1622};
t5459 = ct{1623};
t546 = ct{1624};
t5464 = ct{1625};
t5465 = ct{1626};
t5466 = ct{1627};
t547 = ct{1628};
t548 = ct{1629};
t5480 = ct{1630};
t5482 = ct{1631};
t5483 = ct{1632};
t5484 = ct{1633};
t5486 = ct{1634};
t5487 = ct{1635};
t5488 = ct{1636};
t549 = ct{1637};
t5507 = ct{1638};
t551 = ct{1639};
t5515 = ct{1640};
t552 = ct{1641};
t5521 = ct{1642};
t553 = ct{1643};
t554 = ct{1644};
t555 = ct{1645};
t556 = ct{1646};
t557 = ct{1647};
t558 = ct{1648};
t559 = ct{1649};
t560 = ct{1650};
t5602 = ct{1651};
t5605 = ct{1652};
t561 = ct{1653};
t5616 = ct{1654};
t5617 = ct{1655};
t5619 = ct{1656};
t562 = ct{1657};
t5620 = ct{1658};
t5621 = ct{1659};
t5622 = ct{1660};
t5623 = ct{1661};
t5626 = ct{1662};
t5628 = ct{1663};
t563 = ct{1664};
t5633 = ct{1665};
t5634 = ct{1666};
t5636 = ct{1667};
t5638 = ct{1668};
t5639 = ct{1669};
t564 = ct{1670};
t5642 = ct{1671};
t5644 = ct{1672};
t5645 = ct{1673};
t5646 = ct{1674};
t5647 = ct{1675};
t5648 = ct{1676};
t5650 = ct{1677};
t5652 = ct{1678};
t5654 = ct{1679};
t5655 = ct{1680};
t5657 = ct{1681};
t5658 = ct{1682};
t5662 = ct{1683};
t5665 = ct{1684};
t5666 = ct{1685};
t567 = ct{1686};
t5670 = ct{1687};
t5676 = ct{1688};
t5677 = ct{1689};
t5679 = ct{1690};
t568 = ct{1691};
t5683 = ct{1692};
t5684 = ct{1693};
t5685 = ct{1694};
t5688 = ct{1695};
t569 = ct{1696};
t5691 = ct{1697};
t5694 = ct{1698};
t5699 = ct{1699};
t57 = ct{1700};
t570 = ct{1701};
t5700 = ct{1702};
t5702 = ct{1703};
t5704 = ct{1704};
t5706 = ct{1705};
t5708 = ct{1706};
t5709 = ct{1707};
t571 = ct{1708};
t5710 = ct{1709};
t5717 = ct{1710};
t5718 = ct{1711};
t572 = ct{1712};
t5729 = ct{1713};
t573 = ct{1714};
t5730 = ct{1715};
t5735 = ct{1716};
t5738 = ct{1717};
t5739 = ct{1718};
t574 = ct{1719};
t5740 = ct{1720};
t5742 = ct{1721};
t5744 = ct{1722};
t5750 = ct{1723};
t5752 = ct{1724};
t5755 = ct{1725};
t5756 = ct{1726};
t5757 = ct{1727};
t576 = ct{1728};
t5761 = ct{1729};
t5762 = ct{1730};
t5766 = ct{1731};
t5769 = ct{1732};
t5770 = ct{1733};
t5771 = ct{1734};
t5772 = ct{1735};
t5774 = ct{1736};
t5775 = ct{1737};
t5776 = ct{1738};
t5778 = ct{1739};
t5779 = ct{1740};
t578 = ct{1741};
t5783 = ct{1742};
t5784 = ct{1743};
t5786 = ct{1744};
t5787 = ct{1745};
t5790 = ct{1746};
t5791 = ct{1747};
t5792 = ct{1748};
t5794 = ct{1749};
t5795 = ct{1750};
t5797 = ct{1751};
t5798 = ct{1752};
t5799 = ct{1753};
t58 = ct{1754};
t580 = ct{1755};
t5800 = ct{1756};
t5802 = ct{1757};
t5805 = ct{1758};
t5808 = ct{1759};
t5809 = ct{1760};
t581 = ct{1761};
t5810 = ct{1762};
t582 = ct{1763};
t5822 = ct{1764};
t5823 = ct{1765};
t5824 = ct{1766};
t5825 = ct{1767};
t5826 = ct{1768};
t5827 = ct{1769};
t5828 = ct{1770};
t5829 = ct{1771};
t5830 = ct{1772};
t5831 = ct{1773};
t5832 = ct{1774};
t5833 = ct{1775};
t5834 = ct{1776};
t5835 = ct{1777};
t5836 = ct{1778};
t5838 = ct{1779};
t5839 = ct{1780};
t584 = ct{1781};
t5840 = ct{1782};
t5841 = ct{1783};
t5842 = ct{1784};
t5843 = ct{1785};
t5844 = ct{1786};
t5845 = ct{1787};
t5846 = ct{1788};
t5847 = ct{1789};
t5848 = ct{1790};
t5849 = ct{1791};
t5850 = ct{1792};
t5851 = ct{1793};
t5852 = ct{1794};
t5859 = ct{1795};
t586 = ct{1796};
t5861 = ct{1797};
t5862 = ct{1798};
t5863 = ct{1799};
t5864 = ct{1800};
t587 = ct{1801};
t5870 = ct{1802};
t5872 = ct{1803};
t5873 = ct{1804};
t5874 = ct{1805};
t5878 = ct{1806};
t5879 = ct{1807};
t5880 = ct{1808};
t5881 = ct{1809};
t5882 = ct{1810};
t5883 = ct{1811};
t5884 = ct{1812};
t5885 = ct{1813};
t5888 = ct{1814};
t5889 = ct{1815};
t589 = ct{1816};
t5890 = ct{1817};
t5891 = ct{1818};
t5892 = ct{1819};
t5893 = ct{1820};
t5894 = ct{1821};
t5895 = ct{1822};
t5897 = ct{1823};
t5898 = ct{1824};
t5899 = ct{1825};
t590 = ct{1826};
t5900 = ct{1827};
t5901 = ct{1828};
t5904 = ct{1829};
t5905 = ct{1830};
t5907 = ct{1831};
t5909 = ct{1832};
t591 = ct{1833};
t5911 = ct{1834};
t5912 = ct{1835};
t5914 = ct{1836};
t5915 = ct{1837};
t5916 = ct{1838};
t5917 = ct{1839};
t5918 = ct{1840};
t5919 = ct{1841};
t592 = ct{1842};
t5920 = ct{1843};
t5922 = ct{1844};
t5925 = ct{1845};
t5926 = ct{1846};
t5928 = ct{1847};
t5929 = ct{1848};
t593 = ct{1849};
t5930 = ct{1850};
t5931 = ct{1851};
t5932 = ct{1852};
t5933 = ct{1853};
t5934 = ct{1854};
t5935 = ct{1855};
t5936 = ct{1856};
t5937 = ct{1857};
t5938 = ct{1858};
t5939 = ct{1859};
t594 = ct{1860};
t5940 = ct{1861};
t5941 = ct{1862};
t5942 = ct{1863};
t5943 = ct{1864};
t5944 = ct{1865};
t5945 = ct{1866};
t5946 = ct{1867};
t5947 = ct{1868};
t5948 = ct{1869};
t5949 = ct{1870};
t595 = ct{1871};
t5951 = ct{1872};
t5952 = ct{1873};
t5954 = ct{1874};
t5956 = ct{1875};
t5957 = ct{1876};
t5958 = ct{1877};
t5959 = ct{1878};
t596 = ct{1879};
t5960 = ct{1880};
t5961 = ct{1881};
t5962 = ct{1882};
t5964 = ct{1883};
t5965 = ct{1884};
t5966 = ct{1885};
t5967 = ct{1886};
t5968 = ct{1887};
t597 = ct{1888};
t5970 = ct{1889};
t5971 = ct{1890};
t5972 = ct{1891};
t5973 = ct{1892};
t5974 = ct{1893};
t5975 = ct{1894};
t5976 = ct{1895};
t5977 = ct{1896};
t5978 = ct{1897};
t5979 = ct{1898};
t5980 = ct{1899};
t5981 = ct{1900};
t5982 = ct{1901};
t5983 = ct{1902};
t5984 = ct{1903};
t5985 = ct{1904};
t5986 = ct{1905};
t5988 = ct{1906};
t5991 = ct{1907};
t5992 = ct{1908};
t5994 = ct{1909};
t5995 = ct{1910};
t5996 = ct{1911};
t5997 = ct{1912};
t5998 = ct{1913};
t5999 = ct{1914};
t6 = ct{1915};
t60 = ct{1916};
t600 = ct{1917};
t6000 = ct{1918};
t6001 = ct{1919};
t6002 = ct{1920};
t6003 = ct{1921};
t6004 = ct{1922};
t6005 = ct{1923};
t6007 = ct{1924};
t6008 = ct{1925};
t6009 = ct{1926};
t6010 = ct{1927};
t6011 = ct{1928};
t6012 = ct{1929};
t6013 = ct{1930};
t6014 = ct{1931};
t6016 = ct{1932};
t6017 = ct{1933};
t6018 = ct{1934};
t6019 = ct{1935};
t602 = ct{1936};
t6020 = ct{1937};
t6021 = ct{1938};
t6024 = ct{1939};
t6026 = ct{1940};
t6028 = ct{1941};
t6029 = ct{1942};
t603 = ct{1943};
t6030 = ct{1944};
t6032 = ct{1945};
t6033 = ct{1946};
t6034 = ct{1947};
t6035 = ct{1948};
t6037 = ct{1949};
t6038 = ct{1950};
t604 = ct{1951};
t6042 = ct{1952};
t6043 = ct{1953};
t6045 = ct{1954};
t6046 = ct{1955};
t6047 = ct{1956};
t6048 = ct{1957};
t6049 = ct{1958};
t605 = ct{1959};
t6051 = ct{1960};
t6052 = ct{1961};
t6053 = ct{1962};
t6054 = ct{1963};
t6055 = ct{1964};
t6056 = ct{1965};
t6057 = ct{1966};
t6059 = ct{1967};
t6060 = ct{1968};
t6061 = ct{1969};
t6062 = ct{1970};
t6064 = ct{1971};
t6065 = ct{1972};
t6067 = ct{1973};
t6068 = ct{1974};
t6069 = ct{1975};
t6073 = ct{1976};
t6074 = ct{1977};
t6075 = ct{1978};
t6076 = ct{1979};
t6077 = ct{1980};
t6078 = ct{1981};
t6079 = ct{1982};
t6081 = ct{1983};
t6082 = ct{1984};
t6083 = ct{1985};
t6084 = ct{1986};
t6085 = ct{1987};
t6086 = ct{1988};
t6087 = ct{1989};
t6088 = ct{1990};
t6089 = ct{1991};
t609 = ct{1992};
t6090 = ct{1993};
t6091 = ct{1994};
t6093 = ct{1995};
t6094 = ct{1996};
t6095 = ct{1997};
t6096 = ct{1998};
t6097 = ct{1999};
t610 = ct{2000};
t6103 = ct{2001};
t6105 = ct{2002};
t6106 = ct{2003};
t6108 = ct{2004};
t6109 = ct{2005};
t611 = ct{2006};
t6110 = ct{2007};
t6111 = ct{2008};
t6113 = ct{2009};
t6114 = ct{2010};
t6117 = ct{2011};
t6118 = ct{2012};
t6119 = ct{2013};
t612 = ct{2014};
t6120 = ct{2015};
t6121 = ct{2016};
t6122 = ct{2017};
t6123 = ct{2018};
t6125 = ct{2019};
t6126 = ct{2020};
t6127 = ct{2021};
t6128 = ct{2022};
t6129 = ct{2023};
t613 = ct{2024};
t6130 = ct{2025};
t6131 = ct{2026};
t6132 = ct{2027};
t6134 = ct{2028};
t6135 = ct{2029};
t6136 = ct{2030};
t6137 = ct{2031};
t6139 = ct{2032};
t614 = ct{2033};
t6140 = ct{2034};
t6142 = ct{2035};
t6143 = ct{2036};
t6145 = ct{2037};
t6149 = ct{2038};
t615 = ct{2039};
t6154 = ct{2040};
t6156 = ct{2041};
t6157 = ct{2042};
t616 = ct{2043};
t6161 = ct{2044};
t6163 = ct{2045};
t6165 = ct{2046};
t6166 = ct{2047};
t6167 = ct{2048};
t6168 = ct{2049};
t6169 = ct{2050};
t6170 = ct{2051};
t6171 = ct{2052};
t6174 = ct{2053};
t6175 = ct{2054};
t6178 = ct{2055};
t618 = ct{2056};
t6180 = ct{2057};
t6182 = ct{2058};
t6184 = ct{2059};
t6186 = ct{2060};
t6187 = ct{2061};
t6189 = ct{2062};
t619 = ct{2063};
t6190 = ct{2064};
t6191 = ct{2065};
t6194 = ct{2066};
t6195 = ct{2067};
t6196 = ct{2068};
t6197 = ct{2069};
t6199 = ct{2070};
t620 = ct{2071};
t6200 = ct{2072};
t6201 = ct{2073};
t6202 = ct{2074};
t6203 = ct{2075};
t6204 = ct{2076};
t6205 = ct{2077};
t6206 = ct{2078};
t6207 = ct{2079};
t6208 = ct{2080};
t6209 = ct{2081};
t621 = ct{2082};
t6210 = ct{2083};
t6211 = ct{2084};
t6212 = ct{2085};
t6213 = ct{2086};
t6214 = ct{2087};
t6215 = ct{2088};
t622 = ct{2089};
t6221 = ct{2090};
t6222 = ct{2091};
t6225 = ct{2092};
t6228 = ct{2093};
t6229 = ct{2094};
t623 = ct{2095};
t6230 = ct{2096};
t6231 = ct{2097};
t6232 = ct{2098};
t6233 = ct{2099};
t6234 = ct{2100};
t6235 = ct{2101};
t6239 = ct{2102};
t624 = ct{2103};
t6240 = ct{2104};
t6241 = ct{2105};
t6242 = ct{2106};
t6243 = ct{2107};
t6244 = ct{2108};
t6245 = ct{2109};
t6248 = ct{2110};
t6249 = ct{2111};
t625 = ct{2112};
t6250 = ct{2113};
t6251 = ct{2114};
t6254 = ct{2115};
t6255 = ct{2116};
t6258 = ct{2117};
t6260 = ct{2118};
t6262 = ct{2119};
t6264 = ct{2120};
t6266 = ct{2121};
t6267 = ct{2122};
t6268 = ct{2123};
t6270 = ct{2124};
t6271 = ct{2125};
t6272 = ct{2126};
t6274 = ct{2127};
t6276 = ct{2128};
t6277 = ct{2129};
t6280 = ct{2130};
t6313 = ct{2131};
t6319 = ct{2132};
t632 = ct{2133};
t6320 = ct{2134};
t6329 = ct{2135};
t6330 = ct{2136};
t6331 = ct{2137};
t6332 = ct{2138};
t6333 = ct{2139};
t6336 = ct{2140};
t6338 = ct{2141};
t6341 = ct{2142};
t6342 = ct{2143};
t6343 = ct{2144};
t6345 = ct{2145};
t6347 = ct{2146};
t6348 = ct{2147};
t6349 = ct{2148};
t6350 = ct{2149};
t6351 = ct{2150};
t6352 = ct{2151};
t6353 = ct{2152};
t6354 = ct{2153};
t6355 = ct{2154};
t6356 = ct{2155};
t6360 = ct{2156};
t6361 = ct{2157};
t6362 = ct{2158};
t6364 = ct{2159};
t6365 = ct{2160};
t6366 = ct{2161};
t6367 = ct{2162};
t6368 = ct{2163};
t6369 = ct{2164};
t6374 = ct{2165};
t6375 = ct{2166};
t6376 = ct{2167};
t6378 = ct{2168};
t6379 = ct{2169};
t638 = ct{2170};
t6380 = ct{2171};
t6382 = ct{2172};
t6385 = ct{2173};
t6386 = ct{2174};
t6387 = ct{2175};
t6388 = ct{2176};
t6390 = ct{2177};
t6391 = ct{2178};
t6392 = ct{2179};
t6393 = ct{2180};
t6395 = ct{2181};
t6396 = ct{2182};
t6397 = ct{2183};
t6398 = ct{2184};
t640 = ct{2185};
t6404 = ct{2186};
t6406 = ct{2187};
t6407 = ct{2188};
t6408 = ct{2189};
t6414 = ct{2190};
t6415 = ct{2191};
t6418 = ct{2192};
t6419 = ct{2193};
t6422 = ct{2194};
t6427 = ct{2195};
t6428 = ct{2196};
t6429 = ct{2197};
t6430 = ct{2198};
t6431 = ct{2199};
t6432 = ct{2200};
t6433 = ct{2201};
t6434 = ct{2202};
t6435 = ct{2203};
t6436 = ct{2204};
t6439 = ct{2205};
t6440 = ct{2206};
t6441 = ct{2207};
t6452 = ct{2208};
t6453 = ct{2209};
t6454 = ct{2210};
t6455 = ct{2211};
t6456 = ct{2212};
t6457 = ct{2213};
t6458 = ct{2214};
t6459 = ct{2215};
t6460 = ct{2216};
t6461 = ct{2217};
t6462 = ct{2218};
t6463 = ct{2219};
t6467 = ct{2220};
t6469 = ct{2221};
t6471 = ct{2222};
t6478 = ct{2223};
t6481 = ct{2224};
t6483 = ct{2225};
t6487 = ct{2226};
t6495 = ct{2227};
t6496 = ct{2228};
t6497 = ct{2229};
t6501 = ct{2230};
t6502 = ct{2231};
t6507 = ct{2232};
t6508 = ct{2233};
t6509 = ct{2234};
t6546 = ct{2235};
t6547 = ct{2236};
t6548 = ct{2237};
t6549 = ct{2238};
t6555 = ct{2239};
t6556 = ct{2240};
t6557 = ct{2241};
t6558 = ct{2242};
t6560 = ct{2243};
t6561 = ct{2244};
t6562 = ct{2245};
t6566 = ct{2246};
t6567 = ct{2247};
t6569 = ct{2248};
t6597 = ct{2249};
t6609 = ct{2250};
t6640 = ct{2251};
t6641 = ct{2252};
t6662 = ct{2253};
t6663 = ct{2254};
t6665 = ct{2255};
t6666 = ct{2256};
t6669 = ct{2257};
t6670 = ct{2258};
t6671 = ct{2259};
t6689 = ct{2260};
t6700 = ct{2261};
t6702 = ct{2262};
t6776 = ct{2263};
t681 = ct{2264};
t6826 = ct{2265};
t6827 = ct{2266};
t6832 = ct{2267};
t684 = ct{2268};
t6868 = ct{2269};
t6871 = ct{2270};
t6872 = ct{2271};
t6873 = ct{2272};
t6874 = ct{2273};
t6896 = ct{2274};
t6902 = ct{2275};
t6919 = ct{2276};
